simulink model "CONTROL_01"  (R2018b)
(part 37 of 185)

 I4xy*de1 - I4xy*de1*cos(e2)^2 - I4xy*de1*cos(e3)^2 - 2*I4xy*de1*cos(e4)^2 + (I4xx*de1*sin(2*e4))/2 - (I6xx*de1*sin(2*e4))/2 - (I4yy*de1*sin(2*e4))/2 + (I5yy*de1*sin(2*e4))/2 - (I5zz*de1*sin(2*e4))/2 + (I6zz*de1*sin(2*e4))/2 - I6xy*de1*cos(e5) - I5zx*de1*cos(e5) + I5yz*de1*sin(e5) - I5yz*de1*cos(e2)^2*sin(e5) - I5yz*de1*cos(e3)^2*sin(e5) - 2*I5yz*de1*cos(e4)^2*sin(e5) + de1*m4*x4*y4 - (de1*m4*x4^2*sin(2*e4))/2 + (de1*m6*x6^2*sin(2*e4))/2 + (de1*m4*y4^2*sin(2*e4))/2 - (de1*m5*y5^2*sin(2*e4))/2 + (de1*m5*z5^2*sin(2*e4))/2 - (de1*m6*z6^2*sin(2*e4))/2 + 2*I4xy*de1*cos(e2)^2*cos(e3)^2 + 2*I4xy*de1*cos(e2)^2*cos(e4)^2 + 2*I4xy*de1*cos(e3)^2*cos(e4)^2 - (I4xx*de2*cos(e2)*cos(e3))/2 - (I4xx*de3*cos(e2)*cos(e3))/2 - (I5xx*de2*cos(e2)*cos(e3))/2 - (I5xx*de3*cos(e2)*cos(e3))/2 + (I6xx*de2*cos(e2)*cos(e3))/2 + (I6xx*de3*cos(e2)*cos(e3))/2 + (I4yy*de2*cos(e2)*cos(e3))/2 + (I4yy*de3*cos(e2)*cos(e3))/2 - (I5yy*de2*cos(e2)*cos(e3))/2 - (I5yy*de3*cos(e2)*cos(e3))/2 - (I6yy*de2*cos(e2)*cos(e3))/2 - (I6yy*de3*cos(e2)*cos(e3))/2 - (I4zz*de2*cos(e2)*cos(e3))/2 - (I4zz*de3*cos(e2)*cos(e3))/2 + (I5zz*de2*cos(e2)*cos(e3))/2 + (I5zz*de3*cos(e2)*cos(e3))/2 - (I6zz*de2*cos(e2)*cos(e3))/2 - (I6zz*de3*cos(e2)*cos(e3))/2 - I5xy*de5*cos(e2)*sin(e3) - I5xy*de5*cos(e3)*sin(e2) + I6xy*de6*cos(e2)*sin(e3) + I6xy*de6*cos(e3)*sin(e2) - I6yz*de1*cos(e6)*sin(e5) + (I4xx*de2*sin(e2)*sin(e3))/2 + (I4xx*de3*sin(e2)*sin(e3))/2 + (I5xx*de2*sin(e2)*sin(e3))/2 + (I5xx*de3*sin(e2)*sin(e3))/2 - (I6xx*de2*sin(e2)*sin(e3))/2 - (I6xx*de3*sin(e2)*sin(e3))/2 - (I4yy*de2*sin(e2)*sin(e3))/2 - (I4yy*de3*sin(e2)*sin(e3))/2 + (I5yy*de2*sin(e2)*sin(e3))/2 + (I5yy*de3*sin(e2)*sin(e3))/2 + (I6yy*de2*sin(e2)*sin(e3))/2 + (I6yy*de3*sin(e2)*sin(e3))/2 + (I4zz*de2*sin(e2)*sin(e3))/2 + (I4zz*de3*sin(e2)*sin(e3))/2 - (I5zz*de2*sin(e2)*sin(e3))/2 - (I5zz*de3*sin(e2)*sin(e3))/2 + (I6zz*de2*sin(e2)*sin(e3))/2 + (I6zz*de3*sin(e2)*sin(e3))/2 - I6zx*de1*sin(e5)*sin(e6) + I6xy*de1*cos(e2)^2*cos(e5) + I6xy*de1*cos(e3)^2*cos(e5) + 2*I6xy*de1*cos(e4)^2*cos(e5) + 2*I6xy*de1*cos(e5)*cos(e6)^2 + I5zx*de1*cos(e2)^2*cos(e5) + I5zx*de1*cos(e3)^2*cos(e5) + 2*I5zx*de1*cos(e4)^2*cos(e5) - 2*I6xy*de1*cos(e2)^2*cos(e3)^2*cos(e5) - 2*I6xy*de1*cos(e2)^2*cos(e4)^2*cos(e5) - 2*I6xy*de1*cos(e3)^2*cos(e4)^2*cos(e5) - 2*I6xy*de1*cos(e2)^2*cos(e5)*cos(e6)^2 - 2*I6xy*de1*cos(e3)^2*cos(e5)*cos(e6)^2 - 4*I6xy*de1*cos(e4)^2*cos(e5)*cos(e6)^2 - 2*I5zx*de1*cos(e2)^2*cos(e3)^2*cos(e5) - 2*I5zx*de1*cos(e2)^2*cos(e4)^2*cos(e5) - 2*I5zx*de1*cos(e3)^2*cos(e4)^2*cos(e5) + 2*I5yz*de1*cos(e2)^2*cos(e3)^2*sin(e5) + 2*I5yz*de1*cos(e2)^2*cos(e4)^2*sin(e5) + 2*I5yz*de1*cos(e3)^2*cos(e4)^2*sin(e5) - de1*m4*x4*y4*cos(e2)^2 - de1*m4*x4*y4*cos(e3)^2 - 2*de1*m4*x4*y4*cos(e4)^2 - (I5xx*de5*cos(e2)*cos(e3)*cos(e4))/2 - (I6xx*de5*cos(e2)*cos(e3)*cos(e4))/2 + (I5yy*de5*cos(e2)*cos(e3)*cos(e4))/2 - (I6yy*de5*cos(e2)*cos(e3)*cos(e4))/2 - (I5zz*de5*cos(e2)*cos(e3)*cos(e4))/2 + (I6zz*de5*cos(e2)*cos(e3)*cos(e4))/2 - I5xy*de2*cos(e2)*cos(e4)*sin(e3) - I5xy*de2*cos(e3)*cos(e4)*sin(e2) - I5xy*de3*cos(e2)*cos(e4)*sin(e3) - I5xy*de3*cos(e3)*cos(e4)*sin(e2) - I6xx*de1*cos(e5)*cos(e6)*sin(e6) - I4yz*de1*cos(e2)*cos(e4)*sin(e2) - I4yz*de1*cos(e3)*cos(e4)*sin(e3) + I6yy*de1*cos(e5)*cos(e6)*sin(e6) + I4zx*de2*cos(e2)*cos(e4)*sin(e3) + I4zx*de2*cos(e3)*cos(e4)*sin(e2) + I4zx*de3*cos(e2)*cos(e4)*sin(e3) + I4zx*de3*cos(e3)*cos(e4)*sin(e2) - I6zx*de5*cos(e2)*cos(e6)*sin(e3) - I6zx*de5*cos(e3)*cos(e6)*sin(e2) - 4*I4xy*de1*cos(e2)^2*cos(e3)^2*cos(e4)^2 + I5xy*de1*cos(e2)*sin(e2)*sin(e4) + I5xy*de1*cos(e3)*sin(e3)*sin(e4) + (I5xx*de5*cos(e4)*sin(e2)*sin(e3))/2 + (I6xx*de5*cos(e4)*sin(e2)*sin(e3))/2 - I4yz*de2*cos(e2)*sin(e3)*sin(e4) - I4yz*de2*cos(e3)*sin(e2)*sin(e4) - I4yz*de3*cos(e2)*sin(e3)*sin(e4) - I4yz*de3*cos(e3)*sin(e2)*sin(e4) - (I5yy*de5*cos(e4)*sin(e2)*sin(e3))/2 + (I6yy*de5*cos(e4)*sin(e2)*sin(e3))/2 + I6yz*de5*cos(e2)*sin(e3)*sin(e6) + I6yz*de5*cos(e3)*sin(e2)*sin(e6) - I4zx*de1*cos(e2)*sin(e2)*sin(e4) - I4zx*de1*cos(e3)*sin(e3)*sin(e4) + (I5zz*de5*cos(e4)*sin(e2)*sin(e3))/2 - (I6zz*de5*cos(e4)*sin(e2)*sin(e3))/2 - de2*m6*x6^2*cos(e2)*cos(e3) - de3*m6*x6^2*cos(e2)*cos(e3) - de2*m4*y4^2*cos(e2)*cos(e3) - de3*m4*y4^2*cos(e2)*cos(e3) - de2*m5*z5^2*cos(e2)*cos(e3) - de3*m5*z5^2*cos(e2)*cos(e3) + de2*m6*x6^2*sin(e2)*sin(e3) + de3*m6*x6^2*sin(e2)*sin(e3) + de2*m4*y4^2*sin(e2)*sin(e3) + de3*m4*y4^2*sin(e2)*sin(e3) + de2*m5*z5^2*sin(e2)*sin(e3) + de3*m5*z5^2*sin(e2)*sin(e3) + I4xx*de2*cos(e2)*cos(e3)*cos(e4)^2 + I4xx*de3*cos(e2)*cos(e3)*cos(e4)^2 - I6xx*de2*cos(e2)*cos(e3)*cos(e4)^2 - I6xx*de3*cos(e2)*cos(e3)*cos(e4)^2 - I6xx*de2*cos(e2)*cos(e3)*cos(e6)^2 - I6xx*de3*cos(e2)*cos(e3)*cos(e6)^2 - I4yy*de2*cos(e2)*cos(e3)*cos(e4)^2 - I4yy*de3*cos(e2)*cos(e3)*cos(e4)^2 + I5yy*de2*cos(e2)*cos(e3)*cos(e4)^2 + I5yy*de3*cos(e2)*cos(e3)*cos(e4)^2 + I6yy*de2*cos(e2)*cos(e3)*cos(e6)^2 + I6yy*de3*cos(e2)*cos(e3)*cos(e6)^2 - I5zz*de2*cos(e2)*cos(e3)*cos(e4)^2 - I5zz*de3*cos(e2)*cos(e3)*cos(e4)^2 + I6zz*de2*cos(e2)*cos(e3)*cos(e4)^2 + I6zz*de3*cos(e2)*cos(e3)*cos(e4)^2 - I4xx*de1*cos(e2)^2*cos(e4)*sin(e4) - I4xx*de1*cos(e3)^2*cos(e4)*sin(e4) + I6xx*de1*cos(e2)^2*cos(e4)*sin(e4) + I6xx*de1*cos(e3)^2*cos(e4)*sin(e4) + I5xx*de1*cos(e4)*cos(e5)^2*sin(e4) + 2*I5xy*de5*cos(e2)*cos(e5)^2*sin(e3) + 2*I5xy*de5*cos(e3)*cos(e5)^2*sin(e2) + I6xx*de1*cos(e4)*cos(e6)^2*sin(e4) - I6xy*de6*cos(e2)*cos(e5)^2*sin(e3) - I6xy*de6*cos(e3)*cos(e5)^2*sin(e2) - 2*I6xy*de6*cos(e2)*cos(e6)^2*sin(e3) - 2*I6xy*de6*cos(e3)*cos(e6)^2*sin(e2) + I4yy*de1*cos(e2)^2*cos(e4)*sin(e4) + I4yy*de1*cos(e3)^2*cos(e4)*sin(e4) - I5yy*de1*cos(e2)^2*cos(e4)*sin(e4) - I5yy*de1*cos(e3)^2*cos(e4)*sin(e4) - I5yy*de1*cos(e4)*cos(e5)^2*sin(e4) + I6yy*de1*cos(e4)*cos(e5)^2*sin(e4) - I6yy*de1*cos(e4)*cos(e6)^2*sin(e4) + I6yz*de1*cos(e2)^2*cos(e6)*sin(e5) + I6yz*de1*cos(e3)^2*cos(e6)*sin(e5) + 2*I6yz*de1*cos(e4)^2*cos(e6)*sin(e5) + I5zz*de1*cos(e2)^2*cos(e4)*sin(e4) + I5zz*de1*cos(e3)^2*cos(e4)*sin(e4) - I6zz*de1*cos(e2)^2*cos(e4)*sin(e4) - I6zz*de1*cos(e3)^2*cos(e4)*sin(e4) - I6zz*de1*cos(e4)*cos(e5)^2*sin(e4) - I4xx*de2*cos(e4)^2*sin(e2)*sin(e3) - I4xx*de3*cos(e4)^2*sin(e2)*sin(e3) + I6xx*de2*cos(e4)^2*sin(e2)*sin(e3) + I6xx*de3*cos(e4)^2*sin(e2)*sin(e3) + I6xx*de2*cos(e6)^2*sin(e2)*sin(e3) + I6xx*de3*cos(e6)^2*sin(e2)*sin(e3) + I4yy*de2*cos(e4)^2*sin(e2)*sin(e3) + I4yy*de3*cos(e4)^2*sin(e2)*sin(e3) - I5yy*de2*cos(e4)^2*sin(e2)*sin(e3) - I5yy*de3*cos(e4)^2*sin(e2)*sin(e3) - I6yy*de2*cos(e6)^2*sin(e2)*sin(e3) - I6yy*de3*cos(e6)^2*sin(e2)*sin(e3) + I5zz*de2*cos(e4)^2*sin(e2)*sin(e3) + I5zz*de3*cos(e4)^2*sin(e2)*sin(e3) - I6zz*de2*cos(e4)^2*sin(e2)*sin(e3) + I6zx*de1*cos(e2)^2*sin(e5)*sin(e6) - I6zz*de3*cos(e4)^2*sin(e2)*sin(e3) + I6zx*de1*cos(e3)^2*sin(e5)*sin(e6) + 2*I6zx*de1*cos(e4)^2*sin(e5)*sin(e6) - de1*m6*x6*y6*cos(e5) - de1*m5*x5*z5*cos(e5) + de1*m5*y5*z5*sin(e5) + a3*de1*m4*x4*cos(e2)^2*sin(e4) + a3*de1*m4*x4*cos(e3)^2*sin(e4) - I5xx*de2*cos(e4)^2*cos(e5)^2*sin(e2)*sin(e3) - I5xx*de3*cos(e4)^2*cos(e5)^2*sin(e2)*sin(e3) - I6xx*de2*cos(e4)^2*cos(e6)^2*sin(e2)*sin(e3) - I6xx*de3*cos(e4)^2*cos(e6)^2*sin(e2)*sin(e3) + I5yy*de2*cos(e4)^2*cos(e5)^2*sin(e2)*sin(e3) + I5yy*de3*cos(e4)^2*cos(e5)^2*sin(e2)*sin(e3) - I6yy*de2*cos(e4)^2*cos(e5)^2*sin(e2)*sin(e3) + I6yy*de2*cos(e4)^2*cos(e6)^2*sin(e2)*sin(e3) - I6yy*de3*cos(e4)^2*cos(e5)^2*sin(e2)*sin(e3) + I6yy*de3*cos(e4)^2*cos(e6)^2*sin(e2)*sin(e3) - 2*I6zx*de1*cos(e2)^2*cos(e3)^2*sin(e5)*sin(e6) - 2*I6zx*de1*cos(e2)^2*cos(e4)^2*sin(e5)*sin(e6) + I6zz*de2*cos(e4)^2*cos(e5)^2*sin(e2)*sin(e3) - 2*I6zx*de1*cos(e3)^2*cos(e4)^2*sin(e5)*sin(e6) + I6zz*de3*cos(e4)^2*cos(e5)^2*sin(e2)*sin(e3) + de1*m6*x6*y6*cos(e2)^2*cos(e5) + de1*m6*x6*y6*cos(e3)^2*cos(e5) + 2*de1*m6*x6*y6*cos(e4)^2*cos(e5) + 2*de1*m6*x6*y6*cos(e5)*cos(e6)^2 + de1*m5*x5*z5*cos(e2)^2*cos(e5) + de1*m5*x5*z5*cos(e3)^2*cos(e5) + 2*de1*m5*x5*z5*cos(e4)^2*cos(e5) - de1*m5*y5*z5*cos(e2)^2*sin(e5) - de1*m5*y5*z5*cos(e3)^2*sin(e5) - 2*de1*m5*y5*z5*cos(e4)^2*sin(e5) - I6yz*de6*cos(e2)*cos(e3)*cos(e4)*cos(e6) + 2*I4xy*de2*cos(e2)*cos(e3)*cos(e4)*sin(e4) + 2*I4xy*de3*cos(e2)*cos(e3)*cos(e4)*sin(e4) - 2*I6xy*de2*cos(e2)*cos(e3)*cos(e6)*sin(e6) - I6xy*de5*cos(e2)*cos(e3)*cos(e5)*sin(e4) - 2*I6xy*de3*cos(e2)*cos(e3)*cos(e6)*sin(e6) + I5yz*de1*cos(e2)*cos(e4)*cos(e5)*sin(e2) + I5yz*de1*cos(e3)*cos(e4)*cos(e5)*sin(e3) - I6zx*de2*cos(e2)*cos(e4)*cos(e6)*sin(e3) - I6zx*de2*cos(e3)*cos(e4)*cos(e6)*sin(e2) - I5zx*de5*cos(e2)*cos(e3)*cos(e5)*sin(e4) - I6zx*de3*cos(e2)*cos(e4)*cos(e6)*sin(e3) - I6zx*de3*cos(e3)*cos(e4)*cos(e6)*sin(e2) - I6zx*de6*cos(e2)*cos(e3)*cos(e4)*sin(e6) + 4*I6xy*de1*cos(e2)^2*cos(e3)^2*cos(e4)^2*cos(e5) + 4*I6xy*de1*cos(e2)^2*cos(e3)^2*cos(e5)*cos(e6)^2 + 4*I6xy*de1*cos(e2)^2*cos(e4)^2*cos(e5)*cos(e6)^2 + 4*I6xy*de1*cos(e3)^2*cos(e4)^2*cos(e5)*cos(e6)^2 + 4*I5zx*de1*cos(e2)^2*cos(e3)^2*cos(e4)^2*cos(e5) - 2*I4xy*de1*cos(e2)*cos(e3)*sin(e2)*sin(e3) + I6xy*de1*cos(e2)*cos(e4)*sin(e2)*sin(e5) + I6xy*de1*cos(e3)*cos(e4)*sin(e3)*sin(e5) - I5xx*de5*cos(e2)*cos(e5)*sin(e3)*sin(e5) - I5xx*de5*cos(e3)*cos(e5)*sin(e2)*sin(e5) + 2*I5xy*de1*cos(e4)*cos(e5)*sin(e4)*sin(e5) + (I6xx*de6*cos(e2)*cos(e3)*sin(e4)*sin(e5))/2 + 2*I6xy*de1*cos(e4)*cos(e6)*sin(e4)*sin(e6) + I6xx*de6*cos(e2)*cos(e6)*sin(e3)*sin(e6) + I6xx*de6*cos(e3)*cos(e6)*sin(e2)*sin(e6) + I5yz*de2*cos(e2)*cos(e5)*sin(e3)*sin(e4) + I5yz*de2*cos(e3)*cos(e5)*sin(e2)*sin(e4) + I5yz*de3*cos(e2)*cos(e5)*sin(e3)*sin(e4) + I5yz*de3*cos(e3)*cos(e5)*sin(e2)*sin(e4) + I6yz*de2*cos(e2)*cos(e4)*sin(e3)*sin(e6) + I6yz*de2*cos(e3)*cos(e4)*sin(e2)*sin(e6) + I5yy*de5*cos(e2)*cos(e5)*sin(e3)*sin(e5) + I5yy*de5*cos(e3)*cos(e5)*sin(e2)*sin(e5) + I5yz*de5*cos(e2)*cos(e3)*sin(e4)*sin(e5) + I6yz*de3*cos(e2)*cos(e4)*sin(e3)*sin(e6) + I6yz*de3*cos(e3)*cos(e4)*sin(e2)*sin(e6) - I6yy*de5*cos(e2)*cos(e5)*sin(e3)*sin(e5) - I6yy*de5*cos(e3)*cos(e5)*sin(e2)*sin(e5) - (I6yy*de6*cos(e2)*cos(e3)*sin(e4)*sin(e5))/2 + I6yz*de6*cos(e4)*cos(e6)*sin(e2)*sin(e3) - I6yy*de6*cos(e2)*cos(e6)*sin(e3)*sin(e6) - I6yy*de6*cos(e3)*cos(e6)*sin(e2)*sin(e6) + I5zx*de1*cos(e2)*cos(e4)*sin(e2)*sin(e5) + I5zx*de1*cos(e3)*cos(e4)*sin(e3)*sin(e5) + I6zx*de1*cos(e2)*cos(e6)*sin(e2)*sin(e4) + I6zx*de1*cos(e3)*cos(e6)*sin(e3)*sin(e4) + I6zz*de5*cos(e2)*cos(e5)*sin(e3)*sin(e5) + I6zz*de5*cos(e3)*cos(e5)*sin(e2)*sin(e5) - (I6zz*de6*cos(e2)*cos(e3)*sin(e4)*sin(e5))/2 - 4*I5yz*de1*cos(e2)^2*cos(e3)^2*cos(e4)^2*sin(e5) - 2*I4xy*de2*cos(e4)*sin(e2)*sin(e3)*sin(e4) - 2*I4xy*de3*cos(e4)*sin(e2)*sin(e3)*sin(e4) + I6xy*de2*cos(e2)*sin(e3)*sin(e4)*sin(e5) + I6xy*de2*cos(e3)*sin(e2)*sin(e4)*sin(e5) + I6xy*de3*cos(e2)*sin(e3)*sin(e4)*sin(e5) + I6xy*de3*cos(e3)*sin(e2)*sin(e4)*sin(e5) + 2*I6xy*de2*cos(e6)*sin(e2)*sin(e3)*sin(e6) + I6xy*de5*cos(e5)*sin(e2)*sin(e3)*sin(e4) + 2*I6xy*de3*cos(e6)*sin(e2)*sin(e3)*sin(e6) - I6yz*de1*cos(e2)*sin(e2)*sin(e4)*sin(e6) - I6yz*de1*cos(e3)*sin(e3)*sin(e4)*sin(e6) + I5zx*de2*cos(e2)*sin(e3)*sin(e4)*sin(e5) + I5zx*de2*cos(e3)*sin(e2)*sin(e4)*sin(e5) + I5zx*de3*cos(e2)*sin(e3)*sin(e4)*sin(e5) + I5zx*de3*cos(e3)*sin(e2)*sin(e4)*sin(e5) + I5zx*de5*cos(e5)*sin(e2)*sin(e3)*sin(e4) + I6zx*de6*cos(e4)*sin(e2)*sin(e3)*sin(e6) - de5*m5*y5^2*cos(e2)*cos(e3)*cos(e4) - de5*m6*z6^2*cos(e2)*cos(e3)*cos(e4) - (I6xx*de6*sin(e2)*sin(e3)*sin(e4)*sin(e5))/2 - I5yz*de5*sin(e2)*sin(e3)*sin(e4)*sin(e5) + (I6yy*de6*sin(e2)*sin(e3)*sin(e4)*sin(e5))/2 + (I6zz*de6*sin(e2)*sin(e3)*sin(e4)*sin(e5))/2 + de1*m6*x6^2*cos(e5)*cos(e6)*sin(e6) + 2*de1*m4*x4*y4*cos(e2)^2*cos(e3)^2 + 2*de1*m4*x4*y4*cos(e2)^2*cos(e4)^2 + 2*de1*m4*x4*y4*cos(e3)^2*cos(e4)^2 - de1*m6*y6^2*cos(e5)*cos(e6)*sin(e6) + de5*m5*y5^2*cos(e4)*sin(e2)*sin(e3) + de5*m6*z6^2*cos(e4)*sin(e2)*sin(e3) + I5xx*de5*cos(e2)*cos(e3)*cos(e4)*cos(e5)^2 - I5yy*de5*cos(e2)*cos(e3)*cos(e4)*cos(e5)^2 + I6yy*de5*cos(e2)*cos(e3)*cos(e4)*cos(e5)^2 - I6zz*de5*cos(e2)*cos(e3)*cos(e4)*cos(e5)^2 - a2*de2*m4*x4*cos(e2)*cos(e4) + a2*de1*m4*y4*cos(e3)*cos(e4) - a2*de1*m5*z5*cos(e3)*cos(e4) + 2*I5xy*de2*cos(e2)*cos(e4)*cos(e5)^2*sin(e3) + 2*I5xy*de2*cos(e3)*cos(e4)*cos(e5)^2*sin(e2) + 2*I5xy*de3*cos(e2)*cos(e4)*cos(e5)^2*sin(e3) + 2*I5xy*de3*cos(e3)*cos(e4)*cos(e5)^2*sin(e2) + I6xx*de1*cos(e2)^2*cos(e5)*cos(e6)*sin(e6) + I6xx*de1*cos(e3)^2*cos(e5)*cos(e6)*sin(e6) + 2*I6xx*de1*cos(e4)^2*cos(e5)*cos(e6)*sin(e6) + 2*I4yz*de1*cos(e2)*cos(e3)^2*cos(e4)*sin(e2) + 2*I4yz*de1*cos(e2)^2*cos(e3)*cos(e4)*sin(e3) - I6yy*de1*cos(e2)^2*cos(e5)*cos(e6)*sin(e6) - I6yy*de1*cos(e3)^2*cos(e5)*cos(e6)*sin(e6) - 2*I6yy*de1*cos(e4)^2*cos(e5)*cos(e6)*sin(e6) + 2*I6zx*de5*cos(e2)*cos(e5)^2*cos(e6)*sin(e3) + 2*I6zx*de5*cos(e3)*cos(e5)^2*cos(e6)*sin(e2) + a2*de1*m4*x4*cos(e3)*sin(e4) + a2*de2*m4*y4*cos(e2)*sin(e4) - a2*de2*m5*z5*cos(e2)*sin(e4) - 2*I5xy*de1*cos(e2)*cos(e3)^2*sin(e2)*sin(e4) - 2*I5xy*de1*cos(e2)^2*cos(e3)*sin(e3)*sin(e4) - 2*I5xy*de1*cos(e2)*cos(e5)^2*sin(e2)*sin(e4) - 2*I5xy*de1*cos(e3)*cos(e5)^2*sin(e3)*sin(e4) - I5xx*de5*cos(e4)*cos(e5)^2*sin(e2)*sin(e3) + I5yy*de5*cos(e4)*cos(e5)^2*sin(e2)*sin(e3) - I6yy*de5*cos(e4)*cos(e5)^2*sin(e2)*sin(e3) - 2*I6yz*de5*cos(e2)*cos(e5)^2*sin(e3)*sin(e6) - 2*I6yz*de5*cos(e3)*cos(e5)^2*sin(e2)*sin(e6) + 2*I4zx*de1*cos(e2)*cos(e3)^2*sin(e2)*sin(e4) + 2*I4zx*de1*cos(e2)^2*cos(e3)*sin(e3)*sin(e4) + I6zz*de5*cos(e4)*cos(e5)^2*sin(e2)*sin(e3) - de2*m4*x4^2*cos(e2)*cos(e3)*cos(e4)^2 - de3*m4*x4^2*cos(e2)*cos(e3)*cos(e4)^2 + de2*m6*x6^2*cos(e2)*cos(e3)*cos(e4)^2 + de3*m6*x6^2*cos(e2)*cos(e3)*cos(e4)^2 + de2*m6*x6^2*cos(e2)*cos(e3)*cos(e6)^2 + de3*m6*x6^2*cos(e2)*cos(e3)*cos(e6)^2 + de2*m4*y4^2*cos(e2)*cos(e3)*cos(e4)^2 + de3*m4*y4^2*cos(e2)*cos(e3)*cos(e4)^2 - de2*m5*y5^2*cos(e2)*cos(e3)*cos(e4)^2 - de3*m5*y5^2*cos(e2)*cos(e3)*cos(e4)^2 - de2*m6*y6^2*cos(e2)*cos(e3)*cos(e6)^2 - de3*m6*y6^2*cos(e2)*cos(e3)*cos(e6)^2 - de5*m5*x5*y5*cos(e2)*sin(e3) - de5*m5*x5*y5*cos(e3)*sin(e2) + de6*m6*x6*y6*cos(e2)*sin(e3) + de6*m6*x6*y6*cos(e3)*sin(e2) + de2*m5*z5^2*cos(e2)*cos(e3)*cos(e4)^2 + de3*m5*z5^2*cos(e2)*cos(e3)*cos(e4)^2 - de2*m6*z6^2*cos(e2)*cos(e3)*cos(e4)^2 - de3*m6*z6^2*cos(e2)*cos(e3)*cos(e4)^2 - de1*m6*y6*z6*cos(e6)*sin(e5) + de1*m4*x4^2*cos(e2)^2*cos(e4)*sin(e4) + de1*m4*x4^2*cos(e3)^2*cos(e4)*sin(e4) - de1*m6*x6^2*cos(e2)^2*cos(e4)*sin(e4) - de1*m5*x5^2*cos(e4)*cos(e5)^2*sin(e4) - de1*m6*x6^2*cos(e3)^2*cos(e4)*sin(e4) - de1*m6*x6^2*cos(e4)*cos(e6)^2*sin(e4) - de1*m4*y4^2*cos(e2)^2*cos(e4)*sin(e4) - de1*m4*y4^2*cos(e3)^2*cos(e4)*sin(e4) + de1*m5*y5^2*cos(e2)^2*cos(e4)*sin(e4) + de1*m5*y5^2*cos(e3)^2*cos(e4)*sin(e4) + de1*m5*y5^2*cos(e4)*cos(e5)^2*sin(e4) - de1*m6*y6^2*cos(e4)*cos(e5)^2*sin(e4) + de1*m6*y6^2*cos(e4)*cos(e6)^2*sin(e4) - de1*m5*z5^2*cos(e2)^2*cos(e4)*sin(e4) - de1*m5*z5^2*cos(e3)^2*cos(e4)*sin(e4) + de1*m6*z6^2*cos(e2)^2*cos(e4)*sin(e4) + de1*m6*z6^2*cos(e3)^2*cos(e4)*sin(e4) + de1*m6*z6^2*cos(e4)*cos(e5)^2*sin(e4) - de1*m6*x6*z6*sin(e5)*sin(e6) + de2*m4*x4^2*cos(e4)^2*sin(e2)*sin(e3) + de3*m4*x4^2*cos(e4)^2*sin(e2)*sin(e3) - de2*m6*x6^2*cos(e4)^2*sin(e2)*sin(e3) - de3*m6*x6^2*cos(e4)^2*sin(e2)*sin(e3) - de2*m6*x6^2*cos(e6)^2*sin(e2)*sin(e3) - de3*m6*x6^2*cos(e6)^2*sin(e2)*sin(e3) - de2*m4*y4^2*cos(e4)^2*sin(e2)*sin(e3) - de3*m4*y4^2*cos(e4)^2*sin(e2)*sin(e3) + de2*m5*y5^2*cos(e4)^2*sin(e2)*sin(e3) + de3*m5*y5^2*cos(e4)^2*sin(e2)*sin(e3) + de2*m6*y6^2*cos(e6)^2*sin(e2)*sin(e3) + de3*m6*y6^2*cos(e6)^2*sin(e2)*sin(e3) - de2*m5*z5^2*cos(e4)^2*sin(e2)*sin(e3) - de3*m5*z5^2*cos(e4)^2*sin(e2)*sin(e3) + de2*m6*z6^2*cos(e4)^2*sin(e2)*sin(e3) + de3*m6*z6^2*cos(e4)^2*sin(e2)*sin(e3) + I5xx*de2*cos(e2)*cos(e3)*cos(e4)^2*cos(e5)^2 + I5xx*de3*cos(e2)*cos(e3)*cos(e4)^2*cos(e5)^2 + I6xx*de2*cos(e2)*cos(e3)*cos(e4)^2*cos(e6)^2 + I6xx*de3*cos(e2)*cos(e3)*cos(e4)^2*cos(e6)^2 - I5yy*de2*cos(e2)*cos(e3)*cos(e4)^2*cos(e5)^2 - I5yy*de3*cos(e2)*cos(e3)*cos(e4)^2*cos(e5)^2 + I6yy*de2*cos(e2)*cos(e3)*cos(e4)^2*cos(e5)^2 - I6yy*de2*cos(e2)*cos(e3)*cos(e4)^2*cos(e6)^2 + I6yy*de3*cos(e2)*cos(e3)*cos(e4)^2*cos(e5)^2 - I6yy*de3*cos(e2)*cos(e3)*cos(e4)^2*cos(e6)^2 - I6zz*de2*cos(e2)*cos(e3)*cos(e4)^2*cos(e5)^2 - I6zz*de3*cos(e2)*cos(e3)*cos(e4)^2*cos(e5)^2 + a3*de1*m4*y4*cos(e2)^2*cos(e4) + a3*de1*m4*y4*cos(e3)^2*cos(e4) - a3*de1*m5*z5*cos(e2)^2*cos(e4) - a3*de1*m5*z5*cos(e3)^2*cos(e4) + 2*I4xx*de1*cos(e2)^2*cos(e3)^2*cos(e4)*sin(e4) - 2*I6xx*de1*cos(e2)^2*cos(e3)^2*cos(e4)*sin(e4) - I5xx*de1*cos(e2)^2*cos(e4)*cos(e5)^2*sin(e4) - I5xx*de1*cos(e3)^2*cos(e4)*cos(e5)^2*sin(e4) - I6xx*de1*cos(e2)^2*cos(e4)*cos(e6)^2*sin(e4) - I6xx*de1*cos(e3)^2*cos(e4)*cos(e6)^2*sin(e4) + I6xx*de1*cos(e4)*cos(e5)^2*cos(e6)^2*sin(e4) + 2*I6xy*de6*cos(e2)*cos(e5)^2*cos(e6)^2*sin(e3) + 2*I6xy*de6*cos(e3)*cos(e5)^2*cos(e6)^2*sin(e2) - 2*I4yy*de1*cos(e2)^2*cos(e3)^2*cos(e4)*sin(e4) + 2*I5yy*de1*cos(e2)^2*cos(e3)^2*cos(e4)*sin(e4) + I5yy*de1*cos(e2)^2*cos(e4)*cos(e5)^2*sin(e4) + I5yy*de1*cos(e3)^2*cos(e4)*cos(e5)^2*sin(e4) - I6yy*de1*cos(e2)^2*cos(e4)*cos(e5)^2*sin(e4) + I6yy*de1*cos(e2)^2*cos(e4)*cos(e6)^2*sin(e4) - I6yy*de1*cos(e3)^2*cos(e4)*cos(e5)^2*sin(e4) + I6yy*de1*cos(e3)^2*cos(e4)*cos(e6)^2*sin(e4) - 2*I6yz*de1*cos(e2)^2*cos(e3)^2*cos(e6)*sin(e5) - 2*I6yz*de1*cos(e2)^2*cos(e4)^2*cos(e6)*sin(e5) - I6yy*de1*cos(e4)*cos(e5)^2*cos(e6)^2*sin(e4) - 2*I6yz*de1*cos(e3)^2*cos(e4)^2*cos(e6)*sin(e5) - 2*I5zz*de1*cos(e2)^2*cos(e3)^2*cos(e4)*sin(e4) + 2*I6zz*de1*cos(e2)^2*cos(e3)^2*cos(e4)*sin(e4) + I6zz*de1*cos(e2)^2*cos(e4)*cos(e5)^2*sin(e4) + I6zz*de1*cos(e3)^2*cos(e4)*cos(e5)^2*sin(e4) - 2*I6xy*de2*cos(e2)*cos(e3)*cos(e4)*cos(e5)*sin(e4) - 2*I6xy*de3*cos(e2)*cos(e3)*cos(e4)*cos(e5)*sin(e4) + 2*I5xy*de5*cos(e2)*cos(e3)*cos(e4)*cos(e5)*sin(e5) - I6xy*de6*cos(e2)*cos(e3)*cos(e4)*cos(e5)*sin(e5) - I6yz*de1*cos(e2)*cos(e4)*cos(e5)*cos(e6)*sin(e2) - I6yz*de1*cos(e3)*cos(e4)*cos(e5)*cos(e6)*sin(e3) - 2*I5zx*de2*cos(e2)*cos(e3)*cos(e4)*cos(e5)*sin(e4) - 2*I5zx*de3*cos(e2)*cos(e3)*cos(e4)*cos(e5)*sin(e4) + de2*m5*x5^2*cos(e4)^2*cos(e5)^2*sin(e2)*sin(e3) + de3*m5*x5^2*cos(e4)^2*cos(e5)^2*sin(e2)*sin(e3) + de2*m6*x6^2*cos(e4)^2*cos(e6)^2*sin(e2)*sin(e3) + de3*m6*x6^2*cos(e4)^2*cos(e6)^2*sin(e2)*sin(e3) - de2*m5*y5^2*cos(e4)^2*cos(e5)^2*sin(e2)*sin(e3) - de3*m5*y5^2*cos(e4)^2*cos(e5)^2*sin(e2)*sin(e3) + de2*m6*y6^2*cos(e4)^2*cos(e5)^2*sin(e2)*sin(e3) - de2*m6*y6^2*cos(e4)^2*cos(e6)^2*sin(e2)*sin(e3) + de3*m6*y6^2*cos(e4)^2*cos(e5)^2*sin(e2)*sin(e3) - de3*m6*y6^2*cos(e4)^2*cos(e6)^2*sin(e2)*sin(e3) - de2*m6*z6^2*cos(e4)^2*cos(e5)^2*sin(e2)*sin(e3) - de3*m6*z6^2*cos(e4)^2*cos(e5)^2*sin(e2)*sin(e3) + I6xx*de2*cos(e2)*cos(e3)*cos(e4)^2*cos(e5)^2*cos(e6)^2 + I6xx*de3*cos(e2)*cos(e3)*cos(e4)^2*cos(e5)^2*cos(e6)^2 - I6yy*de2*cos(e2)*cos(e3)*cos(e4)^2*cos(e5)^2*cos(e6)^2 - I6yy*de3*cos(e2)*cos(e3)*cos(e4)^2*cos(e5)^2*cos(e6)^2 + 2*I6xy*de1*cos(e2)*cos(e3)*cos(e5)*sin(e2)*sin(e3) - I5xx*de2*cos(e2)*cos(e4)*cos(e5)*sin(e3)*sin(e5) - I5xx*de2*cos(e3)*cos(e4)*cos(e5)*sin(e2)*sin(e5) - I5xx*de3*cos(e2)*cos(e4)*cos(e5)*sin(e3)*sin(e5) - I5xx*de3*cos(e3)*cos(e4)*cos(e5)*sin(e2)*sin(e5) + I5yy*de2*cos(e2)*cos(e4)*cos(e5)*sin(e3)*sin(e5) + I5yy*de2*cos(e3)*cos(e4)*cos(e5)*sin(e2)*sin(e5) + 2*I5yz*de2*cos(e2)*cos(e3)*cos(e4)*sin(e4)*sin(e5) + I5yy*de3*cos(e2)*cos(e4)*cos(e5)*sin(e3)*sin(e5) + I5yy*de3*cos(e3)*cos(e4)*cos(e5)*sin(e2)*sin(e5) + 2*I5yz*de3*cos(e2)*cos(e3)*cos(e4)*sin(e4)*sin(e5) - I6yy*de2*cos(e2)*cos(e4)*cos(e5)*sin(e3)*sin(e5) - I6yy*de2*cos(e3)*cos(e4)*cos(e5)*sin(e2)*sin(e5) - I6yy*de3*cos(e2)*cos(e4)*cos(e5)*sin(e3)*sin(e5) - I6yy*de3*cos(e3)*cos(e4)*cos(e5)*sin(e2)*sin(e5) - I6yz*de2*cos(e2)*cos(e5)*cos(e6)*sin(e3)*sin(e4) - I6yz*de2*cos(e3)*cos(e5)*cos(e6)*sin(e2)*sin(e4) - I6yz*de3*cos(e2)*cos(e5)*cos(e6)*sin(e3)*sin(e4) - I6yz*de3*cos(e3)*cos(e5)*cos(e6)*sin(e2)*sin(e4) - I6yz*de5*cos(e2)*cos(e3)*cos(e6)*sin(e4)*sin(e5) - I6yz*de6*cos(e2)*cos(e5)*cos(e6)*sin(e3)*sin(e5) - I6yz*de6*cos(e3)*cos(e5)*cos(e6)*sin(e2)*sin(e5) + 2*I5zx*de1*cos(e2)*cos(e3)*cos(e5)*sin(e2)*sin(e3) - I6zx*de1*cos(e2)*cos(e4)*cos(e5)*sin(e2)*sin(e6) - I6zx*de1*cos(e3)*cos(e4)*cos(e5)*sin(e3)*sin(e6) + I6zz*de2*cos(e2)*cos(e4)*cos(e5)*sin(e3)*sin(e5) + I6zz*de2*cos(e3)*cos(e4)*cos(e5)*sin(e2)*sin(e5) + I6zz*de3*cos(e2)*cos(e4)*cos(e5)*sin(e3)*sin(e5) + I6zz*de3*cos(e3)*cos(e4)*cos(e5)*sin(e2)*sin(e5) + 2*I6zx*de1*cos(e4)*cos(e5)*cos(e6)*sin(e4)*sin(e5) - 2*a3*de1*m4*y4*cos(e2)^2*cos(e3)^2*cos(e4) + 2*a3*de1*m5*z5*cos(e2)^2*cos(e3)^2*cos(e4) + 2*I5xx*de1*cos(e2)^2*cos(e3)^2*cos(e4)*cos(e5)^2*sin(e4) + 2*I6xx*de1*cos(e2)^2*cos(e3)^2*cos(e4)*cos(e6)^2*sin(e4) - I6xx*de1*cos(e2)^2*cos(e4)*cos(e5)^2*cos(e6)^2*sin(e4) - I6xx*de1*cos(e3)^2*cos(e4)*cos(e5)^2*cos(e6)^2*sin(e4) - 2*I5yy*de1*cos(e2)^2*cos(e3)^2*cos(e4)*cos(e5)^2*sin(e4) + 2*I6yy*de1*cos(e2)^2*cos(e3)^2*cos(e4)*cos(e5)^2*sin(e4) - 2*I6yy*de1*cos(e2)^2*cos(e3)^2*cos(e4)*cos(e6)^2*sin(e4) + I6yy*de1*cos(e2)^2*cos(e4)*cos(e5)^2*cos(e6)^2*sin(e4) + 4*I6yz*de1*cos(e2)^2*cos(e3)^2*cos(e4)^2*cos(e6)*sin(e5) + I6yy*de1*cos(e3)^2*cos(e4)*cos(e5)^2*cos(e6)^2*sin(e4) - 2*I6zz*de1*cos(e2)^2*cos(e3)^2*cos(e4)*cos(e5)^2*sin(e4) + I5xx*de1*cos(e2)*cos(e5)*sin(e2)*sin(e4)*sin(e5) + I5xx*de1*cos(e3)*cos(e5)*sin(e3)*sin(e4)*sin(e5) + 2*I6xy*de2*cos(e4)*cos(e5)*sin(e2)*sin(e3)*sin(e4) + 2*I6xy*de3*cos(e4)*cos(e5)*sin(e2)*sin(e3)*sin(e4) - 2*I5xy*de5*cos(e4)*cos(e5)*sin(e2)*sin(e3)*sin(e5) + I6xy*de6*cos(e4)*cos(e5)*sin(e2)*sin(e3)*sin(e5) - 2*I5yz*de1*cos(e2)*cos(e3)*sin(e2)*sin(e3)*sin(e5) - I5yy*de1*cos(e2)*cos(e5)*sin(e2)*sin(e4)*sin(e5) + I6yy*de1*cos(e2)*cos(e5)*sin(e2)*sin(e4)*sin(e5) - I5yy*de1*cos(e3)*cos(e5)*sin(e3)*sin(e4)*sin(e5) + I6yy*de1*cos(e3)*cos(e5)*sin(e3)*sin(e4)*sin(e5) - 2*I6yz*de1*cos(e4)*cos(e5)*sin(e4)*sin(e5)*sin(e6) + 2*I5zx*de2*cos(e4)*cos(e5)*sin(e2)*sin(e3)*sin(e4) + 2*I5zx*de3*cos(e4)*cos(e5)*sin(e2)*sin(e3)*sin(e4) - I6zz*de1*cos(e2)*cos(e5)*sin(e2)*sin(e4)*sin(e5) - I6zx*de2*cos(e2)*cos(e5)*sin(e3)*sin(e4)*sin(e6) - I6zx*de2*cos(e3)*cos(e5)*sin(e2)*sin(e4)*sin(e6) - I6zx*de3*cos(e2)*cos(e5)*sin(e3)*sin(e4)*sin(e6) - I6zx*de3*cos(e3)*cos(e5)*sin(e2)*sin(e4)*sin(e6) - I6zz*de1*cos(e3)*cos(e5)*sin(e3)*sin(e4)*sin(e5) - I6zx*de5*cos(e2)*cos(e3)*sin(e4)*sin(e5)*sin(e6) - I6zx*de6*cos(e2)*cos(e5)*sin(e3)*sin(e5)*sin(e6) - I6zx*de6*cos(e3)*cos(e5)*sin(e2)*sin(e5)*sin(e6) - 2*a3*de1*m4*x4*cos(e2)^2*cos(e3)^2*sin(e4) - I6xx*de2*cos(e4)^2*cos(e5)^2*cos(e6)^2*sin(e2)*sin(e3) - I6xx*de3*cos(e4)^2*cos(e5)^2*cos(e6)^2*sin(e2)*sin(e3) + I6yy*de2*cos(e4)^2*cos(e5)^2*cos(e6)^2*sin(e2)*sin(e3) + I6yy*de3*cos(e4)^2*cos(e5)^2*cos(e6)^2*sin(e2)*sin(e3) + 4*I6zx*de1*cos(e2)^2*cos(e3)^2*cos(e4)^2*sin(e5)*sin(e6) - 2*I5yz*de2*cos(e4)*sin(e2)*sin(e3)*sin(e4)*sin(e5) - 2*I5yz*de3*cos(e4)*sin(e2)*sin(e3)*sin(e4)*sin(e5) + I6yz*de5*cos(e6)*sin(e2)*sin(e3)*sin(e4)*sin(e5) - 2*de1*m6*x6*y6*cos(e2)^2*cos(e3)^2*cos(e5) - 2*de1*m6*x6*y6*cos(e2)^2*cos(e4)^2*cos(e5) - 2*de1*m6*x6*y6*cos(e3)^2*cos(e4)^2*cos(e5) - 2*de1*m6*x6*y6*cos(e2)^2*cos(e5)*cos(e6)^2 - 2*de1*m6*x6*y6*cos(e3)^2*cos(e5)*cos(e6)^2 - 4*de1*m6*x6*y6*cos(e4)^2*cos(e5)*cos(e6)^2 - 2*de1*m5*x5*z5*cos(e2)^2*cos(e3)^2*cos(e5) - 2*de1*m5*x5*z5*cos(e2)^2*cos(e4)^2*cos(e5) - 2*de1*m5*x5*z5*cos(e3)^2*cos(e4)^2*cos(e5) + I6zx*de5*sin(e2)*sin(e3)*sin(e4)*sin(e5)*sin(e6) + de5*m5*x5^2*cos(e2)*cos(e5)*sin(e3)*sin(e5) + de5*m5*x5^2*cos(e3)*cos(e5)*sin(e2)*sin(e5) - de6*m6*x6^2*cos(e2)*cos(e3)*sin(e4)*sin(e5) - de6*m6*x6^2*cos(e2)*cos(e6)*sin(e3)*sin(e6) - de6*m6*x6^2*cos(e3)*cos(e6)*sin(e2)*sin(e6) - de5*m5*y5^2*cos(e2)*cos(e5)*sin(e3)*sin(e5) - de5*m5*y5^2*cos(e3)*cos(e5)*sin(e2)*sin(e5) + de5*m6*y6^2*cos(e2)*cos(e5)*sin(e3)*sin(e5) + de5*m6*y6^2*cos(e3)*cos(e5)*sin(e2)*sin(e5) + de6*m6*y6^2*cos(e2)*cos(e6)*sin(e3)*sin(e6) + de6*m6*y6^2*cos(e3)*cos(e6)*sin(e2)*sin(e6) - de5*m6*z6^2*cos(e2)*cos(e5)*sin(e3)*sin(e5) - de5*m6*z6^2*cos(e3)*cos(e5)*sin(e2)*sin(e5) + 2*de1*m5*y5*z5*cos(e2)^2*cos(e3)^2*sin(e5) + 2*de1*m5*y5*z5*cos(e2)^2*cos(e4)^2*sin(e5) + 2*de1*m5*y5*z5*cos(e3)^2*cos(e4)^2*sin(e5) + I6yz*de6*cos(e2)*cos(e3)*cos(e4)*cos(e5)^2*cos(e6) - a3*de2*m4*x4*cos(e2)*cos(e3)*cos(e4) - a3*de3*m4*x4*cos(e2)*cos(e3)*cos(e4) - a2*de2*m5*x5*cos(e2)*cos(e4)*cos(e5) + a2*de1*m6*y6*cos(e3)*cos(e4)*cos(e6) + 2*I5xy*de2*cos(e2)*cos(e3)*cos(e4)^2*cos(e5)*sin(e5) + 2*I5xy*de3*cos(e2)*cos(e3)*cos(e4)^2*cos(e5)*sin(e5) + 2*I6xy*de2*cos(e2)*cos(e3)*cos(e4)^2*cos(e6)*sin(e6) + 2*I6xy*de3*cos(e2)*cos(e3)*cos(e4)^2*cos(e6)*sin(e6) + 2*I6xy*de5*cos(e2)*cos(e3)*cos(e5)*cos(e6)^2*sin(e4) - 2*I5yz*de1*cos(e2)*cos(e3)^2*cos(e4)*cos(e5)*sin(e2) - 2*I5yz*de1*cos(e2)^2*cos(e3)*cos(e4)*cos(e5)*sin(e3) + 2*I6zx*de2*cos(e2)*cos(e4)*cos(e5)^2*cos(e6)*sin(e3) + 2*I6zx*de2*cos(e3)*cos(e4)*cos(e5)^2*cos(e6)*sin(e2) + 2*I6zx*de3*cos(e2)*cos(e4)*cos(e5)^2*cos(e6)*sin(e3) + 2*I6zx*de3*cos(e3)*cos(e4)*cos(e5)^2*cos(e6)*sin(e2) + I6zx*de6*cos(e2)*cos(e3)*cos(e4)*cos(e5)^2*sin(e6) + de6*m6*x6^2*sin(e2)*sin(e3)*sin(e4)*sin(e5) + a2*de1*m5*x5*cos(e3)*cos(e5)*sin(e4) + a2*de1*m6*x6*cos(e3)*cos(e4)*sin(e6) + a1*de1*m4*y4*cos(e2)*cos(e4)*sin(e3) + a1*de1*m4*y4*cos(e3)*cos(e4)*sin(e2) + a3*de2*m4*y4*cos(e2)*cos(e3)*sin(e4) + a3*de3*m4*y4*cos(e2)*cos(e3)*sin(e4) + a2*de2*m5*y5*cos(e2)*cos(e4)*sin(e5) + a2*de2*m6*y6*cos(e2)*cos(e6)*sin(e4) - 8*I6xy*de1*cos(e2)^2*cos(e3)^2*cos(e4)^2*cos(e5)*cos(e6)^2 - a1*de1*m5*z5*cos(e2)*cos(e4)*sin(e3) - a1*de1*m5*z5*cos(e3)*cos(e4)*sin(e2) - a3*de2*m5*z5*cos(e2)*cos(e3)*sin(e4) - a3*de3*m5*z5*cos(e2)*cos(e3)*sin(e4) + a2*de2*m6*z6*cos(e2)*cos(e4)*sin(e5) + d4*de2*m4*x4*cos(e2)*cos(e4)*sin(e3) + d4*de2*m4*x4*cos(e3)*cos(e4)*sin(e2) + d4*de3*m4*x4*cos(e2)*cos(e4)*sin(e3) + d4*de3*m4*x4*cos(e3)*cos(e4)*sin(e2) + 4*I4xy*de1*cos(e2)*cos(e3)*cos(e4)^2*sin(e2)*sin(e3) - 2*I6xy*de1*cos(e2)*cos(e3)^2*cos(e4)*sin(e2)*sin(e5) - 2*I6xy*de1*cos(e2)^2*cos(e3)*cos(e4)*sin(e3)*sin(e5) - 2*I5xy*de1*cos(e2)^2*cos(e4)*cos(e5)*sin(e4)*sin(e5) - 2*I6xy*de1*cos(e2)*cos(e4)*cos(e6)^2*sin(e2)*sin(e5) - 2*I5xy*de1*cos(e3)^2*cos(e4)*cos(e5)*sin(e4)*sin(e5) - 2*I6xy*de1*cos(e3)*cos(e4)*cos(e6)^2*sin(e3)*sin(e5) - 2*I6xy*de1*cos(e2)^2*cos(e4)*cos(e6)*sin(e4)*sin(e6) - 2*I6xy*de1*cos(e3)^2*cos(e4)*cos(e6)*sin(e4)*sin(e6) - I6xx*de5*cos(e2)*cos(e5)*cos(e6)^2*sin(e3)*sin(e5) - I6xx*de5*cos(e3)*cos(e5)*cos(e6)^2*sin(e2)*sin(e5) - I6xx*de6*cos(e2)*cos(e3)*cos(e6)^2*sin(e4)*sin(e5) + 2*I6xy*de1*cos(e4)*cos(e5)^2*cos(e6)*sin(e4)*sin(e6) - I6xx*de6*cos(e2)*cos(e5)^2*cos(e6)*sin(e3)*sin(e6) - I6xx*de6*cos(e3)*cos(e5)^2*cos(e6)*sin(e2)*sin(e6) - 2*I6yz*de2*cos(e2)*cos(e4)*cos(e5)^2*sin(e3)*sin(e6) - 2*I6yz*de2*cos(e3)*cos(e4)*cos(e5)^2*sin(e2)*sin(e6) - 2*I6yz*de3*cos(e2)*cos(e4)*cos(e5)^2*sin(e3)*sin(e6) - 2*I6yz*de3*cos(e3)*cos(e4)*cos(e5)^2*sin(e2)*sin(e6) + I6yy*de5*cos(e2)*cos(e5)*cos(e6)^2*sin(e3)*sin(e5) + I6yy*de5*cos(e3)*cos(e5)*cos(e6)^2*sin(e2)*sin(e5) + I6yy*de6*cos(e2)*cos(e3)*cos(e6)^2*sin(e4)*sin(e5) - I6yz*de6*cos(e4)*cos(e5)^2*cos(e6)*sin(e2)*sin(e3) + I6yy*de6*cos(e2)*cos(e5)^2*cos(e6)*sin(e3)*sin(e6) + I6yy*de6*cos(e3)*cos(e5)^2*cos(e6)*sin(e2)*sin(e6) - 2*I5zx*de1*cos(e2)*cos(e3)^2*cos(e4)*sin(e2)*sin(e5) - 2*I5zx*de1*cos(e2)^2*cos(e3)*cos(e4)*sin(e3)*sin(e5) - 2*I6zx*de1*cos(e2)*cos(e3)^2*cos(e6)*sin(e2)*sin(e4) - 2*I6zx*de1*cos(e2)^2*cos(e3)*cos(e6)*sin(e3)*sin(e4) - 2*I6zx*de1*cos(e2)*cos(e5)^2*cos(e6)*sin(e2)*sin(e4) - 2*I6zx*de1*cos(e3)*cos(e5)^2*cos(e6)*sin(e3)*sin(e4) - d4*de1*m4*y4*cos(e2)*cos(e4)*sin(e2) - d4*de1*m4*y4*cos(e3)*cos(e4)*sin(e3) + d4*de1*m5*z5*cos(e2)*cos(e4)*sin(e2) + d4*de1*m5*z5*cos(e3)*cos(e4)*sin(e3) + a1*de1*m4*x4*cos(e2)*sin(e3)*sin(e4) + a1*de1*m4*x4*cos(e3)*sin(e2)*sin(e4) + a3*de2*m4*x4*cos(e4)*sin(e2)*sin(e3) + a3*de3*m4*x4*cos(e4)*sin(e2)*sin(e3) + a2*de2*m6*x6*cos(e2)*sin(e4)*sin(e6) - a2*de1*m5*y5*cos(e3)*sin(e4)*sin(e5) - a2*de1*m6*z6*cos(e3)*sin(e4)*sin(e5) - d4*de1*m4*x4*cos(e2)*sin(e2)*sin(e4) - d4*de1*m4*x4*cos(e3)*sin(e3)*sin(e4) - 2*I5xy*de2*cos(e4)^2*cos(e5)*sin(e2)*sin(e3)*sin(e5) - 2*I5xy*de3*cos(e4)^2*cos(e5)*sin(e2)*sin(e3)*sin(e5) - 2*I6xy*de2*cos(e2)*cos(e6)^2*sin(e3)*sin(e4)*sin(e5) - 2*I6xy*de2*cos(e3)*cos(e6)^2*sin(e2)*sin(e4)*sin(e5) - 2*I6xy*de2*cos(e4)^2*cos(e6)*sin(e2)*sin(e3)*sin(e6) - 2*I6xy*de3*cos(e2)*cos(e6)^2*sin(e3)*sin(e4)*sin(e5) - 2*I6xy*de3*cos(e3)*cos(e6)^2*sin(e2)*sin(e4)*sin(e5) - 2*I6xy*de3*cos(e4)^2*cos(e6)*sin(e2)*sin(e3)*sin(e6) - 2*I6xy*de5*cos(e5)*cos(e6)^2*sin(e2)*sin(e3)*sin(e4) + 2*I6yz*de1*cos(e2)*cos(e3)^2*sin(e2)*sin(e4)*sin(e6) + 2*I6yz*de1*cos(e2)^2*cos(e3)*sin(e3)*sin(e4)*sin(e6) + 2*I6yz*de1*cos(e2)*cos(e5)^2*sin(e2)*sin(e4)*sin(e6) + 2*I6yz*de1*cos(e3)*cos(e5)^2*sin(e3)*sin(e4)*sin(e6) - I6zx*de6*cos(e4)*cos(e5)^2*sin(e2)*sin(e3)*sin(e6) - d4*de2*m4*y4*cos(e2)*sin(e3)*sin(e4) - d4*de2*m4*y4*cos(e3)*sin(e2)*sin(e4) - d4*de3*m4*y4*cos(e2)*sin(e3)*sin(e4) - d4*de3*m4*y4*cos(e3)*sin(e2)*sin(e4) + d4*de2*m5*z5*cos(e2)*sin(e3)*sin(e4) + d4*de2*m5*z5*cos(e3)*sin(e2)*sin(e4) + d4*de3*m5*z5*cos(e2)*sin(e3)*sin(e4) + d4*de3*m5*z5*cos(e3)*sin(e2)*sin(e4) - de5*m5*x5^2*cos(e2)*cos(e3)*cos(e4)*cos(e5)^2 + de5*m5*y5^2*cos(e2)*cos(e3)*cos(e4)*cos(e5)^2 - de5*m6*y6^2*cos(e2)*cos(e3)*cos(e4)*cos(e5)^2 - de2*m5*x5*y5*cos(e2)*cos(e4)*sin(e3) - de2*m5*x5*y5*cos(e3)*cos(e4)*sin(e2) - de3*m5*x5*y5*cos(e2)*cos(e4)*sin(e3) - de3*m5*x5*y5*cos(e3)*cos(e4)*sin(e2) + de5*m6*z6^2*cos(e2)*cos(e3)*cos(e4)*cos(e5)^2 + de2*m4*x4*z4*cos(e2)*cos(e4)*sin(e3) + de2*m4*x4*z4*cos(e3)*cos(e4)*sin(e2) + de3*m4*x4*z4*cos(e2)*cos(e4)*sin(e3) + de3*m4*x4*z4*cos(e3)*cos(e4)*sin(e2) - de5*m6*x6*z6*cos(e2)*cos(e6)*sin(e3) - de5*m6*x6*z6*cos(e3)*cos(e6)*sin(e2) - de1*m4*y4*z4*cos(e2)*cos(e4)*sin(e2) - de1*m4*y4*z4*cos(e3)*cos(e4)*sin(e3) - a3*de2*m4*y4*sin(e2)*sin(e3)*sin(e4) - a3*de3*m4*y4*sin(e2)*sin(e3)*sin(e4) + a3*de2*m5*z5*sin(e2)*sin(e3)*sin(e4) + a3*de3*m5*z5*sin(e2)*sin(e3)*sin(e4) + I6xx*de6*cos(e6)^2*sin(e2)*sin(e3)*sin(e4)*sin(e5) - I6yy*de6*cos(e6)^2*sin(e2)*sin(e3)*sin(e4)*sin(e5) - de1*m6*x6^2*cos(e2)^2*cos(e5)*cos(e6)*sin(e6) - de1*m6*x6^2*cos(e3)^2*cos(e5)*cos(e6)*sin(e6) - 2*de1*m6*x6^2*cos(e4)^2*cos(e5)*cos(e6)*sin(e6) - 4*de1*m4*x4*y4*cos(e2)^2*cos(e3)^2*cos(e4)^2 + de1*m6*y6^2*cos(e2)^2*cos(e5)*cos(e6)*sin(e6) + de1*m6*y6^2*cos(e3)^2*cos(e5)*cos(e6)*sin(e6) + 2*de1*m6*y6^2*cos(e4)^2*cos(e5)*cos(e6)*sin(e6) + de1*m5*x5*y5*cos(e2)*sin(e2)*sin(e4) + de1*m5*x5*y5*cos(e3)*sin(e3)*sin(e4) - de1*m4*x4*z4*cos(e2)*sin(e2)*sin(e4) - de1*m4*x4*z4*cos(e3)*sin(e3)*sin(e4) - de2*m4*y4*z4*cos(e2)*sin(e3)*sin(e4) - de2*m4*y4*z4*cos(e3)*sin(e2)*sin(e4) - de3*m4*y4*z4*cos(e2)*sin(e3)*sin(e4) - de3*m4*y4*z4*cos(e3)*sin(e2)*sin(e4) + de5*m6*y6*z6*cos(e2)*sin(e3)*sin(e6) + de5*m6*y6*z6*cos(e3)*sin(e2)*sin(e6) + de5*m5*x5^2*cos(e4)*cos(e5)^2*sin(e2)*sin(e3) - de5*m5*y5^2*cos(e4)*cos(e5)^2*sin(e2)*sin(e3) + de5*m6*y6^2*cos(e4)*cos(e5)^2*sin(e2)*sin(e3) - de5*m6*z6^2*cos(e4)*cos(e5)^2*sin(e2)*sin(e3) + I6xx*de5*cos(e2)*cos(e3)*cos(e4)*cos(e5)^2*cos(e6)^2 - I6yy*de5*cos(e2)*cos(e3)*cos(e4)*cos(e5)^2*cos(e6)^2 - a2*de1*m4*y4*cos(e2)^2*cos(e3)*cos(e4) + a3*de1*m6*y6*cos(e2)^2*cos(e4)*cos(e6) + a3*de1*m6*y6*cos(e3)^2*cos(e4)*cos(e6) + a2*de1*m5*z5*cos(e2)^2*cos(e3)*cos(e4) - 2*I6xx*de1*cos(e2)^2*cos(e3)^2*cos(e5)*cos(e6)*sin(e6) - 2*I6xx*de1*cos(e2)^2*cos(e4)^2*cos(e5)*cos(e6)*sin(e6) - 2*I6xx*de1*cos(e3)^2*cos(e4)^2*cos(e5)*cos(e6)*sin(e6) + 2*I6yy*de1*cos(e2)^2*cos(e3)^2*cos(e5)*cos(e6)*sin(e6) + 2*I6yy*de1*cos(e2)^2*cos(e4)^2*cos(e5)*cos(e6)*sin(e6) + 2*I6yy*de1*cos(e3)^2*cos(e4)^2*cos(e5)*cos(e6)*sin(e6) - a2*de1*m4*x4*cos(e2)^2*cos(e3)*sin(e4) + a3*de1*m5*x5*cos(e2)^2*cos(e5)*sin(e4) + a3*de1*m5*x5*cos(e3)^2*cos(e5)*sin(e4) + a3*de1*m6*x6*cos(e2)^2*cos(e4)*sin(e6) + a3*de1*m6*x6*cos(e3)^2*cos(e4)*sin(e6) + 4*I5xy*de1*cos(e2)*cos(e3)^2*cos(e5)^2*sin(e2)*sin(e4) + 4*I5xy*de1*cos(e2)^2*cos(e3)*cos(e5)^2*sin(e3)*sin(e4) - I6xx*de5*cos(e4)*cos(e5)^2*cos(e6)^2*sin(e2)*sin(e3) + I6yy*de5*cos(e4)*cos(e5)^2*cos(e6)^2*sin(e2)*sin(e3) - a3*de1*m5*y5*cos(e2)^2*sin(e4)*sin(e5) - a3*de1*m5*y5*cos(e3)^2*sin(e4)*sin(e5) - a3*de1*m6*z6*cos(e2)^2*sin(e4)*sin(e5) - a3*de1*m6*z6*cos(e3)^2*sin(e4)*sin(e5) - de2*m5*x5^2*cos(e2)*cos(e3)*cos(e4)^2*cos(e5)^2 - de3*m5*x5^2*cos(e2)*cos(e3)*cos(e4)^2*cos(e5)^2 - de2*m6*x6^2*cos(e2)*cos(e3)*cos(e4)^2*cos(e6)^2 - de3*m6*x6^2*cos(e2)*cos(e3)*cos(e4)^2*cos(e6)^2 + de2*m5*y5^2*cos(e2)*cos(e3)*cos(e4)^2*cos(e5)^2 + de3*m5*y5^2*cos(e2)*cos(e3)*cos(e4)^2*cos(e5)^2 - de2*m6*y6^2*cos(e2)*cos(e3)*cos(e4)^2*cos(e5)^2 + de2*m6*y6^2*cos(e2)*cos(e3)*cos(e4)^2*cos(e6)^2 - de3*m6*y6^2*cos(e2)*cos(e3)*cos(e4)^2*cos(e5)^2 + de3*m6*y6^2*cos(e2)*cos(e3)*cos(e4)^2*cos(e6)^2 + 2*de5*m5*x5*y5*cos(e2)*cos(e5)^2*sin(e3) + 2*de5*m5*x5*y5*cos(e3)*cos(e5)^2*sin(e2) - de6*m6*x6*y6*cos(e2)*cos(e5)^2*sin(e3) - de6*m6*x6*y6*cos(e3)*cos(e5)^2*sin(e2) - 2*de6*m6*x6*y6*cos(e2)*cos(e6)^2*sin(e3) - 2*de6*m6*x6*y6*cos(e3)*cos(e6)^2*sin(e2) + de2*m6*z6^2*cos(e2)*cos(e3)*cos(e4)^2*cos(e5)^2 + de3*m6*z6^2*cos(e2)*cos(e3)*cos(e4)^2*cos(e5)^2 + de1*m6*y6*z6*cos(e2)^2*cos(e6)*sin(e5) + de1*m6*y6*z6*cos(e3)^2*cos(e6)*sin(e5) + 2*de1*m6*y6*z6*cos(e4)^2*cos(e6)*sin(e5) - 2*de1*m4*x4^2*cos(e2)^2*cos(e3)^2*cos(e4)*sin(e4) + de1*m5*x5^2*cos(e2)^2*cos(e4)*cos(e5)^2*sin(e4) + 2*de1*m6*x6^2*cos(e2)^2*cos(e3)^2*cos(e4)*sin(e4) + de1*m5*x5^2*cos(e3)^2*cos(e4)*cos(e5)^2*sin(e4) + de1*m6*x6^2*cos(e2)^2*cos(e4)*cos(e6)^2*sin(e4) + de1*m6*x6^2*cos(e3)^2*cos(e4)*cos(e6)^2*sin(e4) - de1*m6*x6^2*cos(e4)*cos(e5)^2*cos(e6)^2*sin(e4) + 2*de1*m4*y4^2*cos(e2)^2*cos(e3)^2*cos(e4)*sin(e4) - 2*de1*m5*y5^2*cos(e2)^2*cos(e3)^2*cos(e4)*sin(e4) - de1*m5*y5^2*cos(e2)^2*cos(e4)*cos(e5)^2*sin(e4) - de1*m5*y5^2*cos(e3)^2*cos(e4)*cos(e5)^2*sin(e4) + de1*m6*y6^2*cos(e2)^2*cos(e4)*cos(e5)^2*sin(e4) - de1*m6*y6^2*cos(e2)^2*cos(e4)*cos(e6)^2*sin(e4) + de1*m6*y6^2*cos(e3)^2*cos(e4)*cos(e5)^2*sin(e4) - de1*m6*y6^2*cos(e3)^2*cos(e4)*cos(e6)^2*sin(e4) + de1*m6*y6^2*cos(e4)*cos(e5)^2*cos(e6)^2*sin(e4) + 2*de1*m5*z5^2*cos(e2)^2*cos(e3)^2*cos(e4)*sin(e4) - 2*de1*m6*z6^2*cos(e2)^2*cos(e3)^2*cos(e4)*sin(e4) - de1*m6*z6^2*cos(e2)^2*cos(e4)*cos(e5)^2*sin(e4) - de1*m6*z6^2*cos(e3)^2*cos(e4)*cos(e5)^2*sin(e4) + de1*m6*x6*z6*cos(e2)^2*sin(e5)*sin(e6) + de1*m6*x6*z6*cos(e3)^2*sin(e5)*sin(e6) + 2*de1*m6*x6*z6*cos(e4)^2*sin(e5)*sin(e6) + 2*a3*de1*m5*y5*cos(e2)^2*cos(e3)^2*sin(e4)*sin(e5) + 2*a3*de1*m6*z6*cos(e2)^2*cos(e3)^2*sin(e4)*sin(e5) + 2*I6xy*de6*cos(e6)*sin(e2)*sin(e3)*sin(e4)*sin(e5)*sin(e6) + 2*I6zx*de2*cos(e4)*sin(e2)*sin(e3)*sin(e4)*sin(e5)*sin(e6) + 2*I6zx*de3*cos(e4)*sin(e2)*sin(e3)*sin(e4)*sin(e5)*sin(e6) - de2*m6*x6^2*cos(e2)*cos(e3)*cos(e4)^2*cos(e5)^2*cos(e6)^2 - de3*m6*x6^2*cos(e2)*cos(e3)*cos(e4)^2*cos(e5)^2*cos(e6)^2 + de2*m6*y6^2*cos(e2)*cos(e3)*cos(e4)^2*cos(e5)^2*cos(e6)^2 + de3*m6*y6^2*cos(e2)*cos(e3)*cos(e4)^2*cos(e5)^2*cos(e6)^2 + de2*m5*x5^2*cos(e2)*cos(e4)*cos(e5)*sin(e3)*sin(e5) + de2*m5*x5^2*cos(e3)*cos(e4)*cos(e5)*sin(e2)*sin(e5) + de3*m5*x5^2*cos(e2)*cos(e4)*cos(e5)*sin(e3)*sin(e5) + de3*m5*x5^2*cos(e3)*cos(e4)*cos(e5)*sin(e2)*sin(e5) + 2*de6*m6*x6*y6*cos(e2)*cos(e5)^2*cos(e6)^2*sin(e3) + 2*de6*m6*x6*y6*cos(e3)*cos(e5)^2*cos(e6)^2*sin(e2) - de2*m5*y5^2*cos(e2)*cos(e4)*cos(e5)*sin(e3)*sin(e5) - de2*m5*y5^2*cos(e3)*cos(e4)*cos(e5)*sin(e2)*sin(e5) - de3*m5*y5^2*cos(e2)*cos(e4)*cos(e5)*sin(e3)*sin(e5) - de3*m5*y5^2*cos(e3)*cos(e4)*cos(e5)*sin(e2)*sin(e5) + de2*m6*y6^2*cos(e2)*cos(e4)*cos(e5)*sin(e3)*sin(e5) + de2*m6*y6^2*cos(e3)*cos(e4)*cos(e5)*sin(e2)*sin(e5) + de3*m6*y6^2*cos(e2)*cos(e4)*cos(e5)*sin(e3)*sin(e5) + de3*m6*y6^2*cos(e3)*cos(e4)*cos(e5)*sin(e2)*sin(e5) - de2*m6*z6^2*cos(e2)*cos(e4)*cos(e5)*sin(e3)*sin(e5) - de2*m6*z6^2*cos(e3)*cos(e4)*cos(e5)*sin(e2)*sin(e5) - de3*m6*z6^2*cos(e2)*cos(e4)*cos(e5)*sin(e3)*sin(e5) - de3*m6*z6^2*cos(e3)*cos(e4)*cos(e5)*sin(e2)*sin(e5) - 2*de1*m6*y6*z6*cos(e2)^2*cos(e3)^2*cos(e6)*sin(e5) - 2*de1*m6*y6*z6*cos(e2)^2*cos(e4)^2*cos(e6)*sin(e5) - 2*de1*m6*y6*z6*cos(e3)^2*cos(e4)^2*cos(e6)*sin(e5) - 2*de1*m5*x5^2*cos(e2)^2*cos(e3)^2*cos(e4)*cos(e5)^2*sin(e4) - 2*de1*m6*x6^2*cos(e2)^2*cos(e3)^2*cos(e4)*cos(e6)^2*sin(e4) + de1*m6*x6^2*cos(e2)^2*cos(e4)*cos(e5)^2*cos(e6)^2*sin(e4) + de1*m6*x6^2*cos(e3)^2*cos(e4)*cos(e5)^2*cos(e6)^2*sin(e4) + 2*de1*m5*y5^2*cos(e2)^2*cos(e3)^2*cos(e4)*cos(e5)^2*sin(e4) - 2*de1*m6*y6^2*cos(e2)^2*cos(e3)^2*cos(e4)*cos(e5)^2*sin(e4) + 2*de1*m6*y6^2*cos(e2)^2*cos(e3)^2*cos(e4)*cos(e6)^2*sin(e4) - de1*m6*y6^2*cos(e2)^2*cos(e4)*cos(e5)^2*cos(e6)^2*sin(e4) - de1*m6*y6^2*cos(e3)^2*cos(e4)*cos(e5)^2*cos(e6)^2*sin(e4) - de1*m5*x5^2*cos(e2)*cos(e5)*sin(e2)*sin(e4)*sin(e5) - de1*m5*x5^2*cos(e3)*cos(e5)*sin(e3)*sin(e4)*sin(e5) + 2*de1*m6*z6^2*cos(e2)^2*cos(e3)^2*cos(e4)*cos(e5)^2*sin(e4) + de1*m5*y5^2*cos(e2)*cos(e5)*sin(e2)*sin(e4)*sin(e5) + de1*m5*y5^2*cos(e3)*cos(e5)*sin(e3)*sin(e4)*sin(e5) - de1*m6*y6^2*cos(e2)*cos(e5)*sin(e2)*sin(e4)*sin(e5) - de1*m6*y6^2*cos(e3)*cos(e5)*sin(e3)*sin(e4)*sin(e5) - 2*de1*m6*x6*z6*cos(e2)^2*cos(e3)^2*sin(e5)*sin(e6) - 2*de1*m6*x6*z6*cos(e2)^2*cos(e4)^2*sin(e5)*sin(e6) - 2*de1*m6*x6*z6*cos(e3)^2*cos(e4)^2*sin(e5)*sin(e6) + de1*m6*z6^2*cos(e2)*cos(e5)*sin(e2)*sin(e4)*sin(e5) + de1*m6*z6^2*cos(e3)*cos(e5)*sin(e3)*sin(e4)*sin(e5) - a3*de2*m5*x5*cos(e2)*cos(e3)*cos(e4)*cos(e5) - a3*de3*m5*x5*cos(e2)*cos(e3)*cos(e4)*cos(e5) - a2*de2*m6*x6*cos(e2)*cos(e4)*cos(e5)*cos(e6) + 4*I6xy*de2*cos(e2)*cos(e3)*cos(e4)*cos(e5)*cos(e6)^2*sin(e4) + 4*I6xy*de3*cos(e2)*cos(e3)*cos(e4)*cos(e5)*cos(e6)^2*sin(e4) + 2*I6xy*de5*cos(e2)*cos(e3)*cos(e4)*cos(e5)^2*cos(e6)*sin(e6) + 2*I6xy*de6*cos(e2)*cos(e3)*cos(e4)*cos(e5)*cos(e6)^2*sin(e5) + 2*I6yz*de1*cos(e2)*cos(e3)^2*cos(e4)*cos(e5)*cos(e6)*sin(e2) + 2*I6yz*de1*cos(e2)^2*cos(e3)*cos(e4)*cos(e5)*cos(e6)*sin(e3) + 2*I6zx*de2*cos(e2)*cos(e3)*cos(e4)^2*cos(e5)*cos(e6)*sin(e5) + 2*I6zx*de3*cos(e2)*cos(e3)*cos(e4)^2*cos(e5)*cos(e6)*sin(e5) + de2*m6*x6^2*cos(e4)^2*cos(e5)^2*cos(e6)^2*sin(e2)*sin(e3) + de3*m6*x6^2*cos(e4)^2*cos(e5)^2*cos(e6)^2*sin(e2)*sin(e3) - de2*m6*y6^2*cos(e4)^2*cos(e5)^2*cos(e6)^2*sin(e2)*sin(e3) - de3*m6*y6^2*cos(e4)^2*cos(e5)^2*cos(e6)^2*sin(e2)*sin(e3) + a2*de1*m6*x6*cos(e3)*cos(e5)*cos(e6)*sin(e4) + a1*de1*m6*y6*cos(e2)*cos(e4)*cos(e6)*sin(e3) + a1*de1*m6*y6*cos(e3)*cos(e4)*cos(e6)*sin(e2) + a3*de2*m5*y5*cos(e2)*cos(e3)*cos(e4)*sin(e5) + a3*de3*m5*y5*cos(e2)*cos(e3)*cos(e4)*sin(e5) + a3*de2*m6*y6*cos(e2)*cos(e3)*cos(e6)*sin(e4) + a2*de2*m6*y6*cos(e2)*cos(e4)*cos(e5)*sin(e6) + a3*de3*m6*y6*cos(e2)*cos(e3)*cos(e6)*sin(e4) + a3*de2*m6*z6*cos(e2)*cos(e3)*cos(e4)*sin(e5) + a3*de3*m6*z6*cos(e2)*cos(e3)*cos(e4)*sin(e5) + d4*de2*m5*x5*cos(e2)*cos(e4)*cos(e5)*sin(e3) + d4*de2*m5*x5*cos(e3)*cos(e4)*cos(e5)*sin(e2) + d4*de3*m5*x5*cos(e2)*cos(e4)*cos(e5)*sin(e3) + d4*de3*m5*x5*cos(e3)*cos(e4)*cos(e5)*sin(e2) - 4*I6xy*de1*cos(e2)*cos(e3)*cos(e4)^2*cos(e5)*sin(e2)*sin(e3) - 4*I6xy*de1*cos(e2)*cos(e3)*cos(e5)*cos(e6)^2*sin(e2)*sin(e3) - I6xx*de2*cos(e2)*cos(e4)*cos(e5)*cos(e6)^2*sin(e3)*sin(e5) - I6xx*de2*cos(e3)*cos(e4)*cos(e5)*cos(e6)^2*sin(e2)*sin(e5) - I6xx*de3*cos(e2)*cos(e4)*cos(e5)*cos(e6)^2*sin(e3)*sin(e5) - I6xx*de3*cos(e3)*cos(e4)*cos(e5)*cos(e6)^2*sin(e2)*sin(e5) + I6yy*de2*cos(e2)*cos(e4)*cos(e5)*cos(e6)^2*sin(e3)*sin(e5) + I6yy*de2*cos(e3)*cos(e4)*cos(e5)*cos(e6)^2*sin(e2)*sin(e5) + I6yy*de3*cos(e2)*cos(e4)*cos(e5)*cos(e6)^2*sin(e3)*sin(e5) + I6yy*de3*cos(e3)*cos(e4)*cos(e5)*cos(e6)^2*sin(e2)*sin(e5) - 2*I6yz*de2*cos(e2)*cos(e3)*cos(e4)^2*cos(e5)*sin(e5)*sin(e6) - 2*I6yz*de3*cos(e2)*cos(e3)*cos(e4)^2*cos(e5)*sin(e5)*sin(e6) - 4*I5zx*de1*cos(e2)*cos(e3)*cos(e4)^2*cos(e5)*sin(e2)*sin(e3) + 2*I6zx*de1*cos(e2)*cos(e3)^2*cos(e4)*cos(e5)*sin(e2)*sin(e6) + 2*I6zx*de1*cos(e2)^2*cos(e3)*cos(e4)*cos(e5)*sin(e3)*sin(e6) - 2*I6zx*de1*cos(e2)^2*cos(e4)*cos(e5)*cos(e6)*sin(e4)*sin(e5) - 2*I6zx*de1*cos(e3)^2*cos(e4)*cos(e5)*cos(e6)*sin(e4)*sin(e5) - d4*de1*m6*y6*cos(e2)*cos(e4)*cos(e6)*sin(e2) - d4*de1*m6*y6*cos(e3)*cos(e4)*cos(e6)*sin(e3) - de6*m6*y6*z6*cos(e2)*cos(e3)*cos(e4)*cos(e6) + a1*de1*m5*x5*cos(e2)*cos(e5)*sin(e3)*sin(e4) + a1*de1*m5*x5*cos(e3)*cos(e5)*sin(e2)*sin(e4) + a1*de1*m6*x6*cos(e2)*cos(e4)*sin(e3)*sin(e6) + a1*de1*m6*x6*cos(e3)*cos(e4)*sin(e2)*sin(e6) + a3*de2*m5*x5*cos(e4)*cos(e5)*sin(e2)*sin(e3) + a3*de3*m5*x5*cos(e4)*cos(e5)*sin(e2)*sin(e3) + a3*de2*m6*x6*cos(e2)*cos(e3)*sin(e4)*sin(e6) + a3*de3*m6*x6*cos(e2)*cos(e3)*sin(e4)*sin(e6) + a2*de1*m4*y4*cos(e2)*cos(e4)*sin(e2)*sin(e3) - a2*de1*m6*y6*cos(e3)*cos(e5)*sin(e4)*sin(e6) + 2*I6xx*de1*cos(e2)^2*cos(e3)^2*cos(e4)*cos(e5)^2*cos(e6)^2*sin(e4) - 2*I6yy*de1*cos(e2)^2*cos(e3)^2*cos(e4)*cos(e5)^2*cos(e6)^2*sin(e4) - a2*de1*m5*z5*cos(e2)*cos(e4)*sin(e2)*sin(e3) - d4*de1*m5*x5*cos(e2)*cos(e5)*sin(e2)*sin(e4) - d4*de1*m5*x5*cos(e3)*cos(e5)*sin(e3)*sin(e4) - d4*de1*m6*x6*cos(e2)*cos(e4)*sin(e2)*sin(e6) - d4*de1*m6*x6*cos(e3)*cos(e4)*sin(e3)*sin(e6) - 2*I5xx*de1*cos(e2)*cos(e3)^2*cos(e5)*sin(e2)*sin(e4)*sin(e5) - 2*I5xx*de1*cos(e2)^2*cos(e3)*cos(e5)*sin(e3)*sin(e4)*sin(e5) + I6xx*de1*cos(e2)*cos(e5)*cos(e6)^2*sin(e2)*sin(e4)*sin(e5) + I6xx*de1*cos(e3)*cos(e5)*cos(e6)^2*sin(e3)*sin(e4)*sin(e5) - 4*I6xy*de2*cos(e4)*cos(e5)*cos(e6)^2*sin(e2)*sin(e3)*sin(e4) - 4*I6xy*de3*cos(e4)*cos(e5)*cos(e6)^2*sin(e2)*sin(e3)*sin(e4) - 2*I6xy*de5*cos(e4)*cos(e5)^2*cos(e6)*sin(e2)*sin(e3)*sin(e6) - 2*I6xy*de6*cos(e4)*cos(e5)*cos(e6)^2*sin(e2)*sin(e3)*sin(e5) + 4*I5yz*de1*cos(e2)*cos(e3)*cos(e4)^2*sin(e2)*sin(e3)*sin(e5) + 2*I5yy*de1*cos(e2)*cos(e3)^2*cos(e5)*sin(e2)*sin(e4)*sin(e5) + 2*I5yy*de1*cos(e2)^2*cos(e3)*cos(e5)*sin(e3)*sin(e4)*sin(e5) - 2*I6yy*de1*cos(e2)*cos(e3)^2*cos(e5)*sin(e2)*sin(e4)*sin(e5) - 2*I6yy*de1*cos(e2)^2*cos(e3)*cos(e5)*sin(e3)*sin(e4)*sin(e5) - I6yy*de1*cos(e2)*cos(e5)*cos(e6)^2*sin(e2)*sin(e4)*sin(e5) - I6yy*de1*cos(e3)*cos(e5)*cos(e6)^2*sin(e3)*sin(e4)*sin(e5) + 2*I6yz*de1*cos(e2)^2*cos(e4)*cos(e5)*sin(e4)*sin(e5)*sin(e6) + 2*I6yz*de1*cos(e3)^2*cos(e4)*cos(e5)*sin(e4)*sin(e5)*sin(e6) + 2*I6zz*de1*cos(e2)*cos(e3)^2*cos(e5)*sin(e2)*sin(e4)*sin(e5) + 2*I6zz*de1*cos(e2)^2*cos(e3)*cos(e5)*sin(e3)*sin(e4)*sin(e5) - 2*I6zx*de2*cos(e4)^2*cos(e5)*cos(e6)*sin(e2)*sin(e3)*sin(e5) - 2*I6zx*de3*cos(e4)^2*cos(e5)*cos(e6)*sin(e2)*sin(e3)*sin(e5) - d4*de2*m5*y5*cos(e2)*cos(e4)*sin(e3)*sin(e5) - d4*de2*m5*y5*cos(e3)*cos(e4)*sin(e2)*sin(e5) - d4*de3*m5*y5*cos(e2)*cos(e4)*sin(e3)*sin(e5) - d4*de3*m5*y5*cos(e3)*cos(e4)*sin(e2)*sin(e5) - d4*de2*m6*y6*cos(e2)*cos(e6)*sin(e3)*sin(e4) - d4*de2*m6*y6*cos(e3)*cos(e6)*sin(e2)*sin(e4) - d4*de3*m6*y6*cos(e2)*cos(e6)*sin(e3)*sin(e4) - d4*de3*m6*y6*cos(e3)*cos(e6)*sin(e2)*sin(e4) - d4*de2*m6*z6*cos(e2)*cos(e4)*sin(e3)*sin(e5) - d4*de2*m6*z6*cos(e3)*cos(e4)*sin(e2)*sin(e5) - d4*de3*m6*z6*cos(e2)*cos(e4)*sin(e3)*sin(e5) - d4*de3*m6*z6*cos(e3)*cos(e4)*sin(e2)*sin(e5) + 2*de2*m4*x4*y4*cos(e2)*cos(e3)*cos(e4)*sin(e4) + 2*de3*m4*x4*y4*cos(e2)*cos(e3)*cos(e4)*sin(e4) - 2*de2*m6*x6*y6*cos(e2)*cos(e3)*cos(e6)*sin(e6) - de5*m6*x6*y6*cos(e2)*cos(e3)*cos(e5)*sin(e4) - 2*de3*m6*x6*y6*cos(e2)*cos(e3)*cos(e6)*sin(e6) - de5*m5*x5*z5*cos(e2)*cos(e3)*cos(e5)*sin(e4) - de2*m6*x6*z6*cos(e2)*cos(e4)*cos(e6)*sin(e3) - de2*m6*x6*z6*cos(e3)*cos(e4)*cos(e6)*sin(e2) - de3*m6*x6*z6*cos(e2)*cos(e4)*cos(e6)*sin(e3) - de3*m6*x6*z6*cos(e3)*cos(e4)*cos(e6)*sin(e2) - de6*m6*x6*z6*cos(e2)*cos(e3)*cos(e4)*sin(e6) + de1*m5*y5*z5*cos(e2)*cos(e4)*cos(e5)*sin(e2) + de1*m5*y5*z5*cos(e3)*cos(e4)*cos(e5)*sin(e3) + a2*de1*m4*x4*cos(e2)*sin(e2)*sin(e3)*sin(e4) - a1*de1*m5*y5*cos(e2)*sin(e3)*sin(e4)*sin(e5) - a1*de1*m5*y5*cos(e3)*sin(e2)*sin(e4)*sin(e5) - a3*de2*m5*y5*cos(e4)*sin(e2)*sin(e3)*sin(e5) - a3*de3*m5*y5*cos(e4)*sin(e2)*sin(e3)*sin(e5) - a3*de2*m6*y6*cos(e6)*sin(e2)*sin(e3)*sin(e4) - a3*de3*m6*y6*cos(e6)*sin(e2)*sin(e3)*sin(e4) - a1*de1*m6*z6*cos(e2)*sin(e3)*sin(e4)*sin(e5) - a1*de1*m6*z6*cos(e3)*sin(e2)*sin(e4)*sin(e5) - a3*de2*m6*z6*cos(e4)*sin(e2)*sin(e3)*sin(e5) - a3*de3*m6*z6*cos(e4)*sin(e2)*sin(e3)*sin(e5) - d4*de2*m6*x6*cos(e2)*sin(e3)*sin(e4)*sin(e6) - d4*de2*m6*x6*cos(e3)*sin(e2)*sin(e4)*sin(e6) - d4*de3*m6*x6*cos(e2)*sin(e3)*sin(e4)*sin(e6) - d4*de3*m6*x6*cos(e3)*sin(e2)*sin(e4)*sin(e6) + 2*I6yz*de2*cos(e4)^2*cos(e5)*sin(e2)*sin(e3)*sin(e5)*sin(e6) + 2*I6yz*de3*cos(e4)^2*cos(e5)*sin(e2)*sin(e3)*sin(e5)*sin(e6) + d4*de1*m5*y5*cos(e2)*sin(e2)*sin(e4)*sin(e5) + d4*de1*m5*y5*cos(e3)*sin(e3)*sin(e4)*sin(e5) + d4*de1*m6*z6*cos(e2)*sin(e2)*sin(e4)*sin(e5) + d4*de1*m6*z6*cos(e3)*sin(e3)*sin(e4)*sin(e5) + 4*de1*m6*x6*y6*cos(e2)^2*cos(e3)^2*cos(e4)^2*cos(e5) + 4*de1*m6*x6*y6*cos(e2)^2*cos(e3)^2*cos(e5)*cos(e6)^2 + 4*de1*m6*x6*y6*cos(e2)^2*cos(e4)^2*cos(e5)*cos(e6)^2 + 4*de1*m6*x6*y6*cos(e3)^2*cos(e4)^2*cos(e5)*cos(e6)^2 + 4*de1*m5*x5*z5*cos(e2)^2*cos(e3)^2*cos(e4)^2*cos(e5) - 2*de1*m4*x4*y4*cos(e2)*cos(e3)*sin(e2)*sin(e3) + de1*m6*x6*y6*cos(e2)*cos(e4)*sin(e2)*sin(e5) + 2*de1*m5*x5*y5*cos(e4)*cos(e5)*sin(e4)*sin(e5) + de1*m6*x6*y6*cos(e3)*cos(e4)*sin(e3)*sin(e5) + 2*de1*m6*x6*y6*cos(e4)*cos(e6)*sin(e4)*sin(e6) + de1*m5*x5*z5*cos(e2)*cos(e4)*sin(e2)*sin(e5) + de1*m5*x5*z5*cos(e3)*cos(e4)*sin(e3)*sin(e5) + de1*m6*x6*z6*cos(e2)*cos(e6)*sin(e2)*sin(e4) + de1*m6*x6*z6*cos(e3)*cos(e6)*sin(e3)*sin(e4) + de2*m5*y5*z5*cos(e2)*cos(e5)*sin(e3)*sin(e4) + de2*m5*y5*z5*cos(e3)*cos(e5)*sin(e2)*sin(e4) + de3*m5*y5*z5*cos(e2)*cos(e5)*sin(e3)*sin(e4) + de3*m5*y5*z5*cos(e3)*cos(e5)*sin(e2)*sin(e4) + de5*m5*y5*z5*cos(e2)*cos(e3)*sin(e4)*sin(e5) + de2*m6*y6*z6*cos(e2)*cos(e4)*sin(e3)*sin(e6) + de2*m6*y6*z6*cos(e3)*cos(e4)*sin(e2)*sin(e6) + de3*m6*y6*z6*cos(e2)*cos(e4)*sin(e3)*sin(e6) + de3*m6*y6*z6*cos(e3)*cos(e4)*sin(e2)*sin(e6) + de6*m6*y6*z6*cos(e4)*cos(e6)*sin(e2)*sin(e3) - a3*de2*m6*x6*sin(e2)*sin(e3)*sin(e4)*sin(e6) - a3*de3*m6*x6*sin(e2)*sin(e3)*sin(e4)*sin(e6) + de5*m6*x6^2*cos(e2)*cos(e5)*cos(e6)^2*sin(e3)*sin(e5) + de5*m6*x6^2*cos(e3)*cos(e5)*cos(e6)^2*sin(e2)*sin(e5) + de6*m6*x6^2*cos(e2)*cos(e3)*cos(e6)^2*sin(e4)*sin(e5) + de6*m6*x6^2*cos(e2)*cos(e5)^2*cos(e6)*sin(e3)*sin(e6) + de6*m6*x6^2*cos(e3)*cos(e5)^2*cos(e6)*sin(e2)*sin(e6) - de5*m6*y6^2*cos(e2)*cos(e5)*cos(e6)^2*sin(e3)*sin(e5) - de5*m6*y6^2*cos(e3)*cos(e5)*cos(e6)^2*sin(e2)*sin(e5) - de6*m6*y6^2*cos(e2)*cos(e3)*cos(e6)^2*sin(e4)*sin(e5) - de6*m6*y6^2*cos(e2)*cos(e5)^2*cos(e6)*sin(e3)*sin(e6) - de6*m6*y6^2*cos(e3)*cos(e5)^2*cos(e6)*sin(e2)*sin(e6) - 2*de2*m4*x4*y4*cos(e4)*sin(e2)*sin(e3)*sin(e4) - 2*de3*m4*x4*y4*cos(e4)*sin(e2)*sin(e3)*sin(e4) + de2*m6*x6*y6*cos(e2)*sin(e3)*sin(e4)*sin(e5) + de2*m6*x6*y6*cos(e3)*sin(e2)*sin(e4)*sin(e5) + de3*m6*x6*y6*cos(e2)*sin(e3)*sin(e4)*sin(e5) + de3*m6*x6*y6*cos(e3)*sin(e2)*sin(e4)*sin(e5) + 2*de2*m6*x6*y6*cos(e6)*sin(e2)*sin(e3)*sin(e6) + de5*m6*x6*y6*cos(e5)*sin(e2)*sin(e3)*sin(e4) + 2*de3*m6*x6*y6*cos(e6)*sin(e2)*sin(e3)*sin(e6) - 4*de1*m5*y5*z5*cos(e2)^2*cos(e3)^2*cos(e4)^2*sin(e5) + de2*m5*x5*z5*cos(e2)*sin(e3)*sin(e4)*sin(e5) + de2*m5*x5*z5*cos(e3)*sin(e2)*sin(e4)*sin(e5) + de3*m5*x5*z5*cos(e2)*sin(e3)*sin(e4)*sin(e5) + de3*m5*x5*z5*cos(e3)*sin(e2)*sin(e4)*sin(e5) + de5*m5*x5*z5*cos(e5)*sin(e2)*sin(e3)*sin(e4) + de6*m6*x6*z6*cos(e4)*sin(e2)*sin(e3)*sin(e6) - de1*m6*y6*z6*cos(e2)*sin(e2)*sin(e4)*sin(e6) - de1*m6*y6*z6*cos(e3)*sin(e3)*sin(e4)*sin(e6) - de5*m5*y5*z5*sin(e2)*sin(e3)*sin(e4)*sin(e5) - a2*de1*m6*y6*cos(e2)^2*cos(e3)*cos(e4)*cos(e6) + 2*I6xy*de2*cos(e2)*cos(e3)*cos(e4)^2*cos(e5)^2*cos(e6)*sin(e6) + 2*I6xy*de3*cos(e2)*cos(e3)*cos(e4)^2*cos(e5)^2*cos(e6)*sin(e6) - de6*m6*x6^2*cos(e6)^2*sin(e2)*sin(e3)*sin(e4)*sin(e5) + de6*m6*y6^2*cos(e6)^2*sin(e2)*sin(e3)*sin(e4)*sin(e5) - a2*de1*m5*x5*cos(e2)^2*cos(e3)*cos(e5)*sin(e4) - a2*de1*m6*x6*cos(e2)^2*cos(e3)*cos(e4)*sin(e6) + a3*de1*m6*x6*cos(e2)^2*cos(e5)*cos(e6)*sin(e4) + a3*de1*m6*x6*cos(e3)^2*cos(e5)*cos(e6)*sin(e4) + 4*I5xy*de1*cos(e2)^2*cos(e3)^2*cos(e4)*cos(e5)*sin(e4)*sin(e5) + 4*I6xy*de1*cos(e2)*cos(e3)^2*cos(e4)*cos(e6)^2*sin(e2)*sin(e5) + 4*I6xy*de1*cos(e2)^2*cos(e3)*cos(e4)*cos(e6)^2*sin(e3)*sin(e5) + 4*I6xy*de1*cos(e2)^2*cos(e3)^2*cos(e4)*cos(e6)*sin(e4)*sin(e6) - 2*I6xy*de1*cos(e2)^2*cos(e4)*cos(e5)^2*cos(e6)*sin(e4)*sin(e6) - 2*I6xy*de1*cos(e3)^2*cos(e4)*cos(e5)^2*cos(e6)*sin(e4)*sin(e6) + 4*I6zx*de1*cos(e2)*cos(e3)^2*cos(e5)^2*cos(e6)*sin(e2)*sin(e4) + 4*I6zx*de1*cos(e2)^2*cos(e3)*cos(e5)^2*cos(e6)*sin(e3)*sin(e4) + 2*d4*de1*m4*y4*cos(e2)*cos(e3)^2*cos(e4)*sin(e2) + 2*d4*de1*m4*y4*cos(e2)^2*cos(e3)*cos(e4)*sin(e3) - 2*d4*de1*m5*z5*cos(e2)*cos(e3)^2*cos(e4)*sin(e2) - 2*d4*de1*m5*z5*cos(e2)^2*cos(e3)*cos(e4)*sin(e3) + a2*de1*m5*y5*cos(e2)^2*cos(e3)*sin(e4)*sin(e5) - a3*de1*m6*y6*cos(e2)^2*cos(e5)*sin(e4)*sin(e6) - a3*de1*m6*y6*cos(e3)^2*cos(e5)*sin(e4)*sin(e6) + a2*de1*m6*z6*cos(e2)^2*cos(e3)*sin(e4)*sin(e5) + 2*d4*de1*m4*x4*cos(e2)*cos(e3)^2*sin(e2)*sin(e4) + 2*d4*de1*m4*x4*cos(e2)^2*cos(e3)*sin(e3)*sin(e4) - 2*I6xy*de2*cos(e4)^2*cos(e5)^2*cos(e6)*sin(e2)*sin(e3)*sin(e6) - 2*I6xy*de3*cos(e4)^2*cos(e5)^2*cos(e6)*sin(e2)*sin(e3)*sin(e6) - 4*I6yz*de1*cos(e2)*cos(e3)^2*cos(e5)^2*sin(e2)*sin(e4)*sin(e6) - 4*I6yz*de1*cos(e2)^2*cos(e3)*cos(e5)^2*sin(e3)*sin(e4)*sin(e6) - de5*m6*x6^2*cos(e2)*cos(e3)*cos(e4)*cos(e5)^2*cos(e6)^2 + de5*m6*y6^2*cos(e2)*cos(e3)*cos(e4)*cos(e5)^2*cos(e6)^2 + 2*de2*m5*x5*y5*cos(e2)*cos(e4)*cos(e5)^2*sin(e3) + 2*de2*m5*x5*y5*cos(e3)*cos(e4)*cos(e5)^2*sin(e2) + 2*de3*m5*x5*y5*cos(e2)*cos(e4)*cos(e5)^2*sin(e3) + 2*de3*m5*x5*y5*cos(e3)*cos(e4)*cos(e5)^2*sin(e2) + 2*de5*m6*x6*z6*cos(e2)*cos(e5)^2*cos(e6)*sin(e3) + 2*de5*m6*x6*z6*cos(e3)*cos(e5)^2*cos(e6)*sin(e2) + 2*de1*m4*y4*z4*cos(e2)*cos(e3)^2*cos(e4)*sin(e2) + 2*de1*m4*y4*z4*cos(e2)^2*cos(e3)*cos(e4)*sin(e3) + 2*de1*m6*x6^2*cos(e2)^2*cos(e3)^2*cos(e5)*cos(e6)*sin(e6) + 2*de1*m6*x6^2*cos(e2)^2*cos(e4)^2*cos(e5)*cos(e6)*sin(e6) + 2*de1*m6*x6^2*cos(e3)^2*cos(e4)^2*cos(e5)*cos(e6)*sin(e6) - 2*de1*m6*y6^2*cos(e2)^2*cos(e3)^2*cos(e5)*cos(e6)*sin(e6) - 2*de1*m6*y6^2*cos(e2)^2*cos(e4)^2*cos(e5)*cos(e6)*sin(e6) - 2*de1*m6*y6^2*cos(e3)^2*cos(e4)^2*cos(e5)*cos(e6)*sin(e6) - 2*de1*m5*x5*y5*cos(e2)*cos(e3)^2*sin(e2)*sin(e4) - 2*de1*m5*x5*y5*cos(e2)^2*cos(e3)*sin(e3)*sin(e4) - 2*de1*m5*x5*y5*cos(e2)*cos(e5)^2*sin(e2)*sin(e4) - 2*de1*m5*x5*y5*cos(e3)*cos(e5)^2*sin(e3)*sin(e4) + 2*de1*m4*x4*z4*cos(e2)*cos(e3)^2*sin(e2)*sin(e4) + 2*de1*m4*x4*z4*cos(e2)^2*cos(e3)*sin(e3)*sin(e4) - 2*de5*m6*y6*z6*cos(e2)*cos(e5)^2*sin(e3)*sin(e6) - 2*de5*m6*y6*z6*cos(e3)*cos(e5)^2*sin(e2)*sin(e6) + 2*I6zx*de5*cos(e2)*cos(e3)*cos(e4)*cos(e5)*cos(e6)*sin(e5) + de5*m6*x6^2*cos(e4)*cos(e5)^2*cos(e6)^2*sin(e2)*sin(e3) - de5*m6*y6^2*cos(e4)*cos(e5)^2*cos(e6)^2*sin(e2)*sin(e3) - I6xx*de5*cos(e2)*cos(e3)*cos(e5)*cos(e6)*sin(e4)*sin(e6) - 2*I6yz*de2*cos(e2)*cos(e3)*cos(e4)*cos(e6)*sin(e4)*sin(e5) - 2*I6yz*de3*cos(e2)*cos(e3)*cos(e4)*cos(e6)*sin(e4)*sin(e5) + I6yy*de5*cos(e2)*cos(e3)*cos(e5)*cos(e6)*sin(e4)*sin(e6) - 2*I6yz*de5*cos(e2)*cos(e3)*cos(e4)*cos(e5)*sin(e5)*sin(e6) - 2*a3*de1*m6*y6*cos(e2)^2*cos(e3)^2*cos(e4)*cos(e6) + 4*I6xx*de1*cos(e2)^2*cos(e3)^2*cos(e4)^2*cos(e5)*cos(e6)*sin(e6) - 4*I6yy*de1*cos(e2)^2*cos(e3)^2*cos(e4)^2*cos(e5)*cos(e6)*sin(e6) - 2*I4xx*de1*cos(e2)*cos(e3)*cos(e4)*sin(e2)*sin(e3)*sin(e4) + 2*I6xx*de1*cos(e2)*cos(e3)*cos(e4)*sin(e2)*sin(e3)*sin(e4) + I6xx*de1*cos(e2)*cos(e4)*cos(e6)*sin(e2)*sin(e5)*sin(e6) + I6xx*de1*cos(e3)*cos(e4)*cos(e6)*sin(e3)*sin(e5)*sin(e6) - 2*I6xy*de5*cos(e2)*cos(e5)*cos(e6)*sin(e3)*sin(e5)*sin(e6) - 2*I6xy*de5*cos(e3)*cos(e5)*cos(e6)*sin(e2)*sin(e5)*sin(e6) - 2*I6xy*de6*cos(e2)*cos(e3)*cos(e6)*sin(e4)*sin(e5)*sin(e6) + 2*I4yy*de1*cos(e2)*cos(e3)*cos(e4)*sin(e2)*sin(e3)*sin(e4) - 2*I5yy*de1*cos(e2)*cos(e3)*cos(e4)*sin(e2)*sin(e3)*sin(e4) + 2*I6yz*de1*cos(e2)*cos(e3)*cos(e6)*sin(e2)*sin(e3)*sin(e5) - I6yy*de1*cos(e2)*cos(e4)*cos(e6)*sin(e2)*sin(e5)*sin(e6) - I6yy*de1*cos(e3)*cos(e4)*cos(e6)*sin(e3)*sin(e5)*sin(e6) + 2*I5zz*de1*cos(e2)*cos(e3)*cos(e4)*sin(e2)*sin(e3)*sin(e4) - 2*I6zz*de1*cos(e2)*cos(e3)*cos(e4)*sin(e2)*sin(e3)*sin(e4) - 2*I6zx*de2*cos(e2)*cos(e3)*cos(e4)*sin(e4)*sin(e5)*sin(e6) - 2*I6zx*de3*cos(e2)*cos(e3)*cos(e4)*sin(e4)*sin(e5)*sin(e6) - 2*I6zx*de5*cos(e4)*cos(e5)*cos(e6)*sin(e2)*sin(e3)*sin(e5) - 2*a3*de1*m5*x5*cos(e2)^2*cos(e3)^2*cos(e5)*sin(e4) - 2*a3*de1*m6*x6*cos(e2)^2*cos(e3)^2*cos(e4)*sin(e6) + I6xx*de2*cos(e2)*cos(e6)*sin(e3)*sin(e4)*sin(e5)*sin(e6) + I6xx*de2*cos(e3)*cos(e6)*sin(e2)*sin(e4)*sin(e5)*sin(e6) + I6xx*de3*cos(e2)*cos(e6)*sin(e3)*sin(e4)*sin(e5)*sin(e6) + I6xx*de3*cos(e3)*cos(e6)*sin(e2)*sin(e4)*sin(e5)*sin(e6) + I6xx*de5*cos(e5)*cos(e6)*sin(e2)*sin(e3)*sin(e4)*sin(e6) + 2*I6yz*de2*cos(e4)*cos(e6)*sin(e2)*sin(e3)*sin(e4)*sin(e5) - I6yy*de2*cos(e2)*cos(e6)*sin(e3)*sin(e4)*sin(e5)*sin(e6) - I6yy*de2*cos(e3)*cos(e6)*sin(e2)*sin(e4)*sin(e5)*sin(e6) + 2*I6yz*de3*cos(e4)*cos(e6)*sin(e2)*sin(e3)*sin(e4)*sin(e5) - I6yy*de3*cos(e2)*cos(e6)*sin(e3)*sin(e4)*sin(e5)*sin(e6) - I6yy*de3*cos(e3)*cos(e6)*sin(e2)*sin(e4)*sin(e5)*sin(e6) - I6yy*de5*cos(e5)*cos(e6)*sin(e2)*sin(e3)*sin(e4)*sin(e6) + 2*I6yz*de5*cos(e4)*cos(e5)*sin(e2)*sin(e3)*sin(e5)*sin(e6) + 2*I6zx*de1*cos(e2)*cos(e3)*sin(e2)*sin(e3)*sin(e5)*sin(e6) + a3*de2*m6*y6*cos(e2)*cos(e3)*cos(e4)*cos(e5)*sin(e6) + a3*de3*m6*y6*cos(e2)*cos(e3)*cos(e4)*cos(e5)*sin(e6) + d4*de2*m6*x6*cos(e2)*cos(e4)*cos(e5)*cos(e6)*sin(e3) + d4*de2*m6*x6*cos(e3)*cos(e4)*cos(e5)*cos(e6)*sin(e2) + d4*de3*m6*x6*cos(e2)*cos(e4)*cos(e5)*cos(e6)*sin(e3) + d4*de3*m6*x6*cos(e3)*cos(e4)*cos(e5)*cos(e6)*sin(e2) + a1*de1*m6*x6*cos(e2)*cos(e5)*cos(e6)*sin(e3)*sin(e4) + a1*de1*m6*x6*cos(e3)*cos(e5)*cos(e6)*sin(e2)*sin(e4) + a3*de2*m6*x6*cos(e4)*cos(e5)*cos(e6)*sin(e2)*sin(e3) + a3*de3*m6*x6*cos(e4)*cos(e5)*cos(e6)*sin(e2)*sin(e3) + 2*a3*de1*m4*y4*cos(e2)*cos(e3)*cos(e4)*sin(e2)*sin(e3) + a2*de1*m6*y6*cos(e2)*cos(e4)*cos(e6)*sin(e2)*sin(e3) - 2*a3*de1*m5*z5*cos(e2)*cos(e3)*cos(e4)*sin(e2)*sin(e3) - d4*de1*m6*x6*cos(e2)*cos(e5)*cos(e6)*sin(e2)*sin(e4) - d4*de1*m6*x6*cos(e3)*cos(e5)*cos(e6)*sin(e3)*sin(e4) - 2*I5xx*de1*cos(e2)*cos(e3)*cos(e4)*cos(e5)^2*sin(e2)*sin(e3)*sin(e4) - 2*I6xx*de1*cos(e2)*cos(e3)*cos(e4)*cos(e6)^2*sin(e2)*sin(e3)*sin(e4) - 2*I6xx*de1*cos(e2)*cos(e3)^2*cos(e4)*cos(e6)*sin(e2)*sin(e5)*sin(e6) - 2*I6xx*de1*cos(e2)^2*cos(e3)*cos(e4)*cos(e6)*sin(e3)*sin(e5)*sin(e6) + 2*I5yy*de1*cos(e2)*cos(e3)*cos(e4)*cos(e5)^2*sin(e2)*sin(e3)*sin(e4) - 2*I6yy*de1*cos(e2)*cos(e3)*cos(e4)*cos(e5)^2*sin(e2)*sin(e3)*sin(e4) + 2*I6yy*de1*cos(e2)*cos(e3)*cos(e4)*cos(e6)^2*sin(e2)*sin(e3)*sin(e4) - 4*I6yz*de1*cos(e2)*cos(e3)*cos(e4)^2*cos(e6)*sin(e2)*sin(e3)*sin(e5) + 2*I6yy*de1*cos(e2)*cos(e3)^2*cos(e4)*cos(e6)*sin(e2)*sin(e5)*sin(e6) + 2*I6yy*de1*cos(e2)^2*cos(e3)*cos(e4)*cos(e6)*sin(e3)*sin(e5)*sin(e6) + 2*I6zz*de1*cos(e2)*cos(e3)*cos(e4)*cos(e5)^2*sin(e2)*sin(e3)*sin(e4) - d4*de2*m6*y6*cos(e2)*cos(e4)*cos(e5)*sin(e3)*sin(e6) - d4*de2*m6*y6*cos(e3)*cos(e4)*cos(e5)*sin(e2)*sin(e6) - d4*de3*m6*y6*cos(e2)*cos(e4)*cos(e5)*sin(e3)*sin(e6) - d4*de3*m6*y6*cos(e3)*cos(e4)*cos(e5)*sin(e2)*sin(e6) - 2*de2*m6*x6*y6*cos(e2)*cos(e3)*cos(e4)*cos(e5)*sin(e4) - 2*de3*m6*x6*y6*cos(e2)*cos(e3)*cos(e4)*cos(e5)*sin(e4) + 2*de5*m5*x5*y5*cos(e2)*cos(e3)*cos(e4)*cos(e5)*sin(e5) - de6*m6*x6*y6*cos(e2)*cos(e3)*cos(e4)*cos(e5)*sin(e5) - 2*de2*m5*x5*z5*cos(e2)*cos(e3)*cos(e4)*cos(e5)*sin(e4) - 2*de3*m5*x5*z5*cos(e2)*cos(e3)*cos(e4)*cos(e5)*sin(e4) - de1*m6*y6*z6*cos(e2)*cos(e4)*cos(e5)*cos(e6)*sin(e2) - de1*m6*y6*z6*cos(e3)*cos(e4)*cos(e5)*cos(e6)*sin(e3) + 2*a3*de1*m4*x4*cos(e2)*cos(e3)*sin(e2)*sin(e3)*sin(e4) + a2*de1*m5*x5*cos(e2)*cos(e5)*sin(e2)*sin(e3)*sin(e4) + a2*de1*m6*x6*cos(e2)*cos(e4)*sin(e2)*sin(e3)*sin(e6) - a1*de1*m6*y6*cos(e2)*cos(e5)*sin(e3)*sin(e4)*sin(e6) - a1*de1*m6*y6*cos(e3)*cos(e5)*sin(e2)*sin(e4)*sin(e6) - a3*de2*m6*y6*cos(e4)*cos(e5)*sin(e2)*sin(e3)*sin(e6) - a3*de3*m6*y6*cos(e4)*cos(e5)*sin(e2)*sin(e3)*sin(e6) - 4*I6zx*de1*cos(e2)*cos(e3)*cos(e4)^2*sin(e2)*sin(e3)*sin(e5)*sin(e6) + d4*de1*m6*y6*cos(e2)*cos(e5)*sin(e2)*sin(e4)*sin(e6) + d4*de1*m6*y6*cos(e3)*cos(e5)*sin(e3)*sin(e4)*sin(e6) + 2*de1*m6*x6*y6*cos(e2)*cos(e3)*cos(e5)*sin(e2)*sin(e3) + 2*de1*m5*x5*z5*cos(e2)*cos(e3)*cos(e5)*sin(e2)*sin(e3) - de1*m6*x6*z6*cos(e2)*cos(e4)*cos(e5)*sin(e2)*sin(e6) - de1*m6*x6*z6*cos(e3)*cos(e4)*cos(e5)*sin(e3)*sin(e6) + 2*de1*m6*x6*z6*cos(e4)*cos(e5)*cos(e6)*sin(e4)*sin(e5) + 2*de2*m5*y5*z5*cos(e2)*cos(e3)*cos(e4)*sin(e4)*sin(e5) + 2*de3*m5*y5*z5*cos(e2)*cos(e3)*cos(e4)*sin(e4)*sin(e5) - de2*m6*y6*z6*cos(e2)*cos(e5)*cos(e6)*sin(e3)*sin(e4) - de2*m6*y6*z6*cos(e3)*cos(e5)*cos(e6)*sin(e2)*sin(e4) - de3*m6*y6*z6*cos(e2)*cos(e5)*cos(e6)*sin(e3)*sin(e4) - de3*m6*y6*z6*cos(e3)*cos(e5)*cos(e6)*sin(e2)*sin(e4) - de5*m6*y6*z6*cos(e2)*cos(e3)*cos(e6)*sin(e4)*sin(e5) - de6*m6*y6*z6*cos(e2)*cos(e5)*cos(e6)*sin(e3)*sin(e5) - de6*m6*y6*z6*cos(e3)*cos(e5)*cos(e6)*sin(e2)*sin(e5) - a2*de1*m5*y5*cos(e2)*sin(e2)*sin(e3)*sin(e4)*sin(e5) - a2*de1*m6*z6*cos(e2)*sin(e2)*sin(e3)*sin(e4)*sin(e5) + de2*m6*x6^2*cos(e2)*cos(e4)*cos(e5)*cos(e6)^2*sin(e3)*sin(e5) + de2*m6*x6^2*cos(e3)*cos(e4)*cos(e5)*cos(e6)^2*sin(e2)*sin(e5) + de3*m6*x6^2*cos(e2)*cos(e4)*cos(e5)*cos(e6)^2*sin(e3)*sin(e5) + de3*m6*x6^2*cos(e3)*cos(e4)*cos(e5)*cos(e6)^2*sin(e2)*sin(e5) - de2*m6*y6^2*cos(e2)*cos(e4)*cos(e5)*cos(e6)^2*sin(e3)*sin(e5) - de2*m6*y6^2*cos(e3)*cos(e4)*cos(e5)*cos(e6)^2*sin(e2)*sin(e5) - de3*m6*y6^2*cos(e2)*cos(e4)*cos(e5)*cos(e6)^2*sin(e3)*sin(e5) - de3*m6*y6^2*cos(e3)*cos(e4)*cos(e5)*cos(e6)^2*sin(e2)*sin(e5) + 2*de2*m6*x6*y6*cos(e4)*cos(e5)*sin(e2)*sin(e3)*sin(e4) + 2*de3*m6*x6*y6*cos(e4)*cos(e5)*sin(e2)*sin(e3)*sin(e4) - 2*de5*m5*x5*y5*cos(e4)*cos(e5)*sin(e2)*sin(e3)*sin(e5) + de6*m6*x6*y6*cos(e4)*cos(e5)*sin(e2)*sin(e3)*sin(e5) + 4*de1*m6*y6*z6*cos(e2)^2*cos(e3)^2*cos(e4)^2*cos(e6)*sin(e5) + 2*de2*m5*x5*z5*cos(e4)*cos(e5)*sin(e2)*sin(e3)*sin(e4) + 2*de3*m5*x5*z5*cos(e4)*cos(e5)*sin(e2)*sin(e3)*sin(e4) - de2*m6*x6*z6*cos(e2)*cos(e5)*sin(e3)*sin(e4)*sin(e6) - de2*m6*x6*z6*cos(e3)*cos(e5)*sin(e2)*sin(e4)*sin(e6) - de3*m6*x6*z6*cos(e2)*cos(e5)*sin(e3)*sin(e4)*sin(e6) - de3*m6*x6*z6*cos(e3)*cos(e5)*sin(e2)*sin(e4)*sin(e6) - de5*m6*x6*z6*cos(e2)*cos(e3)*sin(e4)*sin(e5)*sin(e6) - de6*m6*x6*z6*cos(e2)*cos(e5)*sin(e3)*sin(e5)*sin(e6) - de6*m6*x6*z6*cos(e3)*cos(e5)*sin(e2)*sin(e5)*sin(e6) - 2*de1*m5*y5*z5*cos(e2)*cos(e3)*sin(e2)*sin(e3)*sin(e5) - 2*de1*m6*y6*z6*cos(e4)*cos(e5)*sin(e4)*sin(e5)*sin(e6) - 2*de1*m6*x6^2*cos(e2)^2*cos(e3)^2*cos(e4)*cos(e5)^2*cos(e6)^2*sin(e4) + 2*de1*m6*y6^2*cos(e2)^2*cos(e3)^2*cos(e4)*cos(e5)^2*cos(e6)^2*sin(e4) + 2*de1*m5*x5^2*cos(e2)*cos(e3)^2*cos(e5)*sin(e2)*sin(e4)*sin(e5) + 2*de1*m5*x5^2*cos(e2)^2*cos(e3)*cos(e5)*sin(e3)*sin(e4)*sin(e5) - de1*m6*x6^2*cos(e2)*cos(e5)*cos(e6)^2*sin(e2)*sin(e4)*sin(e5) - de1*m6*x6^2*cos(e3)*cos(e5)*cos(e6)^2*sin(e3)*sin(e4)*sin(e5) - 2*de1*m5*y5^2*cos(e2)*cos(e3)^2*cos(e5)*sin(e2)*sin(e4)*sin(e5) - 2*de1*m5*y5^2*cos(e2)^2*cos(e3)*cos(e5)*sin(e3)*sin(e4)*sin(e5) + 2*de1*m6*y6^2*cos(e2)*cos(e3)^2*cos(e5)*sin(e2)*sin(e4)*sin(e5) + 2*de1*m6*y6^2*cos(e2)^2*cos(e3)*cos(e5)*sin(e3)*sin(e4)*sin(e5) + de1*m6*y6^2*cos(e2)*cos(e5)*cos(e6)^2*sin(e2)*sin(e4)*sin(e5) + de1*m6*y6^2*cos(e3)*cos(e5)*cos(e6)^2*sin(e3)*sin(e4)*sin(e5) + 4*de1*m6*x6*z6*cos(e2)^2*cos(e3)^2*cos(e4)^2*sin(e5)*sin(e6) - 2*de1*m6*z6^2*cos(e2)*cos(e3)^2*cos(e5)*sin(e2)*sin(e4)*sin(e5) - 2*de1*m6*z6^2*cos(e2)^2*cos(e3)*cos(e5)*sin(e3)*sin(e4)*sin(e5) - 2*de2*m5*y5*z5*cos(e4)*sin(e2)*sin(e3)*sin(e4)*sin(e5) - 2*de3*m5*y5*z5*cos(e4)*sin(e2)*sin(e3)*sin(e4)*sin(e5) + de5*m6*y6*z6*cos(e6)*sin(e2)*sin(e3)*sin(e4)*sin(e5) + de5*m6*x6*z6*sin(e2)*sin(e3)*sin(e4)*sin(e5)*sin(e6) - a2*de1*m6*x6*cos(e2)^2*cos(e3)*cos(e5)*cos(e6)*sin(e4) + 8*I6xy*de1*cos(e2)*cos(e3)*cos(e4)^2*cos(e5)*cos(e6)^2*sin(e2)*sin(e3) + 4*I6zx*de1*cos(e2)^2*cos(e3)^2*cos(e4)*cos(e5)*cos(e6)*sin(e4)*sin(e5) + 2*d4*de1*m6*y6*cos(e2)*cos(e3)^2*cos(e4)*cos(e6)*sin(e2) + 2*d4*de1*m6*y6*cos(e2)^2*cos(e3)*cos(e4)*cos(e6)*sin(e3) + de6*m6*y6*z6*cos(e2)*cos(e3)*cos(e4)*cos(e5)^2*cos(e6) + a2*de1*m6*y6*cos(e2)^2*cos(e3)*cos(e5)*sin(e4)*sin(e6) + 2*d4*de1*m5*x5*cos(e2)*cos(e3)^2*cos(e5)*sin(e2)*sin(e4) + 2*d4*de1*m5*x5*cos(e2)^2*cos(e3)*cos(e5)*sin(e3)*sin(e4) + 2*d4*de1*m6*x6*cos(e2)*cos(e3)^2*cos(e4)*sin(e2)*sin(e6) + 2*d4*de1*m6*x6*cos(e2)^2*cos(e3)*cos(e4)*sin(e3)*sin(e6) - 2*I6xx*de1*cos(e2)*cos(e3)^2*cos(e5)*cos(e6)^2*sin(e2)*sin(e4)*sin(e5) - 2*I6xx*de1*cos(e2)^2*cos(e3)*cos(e5)*cos(e6)^2*sin(e3)*sin(e4)*sin(e5) + 2*I6yy*de1*cos(e2)*cos(e3)^2*cos(e5)*cos(e6)^2*sin(e2)*sin(e4)*sin(e5) + 2*I6yy*de1*cos(e2)^2*cos(e3)*cos(e5)*cos(e6)^2*sin(e3)*sin(e4)*sin(e5) - 4*I6yz*de1*cos(e2)^2*cos(e3)^2*cos(e4)*cos(e5)*sin(e4)*sin(e5)*sin(e6) + 2*de2*m5*x5*y5*cos(e2)*cos(e3)*cos(e4)^2*cos(e5)*sin(e5) + 2*de3*m5*x5*y5*cos(e2)*cos(e3)*cos(e4)^2*cos(e5)*sin(e5) + 2*de2*m6*x6*y6*cos(e2)*cos(e3)*cos(e4)^2*cos(e6)*sin(e6) + 2*de3*m6*x6*y6*cos(e2)*cos(e3)*cos(e4)^2*cos(e6)*sin(e6) + 2*de5*m6*x6*y6*cos(e2)*cos(e3)*cos(e5)*cos(e6)^2*sin(e4) + 2*de2*m6*x6*z6*cos(e2)*cos(e4)*cos(e5)^2*cos(e6)*sin(e3) + 2*de2*m6*x6*z6*cos(e3)*cos(e4)*cos(e5)^2*cos(e6)*sin(e2) + 2*de3*m6*x6*z6*cos(e2)*cos(e4)*cos(e5)^2*cos(e6)*sin(e3) + 2*de3*m6*x6*z6*cos(e3)*cos(e4)*cos(e5)^2*cos(e6)*sin(e2) + de6*m6*x6*z6*cos(e2)*cos(e3)*cos(e4)*cos(e5)^2*sin(e6) - 2*de1*m5*y5*z5*cos(e2)*cos(e3)^2*cos(e4)*cos(e5)*sin(e2) - 2*de1*m5*y5*z5*cos(e2)^2*cos(e3)*cos(e4)*cos(e5)*sin(e3) - 2*d4*de1*m5*y5*cos(e2)*cos(e3)^2*sin(e2)*sin(e4)*sin(e5) - 2*d4*de1*m5*y5*cos(e2)^2*cos(e3)*sin(e3)*sin(e4)*sin(e5) - 2*d4*de1*m6*z6*cos(e2)*cos(e3)^2*sin(e2)*sin(e4)*sin(e5) - 2*d4*de1*m6*z6*cos(e2)^2*cos(e3)*sin(e3)*sin(e4)*sin(e5) - 8*de1*m6*x6*y6*cos(e2)^2*cos(e3)^2*cos(e4)^2*cos(e5)*cos(e6)^2 + 4*de1*m4*x4*y4*cos(e2)*cos(e3)*cos(e4)^2*sin(e2)*sin(e3) - 2*de1*m6*x6*y6*cos(e2)*cos(e3)^2*cos(e4)*sin(e2)*sin(e5) - 2*de1*m5*x5*y5*cos(e2)^2*cos(e4)*cos(e5)*sin(e4)*sin(e5) - 2*de1*m6*x6*y6*cos(e2)^2*cos(e3)*cos(e4)*sin(e3)*sin(e5) - 2*de1*m5*x5*y5*cos(e3)^2*cos(e4)*cos(e5)*sin(e4)*sin(e5) - 2*de1*m6*x6*y6*cos(e2)*cos(e4)*cos(e6)^2*sin(e2)*sin(e5) - 2*de1*m6*x6*y6*cos(e3)*cos(e4)*cos(e6)^2*sin(e3)*sin(e5) - 2*de1*m6*x6*y6*cos(e2)^2*cos(e4)*cos(e6)*sin(e4)*sin(e6) - 2*de1*m6*x6*y6*cos(e3)^2*cos(e4)*cos(e6)*sin(e4)*sin(e6) + 2*de1*m6*x6*y6*cos(e4)*cos(e5)^2*cos(e6)*sin(e4)*sin(e6) - 2*de1*m5*x5*z5*cos(e2)*cos(e3)^2*cos(e4)*sin(e2)*sin(e5) - 2*de1*m5*x5*z5*cos(e2)^2*cos(e3)*cos(e4)*sin(e3)*sin(e5) - 2*de1*m6*x6*z6*cos(e2)*cos(e3)^2*cos(e6)*sin(e2)*sin(e4) - 2*de1*m6*x6*z6*cos(e2)^2*cos(e3)*cos(e6)*sin(e3)*sin(e4) - 2*de1*m6*x6*z6*cos(e2)*cos(e5)^2*cos(e6)*sin(e2)*sin(e4) - 2*de1*m6*x6*z6*cos(e3)*cos(e5)^2*cos(e6)*sin(e3)*sin(e4) - 2*de2*m6*y6*z6*cos(e2)*cos(e4)*cos(e5)^2*sin(e3)*sin(e6) - 2*de2*m6*y6*z6*cos(e3)*cos(e4)*cos(e5)^2*sin(e2)*sin(e6) - 2*de3*m6*y6*z6*cos(e2)*cos(e4)*cos(e5)^2*sin(e3)*sin(e6) - 2*de3*m6*y6*z6*cos(e3)*cos(e4)*cos(e5)^2*sin(e2)*sin(e6) - de6*m6*y6*z6*cos(e4)*cos(e5)^2*cos(e6)*sin(e2)*sin(e3) - 2*de2*m5*x5*y5*cos(e4)^2*cos(e5)*sin(e2)*sin(e3)*sin(e5) - 2*de3*m5*x5*y5*cos(e4)^2*cos(e5)*sin(e2)*sin(e3)*sin(e5) - 2*de2*m6*x6*y6*cos(e2)*cos(e6)^2*sin(e3)*sin(e4)*sin(e5) - 2*de2*m6*x6*y6*cos(e3)*cos(e6)^2*sin(e2)*sin(e4)*sin(e5) - 2*de2*m6*x6*y6*cos(e4)^2*cos(e6)*sin(e2)*sin(e3)*sin(e6) - 2*de3*m6*x6*y6*cos(e2)*cos(e6)^2*sin(e3)*sin(e4)*sin(e5) - 2*de3*m6*x6*y6*cos(e3)*cos(e6)^2*sin(e2)*sin(e4)*sin(e5) - 2*de3*m6*x6*y6*cos(e4)^2*cos(e6)*sin(e2)*sin(e3)*sin(e6) - 2*de5*m6*x6*y6*cos(e5)*cos(e6)^2*sin(e2)*sin(e3)*sin(e4) - de6*m6*x6*z6*cos(e4)*cos(e5)^2*sin(e2)*sin(e3)*sin(e6) + 2*de1*m6*y6*z6*cos(e2)*cos(e3)^2*sin(e2)*sin(e4)*sin(e6) + 2*de1*m6*y6*z6*cos(e2)^2*cos(e3)*sin(e3)*sin(e4)*sin(e6) + 2*de1*m6*y6*z6*cos(e2)*cos(e5)^2*sin(e2)*sin(e4)*sin(e6) + 2*de1*m6*y6*z6*cos(e3)*cos(e5)^2*sin(e3)*sin(e4)*sin(e6) - 2*I6xx*de2*cos(e2)*cos(e3)*cos(e4)*cos(e5)*cos(e6)*sin(e4)*sin(e6) - 2*I6xx*de3*cos(e2)*cos(e3)*cos(e4)*cos(e5)*cos(e6)*sin(e4)*sin(e6) - I6xx*de6*cos(e2)*cos(e3)*cos(e4)*cos(e5)*cos(e6)*sin(e5)*sin(e6) + 2*I6yy*de2*cos(e2)*cos(e3)*cos(e4)*cos(e5)*cos(e6)*sin(e4)*sin(e6) + 2*I6yy*de3*cos(e2)*cos(e3)*cos(e4)*cos(e5)*cos(e6)*sin(e4)*sin(e6) + I6yy*de6*cos(e2)*cos(e3)*cos(e4)*cos(e5)*cos(e6)*sin(e5)*sin(e6) + 2*I6xx*de1*cos(e2)*cos(e3)*cos(e5)*cos(e6)*sin(e2)*sin(e3)*sin(e6) - 2*I6xy*de2*cos(e2)*cos(e4)*cos(e5)*cos(e6)*sin(e3)*sin(e5)*sin(e6) - 2*I6xy*de2*cos(e3)*cos(e4)*cos(e5)*cos(e6)*sin(e2)*sin(e5)*sin(e6) - 2*I6xy*de3*cos(e2)*cos(e4)*cos(e5)*cos(e6)*sin(e3)*sin(e5)*sin(e6) - 2*I6xy*de3*cos(e3)*cos(e4)*cos(e5)*cos(e6)*sin(e2)*sin(e5)*sin(e6) - 2*I6yy*de1*cos(e2)*cos(e3)*cos(e5)*cos(e6)*sin(e2)*sin(e3)*sin(e6) - 2*a3*de1*m6*x6*cos(e2)^2*cos(e3)^2*cos(e5)*cos(e6)*sin(e4) + 4*I6xy*de1*cos(e2)^2*cos(e3)^2*cos(e4)*cos(e5)^2*cos(e6)*sin(e4)*sin(e6) + 2*I6xx*de2*cos(e4)*cos(e5)*cos(e6)*sin(e2)*sin(e3)*sin(e4)*sin(e6) + 2*I6xy*de1*cos(e2)*cos(e5)*cos(e6)*sin(e2)*sin(e4)*sin(e5)*sin(e6) + 2*I6xx*de3*cos(e4)*cos(e5)*cos(e6)*sin(e2)*sin(e3)*sin(e4)*sin(e6) + 2*I6xy*de1*cos(e3)*cos(e5)*cos(e6)*sin(e3)*sin(e4)*sin(e5)*sin(e6) + I6xx*de6*cos(e4)*cos(e5)*cos(e6)*sin(e2)*sin(e3)*sin(e5)*sin(e6) - 2*I6yy*de2*cos(e4)*cos(e5)*cos(e6)*sin(e2)*sin(e3)*sin(e4)*sin(e6) - 2*I6yy*de3*cos(e4)*cos(e5)*cos(e6)*sin(e2)*sin(e3)*sin(e4)*sin(e6) - I6yy*de6*cos(e4)*cos(e5)*cos(e6)*sin(e2)*sin(e3)*sin(e5)*sin(e6) + 2*a3*de1*m6*y6*cos(e2)^2*cos(e3)^2*cos(e5)*sin(e4)*sin(e6) + de5*m6*x6^2*cos(e2)*cos(e3)*cos(e5)*cos(e6)*sin(e4)*sin(e6) - de5*m6*y6^2*cos(e2)*cos(e3)*cos(e5)*cos(e6)*sin(e4)*sin(e6) - 4*de1*m6*x6^2*cos(e2)^2*cos(e3)^2*cos(e4)^2*cos(e5)*cos(e6)*sin(e6) + 4*de1*m6*y6^2*cos(e2)^2*cos(e3)^2*cos(e4)^2*cos(e5)*cos(e6)*sin(e6) + 2*de1*m4*x4^2*cos(e2)*cos(e3)*cos(e4)*sin(e2)*sin(e3)*sin(e4) - 2*de1*m6*x6^2*cos(e2)*cos(e3)*cos(e4)*sin(e2)*sin(e3)*sin(e4) - de1*m6*x6^2*cos(e2)*cos(e4)*cos(e6)*sin(e2)*sin(e5)*sin(e6) - de1*m6*x6^2*cos(e3)*cos(e4)*cos(e6)*sin(e3)*sin(e5)*sin(e6) + 4*de1*m5*x5*y5*cos(e2)*cos(e3)^2*cos(e5)^2*sin(e2)*sin(e4) + 4*de1*m5*x5*y5*cos(e2)^2*cos(e3)*cos(e5)^2*sin(e3)*sin(e4) - 2*de1*m4*y4^2*cos(e2)*cos(e3)*cos(e4)*sin(e2)*sin(e3)*sin(e4) + 2*de1*m5*y5^2*cos(e2)*cos(e3)*cos(e4)*sin(e2)*sin(e3)*sin(e4) + de1*m6*y6^2*cos(e2)*cos(e4)*cos(e6)*sin(e2)*sin(e5)*sin(e6) + de1*m6*y6^2*cos(e3)*cos(e4)*cos(e6)*sin(e3)*sin(e5)*sin(e6) - 2*de1*m5*z5^2*cos(e2)*cos(e3)*cos(e4)*sin(e2)*sin(e3)*sin(e4) + 2*de1*m6*z6^2*cos(e2)*cos(e3)*cos(e4)*sin(e2)*sin(e3)*sin(e4) - a3*de2*m6*x6*cos(e2)*cos(e3)*cos(e4)*cos(e5)*cos(e6) - a3*de3*m6*x6*cos(e2)*cos(e3)*cos(e4)*cos(e5)*cos(e6) - de2*m6*x6^2*cos(e2)*cos(e6)*sin(e3)*sin(e4)*sin(e5)*sin(e6) - de2*m6*x6^2*cos(e3)*cos(e6)*sin(e2)*sin(e4)*sin(e5)*sin(e6) - de3*m6*x6^2*cos(e2)*cos(e6)*sin(e3)*sin(e4)*sin(e5)*sin(e6) - de3*m6*x6^2*cos(e3)*cos(e6)*sin(e2)*sin(e4)*sin(e5)*sin(e6) - de5*m6*x6^2*cos(e5)*cos(e6)*sin(e2)*sin(e3)*sin(e4)*sin(e6) + de2*m6*y6^2*cos(e2)*cos(e6)*sin(e3)*sin(e4)*sin(e5)*sin(e6) + de2*m6*y6^2*cos(e3)*cos(e6)*sin(e2)*sin(e4)*sin(e5)*sin(e6) + de3*m6*y6^2*cos(e2)*cos(e6)*sin(e3)*sin(e4)*sin(e5)*sin(e6) + de3*m6*y6^2*cos(e3)*cos(e6)*sin(e2)*sin(e4)*sin(e5)*sin(e6) + de5*m6*y6^2*cos(e5)*cos(e6)*sin(e2)*sin(e3)*sin(e4)*sin(e6) - 2*de5*m6*x6*y6*cos(e2)*cos(e5)*cos(e6)*sin(e3)*sin(e5)*sin(e6) - 2*de5*m6*x6*y6*cos(e3)*cos(e5)*cos(e6)*sin(e2)*sin(e5)*sin(e6) - 2*de6*m6*x6*y6*cos(e2)*cos(e3)*cos(e6)*sin(e4)*sin(e5)*sin(e6) - 2*de2*m6*x6*z6*cos(e2)*cos(e3)*cos(e4)*sin(e4)*sin(e5)*sin(e6) - 2*de3*m6*x6*z6*cos(e2)*cos(e3)*cos(e4)*sin(e4)*sin(e5)*sin(e6) - 2*de5*m6*x6*z6*cos(e4)*cos(e5)*cos(e6)*sin(e2)*sin(e3)*sin(e5) + 2*de1*m6*y6*z6*cos(e2)*cos(e3)*cos(e6)*sin(e2)*sin(e3)*sin(e5) + 2*de1*m5*x5^2*cos(e2)*cos(e3)*cos(e4)*cos(e5)^2*sin(e2)*sin(e3)*sin(e4) + 2*de1*m6*x6^2*cos(e2)*cos(e3)*cos(e4)*cos(e6)^2*sin(e2)*sin(e3)*sin(e4) + 2*de1*m6*x6^2*cos(e2)*cos(e3)^2*cos(e4)*cos(e6)*sin(e2)*sin(e5)*sin(e6) + 2*de1*m6*x6^2*cos(e2)^2*cos(e3)*cos(e4)*cos(e6)*sin(e3)*sin(e5)*sin(e6) - 2*de1*m5*y5^2*cos(e2)*cos(e3)*cos(e4)*cos(e5)^2*sin(e2)*sin(e3)*sin(e4) + 2*de1*m6*y6^2*cos(e2)*cos(e3)*cos(e4)*cos(e5)^2*sin(e2)*sin(e3)*sin(e4) - 2*de1*m6*y6^2*cos(e2)*cos(e3)*cos(e4)*cos(e6)^2*sin(e2)*sin(e3)*sin(e4) - 2*de1*m6*y6^2*cos(e2)*cos(e3)^2*cos(e4)*cos(e6)*sin(e2)*sin(e5)*sin(e6) - 2*de1*m6*y6^2*cos(e2)^2*cos(e3)*cos(e4)*cos(e6)*sin(e3)*sin(e5)*sin(e6) - 2*de1*m6*z6^2*cos(e2)*cos(e3)*cos(e4)*cos(e5)^2*sin(e2)*sin(e3)*sin(e4) + 2*de1*m6*x6*z6*cos(e2)*cos(e3)*sin(e2)*sin(e3)*sin(e5)*sin(e6) + 2*de2*m6*y6*z6*cos(e4)*cos(e6)*sin(e2)*sin(e3)*sin(e4)*sin(e5) + 2*de3*m6*y6*z6*cos(e4)*cos(e6)*sin(e2)*sin(e3)*sin(e4)*sin(e5) + 2*de5*m6*y6*z6*cos(e4)*cos(e5)*sin(e2)*sin(e3)*sin(e5)*sin(e6) + 2*de6*m6*x6*y6*cos(e6)*sin(e2)*sin(e3)*sin(e4)*sin(e5)*sin(e6) + 2*de2*m6*x6*z6*cos(e4)*sin(e2)*sin(e3)*sin(e4)*sin(e5)*sin(e6) + 2*de3*m6*x6*z6*cos(e4)*sin(e2)*sin(e3)*sin(e4)*sin(e5)*sin(e6) + 2*d4*de1*m6*x6*cos(e2)*cos(e3)^2*cos(e5)*cos(e6)*sin(e2)*sin(e4) + 2*d4*de1*m6*x6*cos(e2)^2*cos(e3)*cos(e5)*cos(e6)*sin(e3)*sin(e4) - 2*I6xx*de1*cos(e2)*cos(e3)*cos(e4)*cos(e5)^2*cos(e6)^2*sin(e2)*sin(e3)*sin(e4) + 2*I6yy*de1*cos(e2)*cos(e3)*cos(e4)*cos(e5)^2*cos(e6)^2*sin(e2)*sin(e3)*sin(e4) + 4*de2*m6*x6*y6*cos(e2)*cos(e3)*cos(e4)*cos(e5)*cos(e6)^2*sin(e4) + 4*de3*m6*x6*y6*cos(e2)*cos(e3)*cos(e4)*cos(e5)*cos(e6)^2*sin(e4) + 2*de5*m6*x6*y6*cos(e2)*cos(e3)*cos(e4)*cos(e5)^2*cos(e6)*sin(e6) + 2*de6*m6*x6*y6*cos(e2)*cos(e3)*cos(e4)*cos(e5)*cos(e6)^2*sin(e5) + 2*de2*m6*x6*z6*cos(e2)*cos(e3)*cos(e4)^2*cos(e5)*cos(e6)*sin(e5) + 2*de3*m6*x6*z6*cos(e2)*cos(e3)*cos(e4)^2*cos(e5)*cos(e6)*sin(e5) + 2*de1*m6*y6*z6*cos(e2)*cos(e3)^2*cos(e4)*cos(e5)*cos(e6)*sin(e2) + 2*de1*m6*y6*z6*cos(e2)^2*cos(e3)*cos(e4)*cos(e5)*cos(e6)*sin(e3) - 2*d4*de1*m6*y6*cos(e2)*cos(e3)^2*cos(e5)*sin(e2)*sin(e4)*sin(e6) - 2*d4*de1*m6*y6*cos(e2)^2*cos(e3)*cos(e5)*sin(e3)*sin(e4)*sin(e6) - 4*de1*m6*x6*y6*cos(e2)*cos(e3)*cos(e4)^2*cos(e5)*sin(e2)*sin(e3) - 4*de1*m6*x6*y6*cos(e2)*cos(e3)*cos(e5)*cos(e6)^2*sin(e2)*sin(e3) - 4*de1*m5*x5*z5*cos(e2)*cos(e3)*cos(e4)^2*cos(e5)*sin(e2)*sin(e3) + 2*de1*m6*x6*z6*cos(e2)*cos(e3)^2*cos(e4)*cos(e5)*sin(e2)*sin(e6) + 2*de1*m6*x6*z6*cos(e2)^2*cos(e3)*cos(e4)*cos(e5)*sin(e3)*sin(e6) - 2*de1*m6*x6*z6*cos(e2)^2*cos(e4)*cos(e5)*cos(e6)*sin(e4)*sin(e5) - 2*de1*m6*x6*z6*cos(e3)^2*cos(e4)*cos(e5)*cos(e6)*sin(e4)*sin(e5) - 2*de2*m6*y6*z6*cos(e2)*cos(e3)*cos(e4)^2*cos(e5)*sin(e5)*sin(e6) - 2*de3*m6*y6*z6*cos(e2)*cos(e3)*cos(e4)^2*cos(e5)*sin(e5)*sin(e6) - 4*de2*m6*x6*y6*cos(e4)*cos(e5)*cos(e6)^2*sin(e2)*sin(e3)*sin(e4) - 4*de3*m6*x6*y6*cos(e4)*cos(e5)*cos(e6)^2*sin(e2)*sin(e3)*sin(e4) - 2*de5*m6*x6*y6*cos(e4)*cos(e5)^2*cos(e6)*sin(e2)*sin(e3)*sin(e6) - 2*de6*m6*x6*y6*cos(e4)*cos(e5)*cos(e6)^2*sin(e2)*sin(e3)*sin(e5) - 2*de2*m6*x6*z6*cos(e4)^2*cos(e5)*cos(e6)*sin(e2)*sin(e3)*sin(e5) - 2*de3*m6*x6*z6*cos(e4)^2*cos(e5)*cos(e6)*sin(e2)*sin(e3)*sin(e5) + 4*de1*m5*y5*z5*cos(e2)*cos(e3)*cos(e4)^2*sin(e2)*sin(e3)*sin(e5) + 2*de1*m6*y6*z6*cos(e2)^2*cos(e4)*cos(e5)*sin(e4)*sin(e5)*sin(e6) + 2*de1*m6*y6*z6*cos(e3)^2*cos(e4)*cos(e5)*sin(e4)*sin(e5)*sin(e6) + 2*de1*m6*x6^2*cos(e2)*cos(e3)^2*cos(e5)*cos(e6)^2*sin(e2)*sin(e4)*sin(e5) + 2*de1*m6*x6^2*cos(e2)^2*cos(e3)*cos(e5)*cos(e6)^2*sin(e3)*sin(e4)*sin(e5) - 2*de1*m6*y6^2*cos(e2)*cos(e3)^2*cos(e5)*cos(e6)^2*sin(e2)*sin(e4)*sin(e5) - 2*de1*m6*y6^2*cos(e2)^2*cos(e3)*cos(e5)*cos(e6)^2*sin(e3)*sin(e4)*sin(e5) + 2*de2*m6*y6*z6*cos(e4)^2*cos(e5)*sin(e2)*sin(e3)*sin(e5)*sin(e6) + 2*de3*m6*y6*z6*cos(e4)^2*cos(e5)*sin(e2)*sin(e3)*sin(e5)*sin(e6) - 4*I5xy*de1*cos(e2)*cos(e3)*cos(e4)*cos(e5)*sin(e2)*sin(e3)*sin(e4)*sin(e5) - 4*I6xy*de1*cos(e2)*cos(e3)*cos(e4)*cos(e6)*sin(e2)*sin(e3)*sin(e4)*sin(e6) + 2*de2*m6*x6^2*cos(e2)*cos(e3)*cos(e4)*cos(e5)*cos(e6)*sin(e4)*sin(e6) + 2*de3*m6*x6^2*cos(e2)*cos(e3)*cos(e4)*cos(e5)*cos(e6)*sin(e4)*sin(e6) + de6*m6*x6^2*cos(e2)*cos(e3)*cos(e4)*cos(e5)*cos(e6)*sin(e5)*sin(e6) + 2*de2*m6*x6*y6*cos(e2)*cos(e3)*cos(e4)^2*cos(e5)^2*cos(e6)*sin(e6) + 2*de3*m6*x6*y6*cos(e2)*cos(e3)*cos(e4)^2*cos(e5)^2*cos(e6)*sin(e6) - 2*de2*m6*y6^2*cos(e2)*cos(e3)*cos(e4)*cos(e5)*cos(e6)*sin(e4)*sin(e6) - 2*de3*m6*y6^2*cos(e2)*cos(e3)*cos(e4)*cos(e5)*cos(e6)*sin(e4)*sin(e6) - de6*m6*y6^2*cos(e2)*cos(e3)*cos(e4)*cos(e5)*cos(e6)*sin(e5)*sin(e6) - 2*de1*m6*x6^2*cos(e2)*cos(e3)*cos(e5)*cos(e6)*sin(e2)*sin(e3)*sin(e6) + 4*de1*m5*x5*y5*cos(e2)^2*cos(e3)^2*cos(e4)*cos(e5)*sin(e4)*sin(e5) + 4*de1*m6*x6*y6*cos(e2)*cos(e3)^2*cos(e4)*cos(e6)^2*sin(e2)*sin(e5) + 4*de1*m6*x6*y6*cos(e2)^2*cos(e3)*cos(e4)*cos(e6)^2*sin(e3)*sin(e5) + 4*de1*m6*x6*y6*cos(e2)^2*cos(e3)^2*cos(e4)*cos(e6)*sin(e4)*sin(e6) - 2*de1*m6*x6*y6*cos(e2)^2*cos(e4)*cos(e5)^2*cos(e6)*sin(e4)*sin(e6) - 2*de1*m6*x6*y6*cos(e3)^2*cos(e4)*cos(e5)^2*cos(e6)*sin(e4)*sin(e6) + 2*de1*m6*y6^2*cos(e2)*cos(e3)*cos(e5)*cos(e6)*sin(e2)*sin(e3)*sin(e6) + 4*de1*m6*x6*z6*cos(e2)*cos(e3)^2*cos(e5)^2*cos(e6)*sin(e2)*sin(e4) + 4*de1*m6*x6*z6*cos(e2)^2*cos(e3)*cos(e5)^2*cos(e6)*sin(e3)*sin(e4) - 2*de2*m6*x6^2*cos(e4)*cos(e5)*cos(e6)*sin(e2)*sin(e3)*sin(e4)*sin(e6) - 2*de3*m6*x6^2*cos(e4)*cos(e5)*cos(e6)*sin(e2)*sin(e3)*sin(e4)*sin(e6) - de6*m6*x6^2*cos(e4)*cos(e5)*cos(e6)*sin(e2)*sin(e3)*sin(e5)*sin(e6) - 2*de2*m6*x6*y6*cos(e4)^2*cos(e5)^2*cos(e6)*sin(e2)*sin(e3)*sin(e6) - 2*de3*m6*x6*y6*cos(e4)^2*cos(e5)^2*cos(e6)*sin(e2)*sin(e3)*sin(e6) + 2*de2*m6*y6^2*cos(e4)*cos(e5)*cos(e6)*sin(e2)*sin(e3)*sin(e4)*sin(e6) + 2*de3*m6*y6^2*cos(e4)*cos(e5)*cos(e6)*sin(e2)*sin(e3)*sin(e4)*sin(e6) + de6*m6*y6^2*cos(e4)*cos(e5)*cos(e6)*sin(e2)*sin(e3)*sin(e5)*sin(e6) - 4*de1*m6*y6*z6*cos(e2)*cos(e3)^2*cos(e5)^2*sin(e2)*sin(e4)*sin(e6) - 4*de1*m6*y6*z6*cos(e2)^2*cos(e3)*cos(e5)^2*sin(e3)*sin(e4)*sin(e6) + 2*a3*de1*m6*y6*cos(e2)*cos(e3)*cos(e4)*cos(e6)*sin(e2)*sin(e3) - 4*I6xx*de1*cos(e2)*cos(e3)*cos(e4)^2*cos(e5)*cos(e6)*sin(e2)*sin(e3)*sin(e6) + 4*I6yy*de1*cos(e2)*cos(e3)*cos(e4)^2*cos(e5)*cos(e6)*sin(e2)*sin(e3)*sin(e6) + 2*de5*m6*x6*z6*cos(e2)*cos(e3)*cos(e4)*cos(e5)*cos(e6)*sin(e5) + 2*a3*de1*m5*x5*cos(e2)*cos(e3)*cos(e5)*sin(e2)*sin(e3)*sin(e4) + 2*a3*de1*m6*x6*cos(e2)*cos(e3)*cos(e4)*sin(e2)*sin(e3)*sin(e6) + a2*de1*m6*x6*cos(e2)*cos(e5)*cos(e6)*sin(e2)*sin(e3)*sin(e4) - 4*I6xy*de1*cos(e2)*cos(e3)^2*cos(e5)*cos(e6)*sin(e2)*sin(e4)*sin(e5)*sin(e6) - 4*I6xy*de1*cos(e2)^2*cos(e3)*cos(e5)*cos(e6)*sin(e3)*sin(e4)*sin(e5)*sin(e6) - 2*de2*m6*y6*z6*cos(e2)*cos(e3)*cos(e4)*cos(e6)*sin(e4)*sin(e5) - 2*de3*m6*y6*z6*cos(e2)*cos(e3)*cos(e4)*cos(e6)*sin(e4)*sin(e5) - 2*de5*m6*y6*z6*cos(e2)*cos(e3)*cos(e4)*cos(e5)*sin(e5)*sin(e6) - 2*a3*de1*m5*y5*cos(e2)*cos(e3)*sin(e2)*sin(e3)*sin(e4)*sin(e5) - a2*de1*m6*y6*cos(e2)*cos(e5)*sin(e2)*sin(e3)*sin(e4)*sin(e6) - 2*a3*de1*m6*z6*cos(e2)*cos(e3)*sin(e2)*sin(e3)*sin(e4)*sin(e5) - 4*de1*m6*y6*z6*cos(e2)*cos(e3)*cos(e4)^2*cos(e6)*sin(e2)*sin(e3)*sin(e5) + 2*de1*m6*x6^2*cos(e2)*cos(e3)*cos(e4)*cos(e5)^2*cos(e6)^2*sin(e2)*sin(e3)*sin(e4) - 2*de1*m6*y6^2*cos(e2)*cos(e3)*cos(e4)*cos(e5)^2*cos(e6)^2*sin(e2)*sin(e3)*sin(e4) - 4*de1*m6*x6*z6*cos(e2)*cos(e3)*cos(e4)^2*sin(e2)*sin(e3)*sin(e5)*sin(e6) - 4*I6zx*de1*cos(e2)*cos(e3)*cos(e4)*cos(e5)*cos(e6)*sin(e2)*sin(e3)*sin(e4)*sin(e5) + 4*I6yz*de1*cos(e2)*cos(e3)*cos(e4)*cos(e5)*sin(e2)*sin(e3)*sin(e4)*sin(e5)*sin(e6) + 8*de1*m6*x6*y6*cos(e2)*cos(e3)*cos(e4)^2*cos(e5)*cos(e6)^2*sin(e2)*sin(e3) + 4*de1*m6*x6*z6*cos(e2)^2*cos(e3)^2*cos(e4)*cos(e5)*cos(e6)*sin(e4)*sin(e5) - 4*de1*m6*y6*z6*cos(e2)^2*cos(e3)^2*cos(e4)*cos(e5)*sin(e4)*sin(e5)*sin(e6) + 2*a3*de1*m6*x6*cos(e2)*cos(e3)*cos(e5)*cos(e6)*sin(e2)*sin(e3)*sin(e4) - 4*I6xy*de1*cos(e2)*cos(e3)*cos(e4)*cos(e5)^2*cos(e6)*sin(e2)*sin(e3)*sin(e4)*sin(e6) - 2*a3*de1*m6*y6*cos(e2)*cos(e3)*cos(e5)*sin(e2)*sin(e3)*sin(e4)*sin(e6) - 2*de2*m6*x6*y6*cos(e2)*cos(e4)*cos(e5)*cos(e6)*sin(e3)*sin(e5)*sin(e6) - 2*de2*m6*x6*y6*cos(e3)*cos(e4)*cos(e5)*cos(e6)*sin(e2)*sin(e5)*sin(e6) - 2*de3*m6*x6*y6*cos(e2)*cos(e4)*cos(e5)*cos(e6)*sin(e3)*sin(e5)*sin(e6) - 2*de3*m6*x6*y6*cos(e3)*cos(e4)*cos(e5)*cos(e6)*sin(e2)*sin(e5)*sin(e6) + 4*de1*m6*x6^2*cos(e2)*cos(e3)*cos(e4)^2*cos(e5)*cos(e6)*sin(e2)*sin(e3)*sin(e6) + 4*de1*m6*x6*y6*cos(e2)^2*cos(e3)^2*cos(e4)*cos(e5)^2*cos(e6)*sin(e4)*sin(e6) - 4*de1*m6*y6^2*cos(e2)*cos(e3)*cos(e4)^2*cos(e5)*cos(e6)*sin(e2)*sin(e3)*sin(e6) + 2*de1*m6*x6*y6*cos(e2)*cos(e5)*cos(e6)*sin(e2)*sin(e4)*sin(e5)*sin(e6) + 2*de1*m6*x6*y6*cos(e3)*cos(e5)*cos(e6)*sin(e3)*sin(e4)*sin(e5)*sin(e6) - 4*de1*m6*x6*y6*cos(e2)*cos(e3)^2*cos(e5)*cos(e6)*sin(e2)*sin(e4)*sin(e5)*sin(e6) - 4*de1*m6*x6*y6*cos(e2)^2*cos(e3)*cos(e5)*cos(e6)*sin(e3)*sin(e4)*sin(e5)*sin(e6) - 4*de1*m5*x5*y5*cos(e2)*cos(e3)*cos(e4)*cos(e5)*sin(e2)*sin(e3)*sin(e4)*sin(e5) - 4*de1*m6*x6*y6*cos(e2)*cos(e3)*cos(e4)*cos(e6)*sin(e2)*sin(e3)*sin(e4)*sin(e6) - 4*de1*m6*x6*z6*cos(e2)*cos(e3)*cos(e4)*cos(e5)*cos(e6)*sin(e2)*sin(e3)*sin(e4)*sin(e5) + 4*de1*m6*y6*z6*cos(e2)*cos(e3)*cos(e4)*cos(e5)*sin(e2)*sin(e3)*sin(e4)*sin(e5)*sin(e6) - 4*de1*m6*x6*y6*cos(e2)*cos(e3)*cos(e4)*cos(e5)^2*cos(e6)*sin(e2)*sin(e3)*sin(e4)*sin(e6),2*I4xy*de2*cos(e4)^2 - I4xy*de3 - I4xy*de2 + 2*I4xy*de3*cos(e4)^2 - (I4xx*de2*sin(2*e4))/2 - (I4xx*de3*sin(2*e4))/2 + (I6xx*de2*sin(2*e4))/2 + (I6xx*de3*sin(2*e4))/2 + (I4yy*de2*sin(2*e4))/2 + (I4yy*de3*sin(2*e4))/2 - (I5yy*de2*sin(2*e4))/2 - (I5yy*de3*sin(2*e4))/2 + (I5zz*de2*sin(2*e4))/2 + (I5zz*de3*sin(2*e4))/2 - (I6zz*de2*sin(2*e4))/2 - (I6zz*de3*sin(2*e4))/2 + I6xy*de2*cos(e5) + I6xy*de3*cos(e5) + I5zx*de2*cos(e5) + I5zx*de3*cos(e5) + (I5xx*de5*sin(e4))/2 + (I6xx*de5*sin(e4))/2 - I5yz*de2*sin(e5) - (I5yy*de5*sin(e4))/2 - I5yz*de3*sin(e5) + (I6yy*de5*sin(e4))/2 + (I5zz*de5*sin(e4))/2 - (I6zz*de5*sin(e4))/2 - I5xx*de5*cos(e5)^2*sin(e4) + 2*I5yz*de2*cos(e4)^2*sin(e5) + 2*I5yz*de3*cos(e4)^2*sin(e5) + I5yy*de5*cos(e5)^2*sin(e4) - I6yy*de5*cos(e5)^2*sin(e4) + I6zz*de5*cos(e5)^2*sin(e4) - de2*m4*x4*y4 - de3*m4*x4*y4 + (de2*m4*x4^2*sin(2*e4))/2 + (de3*m4*x4^2*sin(2*e4))/2 - (de2*m6*x6^2*sin(2*e4))/2 - (de3*m6*x6^2*sin(2*e4))/2 - (de2*m4*y4^2*sin(2*e4))/2 - (de3*m4*y4^2*sin(2*e4))/2 + (de2*m5*y5^2*sin(2*e4))/2 + (de3*m5*y5^2*sin(2*e4))/2 - (de2*m5*z5^2*sin(2*e4))/2 - (de3*m5*z5^2*sin(2*e4))/2 + (de2*m6*z6^2*sin(2*e4))/2 + (de3*m6*z6^2*sin(2*e4))/2 - (I4xx*de1*cos(e2)*cos(e3))/2 - (I5xx*de1*cos(e2)*cos(e3))/2 + (I6xx*de1*cos(e2)*cos(e3))/2 - I6xy*de5*cos(e4)*cos(e5) + (I4yy*de1*cos(e2)*cos(e3))/2 - (I5yy*de1*cos(e2)*cos(e3))/2 - (I6yy*de1*cos(e2)*cos(e3))/2 - (I4zz*de1*cos(e2)*cos(e3))/2 + (I5zz*de1*cos(e2)*cos(e3))/2 - (I6zz*de1*cos(e2)*cos(e3))/2 - I5zx*de5*cos(e4)*cos(e5) + (I6xx*de6*cos(e4)*sin(e5))/2 + I5yz*de5*cos(e4)*sin(e5) + I6yz*de2*cos(e6)*sin(e5) - (I6yy*de6*cos(e4)*sin(e5))/2 + I6yz*de3*cos(e6)*sin(e5) + I6yz*de6*cos(e6)*sin(e4) - (I6zz*de6*cos(e4)*sin(e5))/2 + (I4xx*de1*sin(e2)*sin(e3))/2 + (I5xx*de1*sin(e2)*sin(e3))/2 - (I6xx*de1*sin(e2)*sin(e3))/2 - (I4yy*de1*sin(e2)*sin(e3))/2 + (I5yy*de1*sin(e2)*sin(e3))/2 + (I6yy*de1*sin(e2)*sin(e3))/2 + (I4zz*de1*sin(e2)*sin(e3))/2 - (I5zz*de1*sin(e2)*sin(e3))/2 + (I6zz*de1*sin(e2)*sin(e3))/2 + I6zx*de2*sin(e5)*sin(e6) + I6zx*de3*sin(e5)*sin(e6) + I6zx*de6*sin(e4)*sin(e6) + de5*m5*y5^2*sin(e4) + de5*m6*z6^2*sin(e4) - 2*I6xy*de2*cos(e4)^2*cos(e5) - 2*I6xy*de3*cos(e4)^2*cos(e5) - 2*I6xy*de2*cos(e5)*cos(e6)^2 - 2*I6xy*de3*cos(e5)*cos(e6)^2 - 2*I5zx*de2*cos(e4)^2*cos(e5) - 2*I5zx*de3*cos(e4)^2*cos(e5) + de5*m5*x5^2*cos(e5)^2*sin(e4) - de5*m5*y5^2*cos(e5)^2*sin(e4) + de5*m6*y6^2*cos(e5)^2*sin(e4) - de5*m6*z6^2*cos(e5)^2*sin(e4) + 4*I6xy*de2*cos(e4)^2*cos(e5)*cos(e6)^2 + 4*I6xy*de3*cos(e4)^2*cos(e5)*cos(e6)^2 - I6xx*de5*cos(e5)^2*cos(e6)^2*sin(e4) + I6yy*de5*cos(e5)^2*cos(e6)^2*sin(e4) + 2*de2*m4*x4*y4*cos(e4)^2 + 2*de3*m4*x4*y4*cos(e4)^2 - I5xy*de1*cos(e2)*cos(e4)*sin(e3) - I5xy*de1*cos(e3)*cos(e4)*sin(e2) + I6xx*de2*cos(e5)*cos(e6)*sin(e6) + I6xx*de3*cos(e5)*cos(e6)*sin(e6) - I6yy*de2*cos(e5)*cos(e6)*sin(e6) - I6yy*de3*cos(e5)*cos(e6)*sin(e6) - I6yz*de5*cos(e4)*cos(e6)*sin(e5) + I4zx*de1*cos(e2)*cos(e4)*sin(e3) + I4zx*de1*cos(e3)*cos(e4)*sin(e2) - 2*I5xy*de5*cos(e5)*sin(e4)*sin(e5) + I6xy*de6*cos(e5)*sin(e4)*sin(e5) - I4yz*de1*cos(e2)*sin(e3)*sin(e4) - I4yz*de1*cos(e3)*sin(e2)*sin(e4) - I6zx*de5*cos(e4)*sin(e5)*sin(e6) - de1*m6*x6^2*cos(e2)*cos(e3) - de1*m4*y4^2*cos(e2)*cos(e3) - de1*m5*z5^2*cos(e2)*cos(e3) - de6*m6*x6^2*cos(e4)*sin(e5) + de1*m6*x6^2*sin(e2)*sin(e3) + de1*m4*y4^2*sin(e2)*sin(e3) + de1*m5*z5^2*sin(e2)*sin(e3) + I4xx*de1*cos(e2)*cos(e3)*cos(e4)^2 - I6xx*de1*cos(e2)*cos(e3)*cos(e4)^2 - I6xx*de1*cos(e2)*cos(e3)*cos(e6)^2 + 2*I6xy*de5*cos(e4)*cos(e5)*cos(e6)^2 - I4yy*de1*cos(e2)*cos(e3)*cos(e4)^2 + I5yy*de1*cos(e2)*cos(e3)*cos(e4)^2 + I6yy*de1*cos(e2)*cos(e3)*cos(e6)^2 - I5zz*de1*cos(e2)*cos(e3)*cos(e4)^2 + I6zz*de1*cos(e2)*cos(e3)*cos(e4)^2 + a3*de2*m4*y4*cos(e4) + a3*de3*m4*y4*cos(e4) - a3*de2*m5*z5*cos(e4) - a3*de3*m5*z5*cos(e4) - I5xx*de2*cos(e4)*cos(e5)^2*sin(e4) - I5xx*de3*cos(e4)*cos(e5)^2*sin(e4) - I6xx*de2*cos(e4)*cos(e6)^2*sin(e4) - I6xx*de3*cos(e4)*cos(e6)^2*sin(e4) - I6xx*de6*cos(e4)*cos(e6)^2*sin(e5) + I5yy*de2*cos(e4)*cos(e5)^2*sin(e4) + I5yy*de3*cos(e4)*cos(e5)^2*sin(e4) - I6yy*de2*cos(e4)*cos(e5)^2*sin(e4) + I6yy*de2*cos(e4)*cos(e6)^2*sin(e4) - I6yy*de3*cos(e4)*cos(e5)^2*sin(e4) + I6yy*de3*cos(e4)*cos(e6)^2*sin(e4) - 2*I6yz*de2*cos(e4)^2*cos(e6)*sin(e5) - 2*I6yz*de3*cos(e4)^2*cos(e6)*sin(e5) + I6yy*de6*cos(e4)*cos(e6)^2*sin(e5) - I6yz*de6*cos(e5)^2*cos(e6)*sin(e4) + I6zz*de2*cos(e4)*cos(e5)^2*sin(e4) + I6zz*de3*cos(e4)*cos(e5)^2*sin(e4) + a3*de2*m4*x4*sin(e4) + a3*de3*m4*x4*sin(e4) - I4xx*de1*cos(e4)^2*sin(e2)*sin(e3) + I6xx*de1*cos(e4)^2*sin(e2)*sin(e3) + I6xx*de1*cos(e6)^2*sin(e2)*sin(e3) + I4yy*de1*cos(e4)^2*sin(e2)*sin(e3) - I5yy*de1*cos(e4)^2*sin(e2)*sin(e3) - I6yy*de1*cos(e6)^2*sin(e2)*sin(e3) + I5zz*de1*cos(e4)^2*sin(e2)*sin(e3) - I6zz*de1*cos(e4)^2*sin(e2)*sin(e3) - 2*I6zx*de2*cos(e4)^2*sin(e5)*sin(e6) - 2*I6zx*de3*cos(e4)^2*sin(e5)*sin(e6) - I6zx*de6*cos(e5)^2*sin(e4)*sin(e6) + de2*m6*x6*y6*cos(e5) + de3*m6*x6*y6*cos(e5) + de2*m5*x5*z5*cos(e5) + de3*m5*x5*z5*cos(e5) - de2*m5*y5*z5*sin(e5) - de3*m5*y5*z5*sin(e5) - I5xx*de1*cos(e4)^2*cos(e5)^2*sin(e2)*sin(e3) - I6xx*de1*cos(e4)^2*cos(e6)^2*sin(e2)*sin(e3) + I5yy*de1*cos(e4)^2*cos(e5)^2*sin(e2)*sin(e3) - I6yy*de1*cos(e4)^2*cos(e5)^2*sin(e2)*sin(e3) + I6yy*de1*cos(e4)^2*cos(e6)^2*sin(e2)*sin(e3) + I6zz*de1*cos(e4)^2*cos(e5)^2*sin(e2)*sin(e3) - 2*de2*m6*x6*y6*cos(e4)^2*cos(e5) - 2*de3*m6*x6*y6*cos(e4)^2*cos(e5) - 2*de2*m6*x6*y6*cos(e5)*cos(e6)^2 - 2*de3*m6*x6*y6*cos(e5)*cos(e6)^2 - 2*de2*m5*x5*z5*cos(e4)^2*cos(e5) - 2*de3*m5*x5*z5*cos(e4)^2*cos(e5) + 2*de2*m5*y5*z5*cos(e4)^2*sin(e5) + 2*de3*m5*y5*z5*cos(e4)^2*sin(e5) + de5*m6*x6^2*cos(e5)^2*cos(e6)^2*sin(e4) - de5*m6*y6^2*cos(e5)^2*cos(e6)^2*sin(e4) + 2*I4xy*de1*cos(e2)*cos(e3)*cos(e4)*sin(e4) - 2*I6xy*de1*cos(e2)*cos(e3)*cos(e6)*sin(e6) - I6xx*de5*cos(e4)*cos(e5)*cos(e6)*sin(e6) + I6yy*de5*cos(e4)*cos(e5)*cos(e6)*sin(e6) - I6zx*de1*cos(e2)*cos(e4)*cos(e6)*sin(e3) - I6zx*de1*cos(e3)*cos(e4)*cos(e6)*sin(e2) - 2*I5xy*de2*cos(e4)*cos(e5)*sin(e4)*sin(e5) - 2*I5xy*de3*cos(e4)*cos(e5)*sin(e4)*sin(e5) - 2*I6xy*de2*cos(e4)*cos(e6)*sin(e4)*sin(e6) - 2*I6xy*de3*cos(e4)*cos(e6)*sin(e4)*sin(e6) - 2*I6xy*de6*cos(e4)*cos(e6)*sin(e5)*sin(e6) + I5yz*de1*cos(e2)*cos(e5)*sin(e3)*sin(e4) + I5yz*de1*cos(e3)*cos(e5)*sin(e2)*sin(e4) + I6yz*de1*cos(e2)*cos(e4)*sin(e3)*sin(e6) + I6yz*de1*cos(e3)*cos(e4)*sin(e2)*sin(e6) - 2*I6zx*de5*cos(e5)*cos(e6)*sin(e4)*sin(e5) - 2*I4xy*de1*cos(e4)*sin(e2)*sin(e3)*sin(e4) + I6xy*de1*cos(e2)*sin(e3)*sin(e4)*sin(e5) + I6xy*de1*cos(e3)*sin(e2)*sin(e4)*sin(e5) + 2*I6xy*de1*cos(e6)*sin(e2)*sin(e3)*sin(e6) + 2*I6yz*de5*cos(e5)*sin(e4)*sin(e5)*sin(e6) + I5zx*de1*cos(e2)*sin(e3)*sin(e4)*sin(e5) + I5zx*de1*cos(e3)*sin(e2)*sin(e4)*sin(e5) - de2*m6*x6^2*cos(e5)*cos(e6)*sin(e6) - de3*m6*x6^2*cos(e5)*cos(e6)*sin(e6) + de2*m6*y6^2*cos(e5)*cos(e6)*sin(e6) + de3*m6*y6^2*cos(e5)*cos(e6)*sin(e6) - a2*de1*m4*x4*cos(e2)*cos(e4) + a2*de2*m4*y4*cos(e3)*cos(e4) + a3*de2*m6*y6*cos(e4)*cos(e6) + a3*de3*m6*y6*cos(e4)*cos(e6) - a2*de2*m5*z5*cos(e3)*cos(e4) + 2*I5xy*de1*cos(e2)*cos(e4)*cos(e5)^2*sin(e3) + 2*I5xy*de1*cos(e3)*cos(e4)*cos(e5)^2*sin(e2) - 2*I6xx*de2*cos(e4)^2*cos(e5)*cos(e6)*sin(e6) - 2*I6xx*de3*cos(e4)^2*cos(e5)*cos(e6)*sin(e6) + 2*I6yy*de2*cos(e4)^2*cos(e5)*cos(e6)*sin(e6) + 2*I6yy*de3*cos(e4)^2*cos(e5)*cos(e6)*sin(e6) + a2*de2*m4*x4*cos(e3)*sin(e4) + a3*de2*m5*x5*cos(e5)*sin(e4) + a3*de3*m5*x5*cos(e5)*sin(e4) + a3*de2*m6*x6*cos(e4)*sin(e6) + a3*de3*m6*x6*cos(e4)*sin(e6) + a2*de1*m4*y4*cos(e2)*sin(e4) - a2*de1*m5*z5*cos(e2)*sin(e4) - 2*I6xy*de5*cos(e5)^2*cos(e6)*sin(e4)*sin(e6) - 2*I6xy*de6*cos(e5)*cos(e6)^2*sin(e4)*sin(e5) - de5*m6*x6*y6*cos(e4)*cos(e5) - de5*m5*x5*z5*cos(e4)*cos(e5) - a3*de2*m5*y5*sin(e4)*sin(e5) - a3*de3*m5*y5*sin(e4)*sin(e5) - a3*de2*m6*z6*sin(e4)*sin(e5) - a3*de3*m6*z6*sin(e4)*sin(e5) - de1*m4*x4^2*cos(e2)*cos(e3)*cos(e4)^2 + de1*m6*x6^2*cos(e2)*cos(e3)*cos(e4)^2 + de1*m6*x6^2*cos(e2)*cos(e3)*cos(e6)^2 + de1*m4*y4^2*cos(e2)*cos(e3)*cos(e4)^2 - de1*m5*y5^2*cos(e2)*cos(e3)*cos(e4)^2 - de1*m6*y6^2*cos(e2)*cos(e3)*cos(e6)^2 + de1*m5*z5^2*cos(e2)*cos(e3)*cos(e4)^2 - de1*m6*z6^2*cos(e2)*cos(e3)*cos(e4)^2 + de5*m5*y5*z5*cos(e4)*sin(e5) + de2*m6*y6*z6*cos(e6)*sin(e5) + de3*m6*y6*z6*cos(e6)*sin(e5) + de6*m6*y6*z6*cos(e6)*sin(e4) + de2*m5*x5^2*cos(e4)*cos(e5)^2*sin(e4) + de3*m5*x5^2*cos(e4)*cos(e5)^2*sin(e4) + de2*m6*x6^2*cos(e4)*cos(e6)^2*sin(e4) + de3*m6*x6^2*cos(e4)*cos(e6)^2*sin(e4) + de6*m6*x6^2*cos(e4)*cos(e6)^2*sin(e5) - de2*m5*y5^2*cos(e4)*cos(e5)^2*sin(e4) - de3*m5*y5^2*cos(e4)*cos(e5)^2*sin(e4) + de2*m6*y6^2*cos(e4)*cos(e5)^2*sin(e4) - de2*m6*y6^2*cos(e4)*cos(e6)^2*sin(e4) + de3*m6*y6^2*cos(e4)*cos(e5)^2*sin(e4) - de3*m6*y6^2*cos(e4)*cos(e6)^2*sin(e4) - de6*m6*y6^2*cos(e4)*cos(e6)^2*sin(e5) - de2*m6*z6^2*cos(e4)*cos(e5)^2*sin(e4) - de3*m6*z6^2*cos(e4)*cos(e5)^2*sin(e4) + de2*m6*x6*z6*sin(e5)*sin(e6) + de3*m6*x6*z6*sin(e5)*sin(e6) + de6*m6*x6*z6*sin(e4)*sin(e6) + de1*m4*x4^2*cos(e4)^2*sin(e2)*sin(e3) - de1*m6*x6^2*cos(e4)^2*sin(e2)*sin(e3) - de1*m6*x6^2*cos(e6)^2*sin(e2)*sin(e3) - de1*m4*y4^2*cos(e4)^2*sin(e2)*sin(e3) + de1*m5*y5^2*cos(e4)^2*sin(e2)*sin(e3) + de1*m6*y6^2*cos(e6)^2*sin(e2)*sin(e3) - de1*m5*z5^2*cos(e4)^2*sin(e2)*sin(e3) + de1*m6*z6^2*cos(e4)^2*sin(e2)*sin(e3) + I5xx*de1*cos(e2)*cos(e3)*cos(e4)^2*cos(e5)^2 + I6xx*de1*cos(e2)*cos(e3)*cos(e4)^2*cos(e6)^2 - I5yy*de1*cos(e2)*cos(e3)*cos(e4)^2*cos(e5)^2 + I6yy*de1*cos(e2)*cos(e3)*cos(e4)^2*cos(e5)^2 - I6yy*de1*cos(e2)*cos(e3)*cos(e4)^2*cos(e6)^2 - I6zz*de1*cos(e2)*cos(e3)*cos(e4)^2*cos(e5)^2 - I6xx*de2*cos(e4)*cos(e5)^2*cos(e6)^2*sin(e4) - I6xx*de3*cos(e4)*cos(e5)^2*cos(e6)^2*sin(e4) + I6yy*de2*cos(e4)*cos(e5)^2*cos(e6)^2*sin(e4) + I6yy*de3*cos(e4)*cos(e5)^2*cos(e6)^2*sin(e4) - 2*I6xy*de1*cos(e2)*cos(e3)*cos(e4)*cos(e5)*sin(e4) - 2*I5zx*de1*cos(e2)*cos(e3)*cos(e4)*cos(e5)*sin(e4) + de1*m5*x5^2*cos(e4)^2*cos(e5)^2*sin(e2)*sin(e3) + de1*m6*x6^2*cos(e4)^2*cos(e6)^2*sin(e2)*sin(e3) - de1*m5*y5^2*cos(e4)^2*cos(e5)^2*sin(e2)*sin(e3) + de1*m6*y6^2*cos(e4)^2*cos(e5)^2*sin(e2)*sin(e3) - de1*m6*y6^2*cos(e4)^2*cos(e6)^2*sin(e2)*sin(e3) - de1*m6*z6^2*cos(e4)^2*cos(e5)^2*sin(e2)*sin(e3) + I6xx*de1*cos(e2)*cos(e3)*cos(e4)^2*cos(e5)^2*cos(e6)^2 - I6yy*de1*cos(e2)*cos(e3)*cos(e4)^2*cos(e5)^2*cos(e6)^2 - I5xx*de1*cos(e2)*cos(e4)*cos(e5)*sin(e3)*sin(e5) - I5xx*de1*cos(e3)*cos(e4)*cos(e5)*sin(e2)*sin(e5) + I5yy*de1*cos(e2)*cos(e4)*cos(e5)*sin(e3)*sin(e5) + I5yy*de1*cos(e3)*cos(e4)*cos(e5)*sin(e2)*sin(e5) + 2*I5yz*de1*cos(e2)*cos(e3)*cos(e4)*sin(e4)*sin(e5) - I6yy*de1*cos(e2)*cos(e4)*cos(e5)*sin(e3)*sin(e5) - I6yy*de1*cos(e3)*cos(e4)*cos(e5)*sin(e2)*sin(e5) - I6yz*de1*cos(e2)*cos(e5)*cos(e6)*sin(e3)*sin(e4) - I6yz*de1*cos(e3)*cos(e5)*cos(e6)*sin(e2)*sin(e4) + I6zz*de1*cos(e2)*cos(e4)*cos(e5)*sin(e3)*sin(e5) + I6zz*de1*cos(e3)*cos(e4)*cos(e5)*sin(e2)*sin(e5) - 2*I6zx*de2*cos(e4)*cos(e5)*cos(e6)*sin(e4)*sin(e5) - 2*I6zx*de3*cos(e4)*cos(e5)*cos(e6)*sin(e4)*sin(e5) + 2*I6xy*de1*cos(e4)*cos(e5)*sin(e2)*sin(e3)*sin(e4) + I6xx*de6*cos(e5)*cos(e6)*sin(e4)*sin(e5)*sin(e6) + 2*I6yz*de2*cos(e4)*cos(e5)*sin(e4)*sin(e5)*sin(e6) + 2*I6yz*de3*cos(e4)*cos(e5)*sin(e4)*sin(e5)*sin(e6) - I6yy*de6*cos(e5)*cos(e6)*sin(e4)*sin(e5)*sin(e6) + 2*I5zx*de1*cos(e4)*cos(e5)*sin(e2)*sin(e3)*sin(e4) - I6zx*de1*cos(e2)*cos(e5)*sin(e3)*sin(e4)*sin(e6) - I6zx*de1*cos(e3)*cos(e5)*sin(e2)*sin(e4)*sin(e6) - I6xx*de1*cos(e4)^2*cos(e5)^2*cos(e6)^2*sin(e2)*sin(e3) + I6yy*de1*cos(e4)^2*cos(e5)^2*cos(e6)^2*sin(e2)*sin(e3) - 2*I5yz*de1*cos(e4)*sin(e2)*sin(e3)*sin(e4)*sin(e5) + de5*m6*x6^2*cos(e4)*cos(e5)*cos(e6)*sin(e6) + 4*de2*m6*x6*y6*cos(e4)^2*cos(e5)*cos(e6)^2 + 4*de3*m6*x6*y6*cos(e4)^2*cos(e5)*cos(e6)^2 - de5*m6*y6^2*cos(e4)*cos(e5)*cos(e6)*sin(e6) - a3*de1*m4*x4*cos(e2)*cos(e3)*cos(e4) - a2*de1*m5*x5*cos(e2)*cos(e4)*cos(e5) + a2*de2*m6*y6*cos(e3)*cos(e4)*cos(e6) + 2*I5xy*de1*cos(e2)*cos(e3)*cos(e4)^2*cos(e5)*sin(e5) + 2*I6xy*de1*cos(e2)*cos(e3)*cos(e4)^2*cos(e6)*sin(e6) + 2*I6zx*de1*cos(e2)*cos(e4)*cos(e5)^2*cos(e6)*sin(e3) + 2*I6zx*de1*cos(e3)*cos(e4)*cos(e5)^2*cos(e6)*sin(e2) + a2*de2*m5*x5*cos(e3)*cos(e5)*sin(e4) + a2*de2*m6*x6*cos(e3)*cos(e4)*sin(e6) + a3*de2*m6*x6*cos(e5)*cos(e6)*sin(e4) + a3*de3*m6*x6*cos(e5)*cos(e6)*sin(e4) + a3*de1*m4*y4*cos(e2)*cos(e3)*sin(e4) + a2*de1*m5*y5*cos(e2)*cos(e4)*sin(e5) + a2*de1*m6*y6*cos(e2)*cos(e6)*sin(e4) - a3*de1*m5*z5*cos(e2)*cos(e3)*sin(e4) + a2*de1*m6*z6*cos(e2)*cos(e4)*sin(e5) + d4*de1*m4*x4*cos(e2)*cos(e4)*sin(e3) + d4*de1*m4*x4*cos(e3)*cos(e4)*sin(e2) - 2*I6xy*de2*cos(e4)*cos(e5)^2*cos(e6)*sin(e4)*sin(e6) - 2*I6xy*de3*cos(e4)*cos(e5)^2*cos(e6)*sin(e4)*sin(e6) - 2*I6yz*de1*cos(e2)*cos(e4)*cos(e5)^2*sin(e3)*sin(e6) - 2*I6yz*de1*cos(e3)*cos(e4)*cos(e5)^2*sin(e2)*sin(e6) + a3*de1*m4*x4*cos(e4)*sin(e2)*sin(e3) + a2*de1*m6*x6*cos(e2)*sin(e4)*sin(e6) - a2*de2*m5*y5*cos(e3)*sin(e4)*sin(e5) - a3*de2*m6*y6*cos(e5)*sin(e4)*sin(e6) - a3*de3*m6*y6*cos(e5)*sin(e4)*sin(e6) - a2*de2*m6*z6*cos(e3)*sin(e4)*sin(e5) - 2*I5xy*de1*cos(e4)^2*cos(e5)*sin(e2)*sin(e3)*sin(e5) - 2*I6xy*de1*cos(e2)*cos(e6)^2*sin(e3)*sin(e4)*sin(e5) - 2*I6xy*de1*cos(e3)*cos(e6)^2*sin(e2)*sin(e4)*sin(e5) - 2*I6xy*de1*cos(e4)^2*cos(e6)*sin(e2)*sin(e3)*sin(e6) - d4*de1*m4*y4*cos(e2)*sin(e3)*sin(e4) - d4*de1*m4*y4*cos(e3)*sin(e2)*sin(e4) + d4*de1*m5*z5*cos(e2)*sin(e3)*sin(e4) + d4*de1*m5*z5*cos(e3)*sin(e2)*sin(e4) - de1*m5*x5*y5*cos(e2)*cos(e4)*sin(e3) - de1*m5*x5*y5*cos(e3)*cos(e4)*sin(e2) + de1*m4*x4*z4*cos(e2)*cos(e4)*sin(e3) + de1*m4*x4*z4*cos(e3)*cos(e4)*sin(e2) - de5*m6*y6*z6*cos(e4)*cos(e6)*sin(e5) - a3*de1*m4*y4*sin(e2)*sin(e3)*sin(e4) + a3*de1*m5*z5*sin(e2)*sin(e3)*sin(e4) + 2*de2*m6*x6^2*cos(e4)^2*cos(e5)*cos(e6)*sin(e6) + 2*de3*m6*x6^2*cos(e4)^2*cos(e5)*cos(e6)*sin(e6) - 2*de2*m6*y6^2*cos(e4)^2*cos(e5)*cos(e6)*sin(e6) - 2*de3*m6*y6^2*cos(e4)^2*cos(e5)*cos(e6)*sin(e6) - 2*de5*m5*x5*y5*cos(e5)*sin(e4)*sin(e5) + de6*m6*x6*y6*cos(e5)*sin(e4)*sin(e5) - de5*m6*x6*z6*cos(e4)*sin(e5)*sin(e6) - de1*m4*y4*z4*cos(e2)*sin(e3)*sin(e4) - de1*m4*y4*z4*cos(e3)*sin(e2)*sin(e4) + 2*de5*m6*x6*y6*cos(e4)*cos(e5)*cos(e6)^2 - de1*m5*x5^2*cos(e2)*cos(e3)*cos(e4)^2*cos(e5)^2 - de1*m6*x6^2*cos(e2)*cos(e3)*cos(e4)^2*cos(e6)^2 + de1*m5*y5^2*cos(e2)*cos(e3)*cos(e4)^2*cos(e5)^2 - de1*m6*y6^2*cos(e2)*cos(e3)*cos(e4)^2*cos(e5)^2 + de1*m6*y6^2*cos(e2)*cos(e3)*cos(e4)^2*cos(e6)^2 + de1*m6*z6^2*cos(e2)*cos(e3)*cos(e4)^2*cos(e5)^2 - 2*de2*m6*y6*z6*cos(e4)^2*cos(e6)*sin(e5) - 2*de3*m6*y6*z6*cos(e4)^2*cos(e6)*sin(e5) - de6*m6*y6*z6*cos(e5)^2*cos(e6)*sin(e4) + de2*m6*x6^2*cos(e4)*cos(e5)^2*cos(e6)^2*sin(e4) + de3*m6*x6^2*cos(e4)*cos(e5)^2*cos(e6)^2*sin(e4) - de2*m6*y6^2*cos(e4)*cos(e5)^2*cos(e6)^2*sin(e4) - de3*m6*y6^2*cos(e4)*cos(e5)^2*cos(e6)^2*sin(e4) - 2*de2*m6*x6*z6*cos(e4)^2*sin(e5)*sin(e6) - 2*de3*m6*x6*z6*cos(e4)^2*sin(e5)*sin(e6) - de6*m6*x6*z6*cos(e5)^2*sin(e4)*sin(e6) + 2*I6zx*de1*cos(e4)*sin(e2)*sin(e3)*sin(e4)*sin(e5)*sin(e6) - de1*m6*x6^2*cos(e2)*cos(e3)*cos(e4)^2*cos(e5)^2*cos(e6)^2 + de1*m6*y6^2*cos(e2)*cos(e3)*cos(e4)^2*cos(e5)^2*cos(e6)^2 + de1*m5*x5^2*cos(e2)*cos(e4)*cos(e5)*sin(e3)*sin(e5) + de1*m5*x5^2*cos(e3)*cos(e4)*cos(e5)*sin(e2)*sin(e5) - de1*m5*y5^2*cos(e2)*cos(e4)*cos(e5)*sin(e3)*sin(e5) - de1*m5*y5^2*cos(e3)*cos(e4)*cos(e5)*sin(e2)*sin(e5) + de1*m6*y6^2*cos(e2)*cos(e4)*cos(e5)*sin(e3)*sin(e5) + de1*m6*y6^2*cos(e3)*cos(e4)*cos(e5)*sin(e2)*sin(e5) - de1*m6*z6^2*cos(e2)*cos(e4)*cos(e5)*sin(e3)*sin(e5) - de1*m6*z6^2*cos(e3)*cos(e4)*cos(e5)*sin(e2)*sin(e5) - de6*m6*x6^2*cos(e5)*cos(e6)*sin(e4)*sin(e5)*sin(e6) + de6*m6*y6^2*cos(e5)*cos(e6)*sin(e4)*sin(e5)*sin(e6) - a3*de1*m5*x5*cos(e2)*cos(e3)*cos(e4)*cos(e5) - a2*de1*m6*x6*cos(e2)*cos(e4)*cos(e5)*cos(e6) + 4*I6xy*de1*cos(e2)*cos(e3)*cos(e4)*cos(e5)*cos(e6)^2*sin(e4) + 2*I6zx*de1*cos(e2)*cos(e3)*cos(e4)^2*cos(e5)*cos(e6)*sin(e5) + de1*m6*x6^2*cos(e4)^2*cos(e5)^2*cos(e6)^2*sin(e2)*sin(e3) - de1*m6*y6^2*cos(e4)^2*cos(e5)^2*cos(e6)^2*sin(e2)*sin(e3) + a2*de2*m6*x6*cos(e3)*cos(e5)*cos(e6)*sin(e4) + a3*de1*m5*y5*cos(e2)*cos(e3)*cos(e4)*sin(e5) + a3*de1*m6*y6*cos(e2)*cos(e3)*cos(e6)*sin(e4) + a2*de1*m6*y6*cos(e2)*cos(e4)*cos(e5)*sin(e6) + a3*de1*m6*z6*cos(e2)*cos(e3)*cos(e4)*sin(e5) + d4*de1*m5*x5*cos(e2)*cos(e4)*cos(e5)*sin(e3) + d4*de1*m5*x5*cos(e3)*cos(e4)*cos(e5)*sin(e2) - I6xx*de1*cos(e2)*cos(e4)*cos(e5)*cos(e6)^2*sin(e3)*sin(e5) - I6xx*de1*cos(e3)*cos(e4)*cos(e5)*cos(e6)^2*sin(e2)*sin(e5) + I6yy*de1*cos(e2)*cos(e4)*cos(e5)*cos(e6)^2*sin(e3)*sin(e5) + I6yy*de1*cos(e3)*cos(e4)*cos(e5)*cos(e6)^2*sin(e2)*sin(e5) - 2*I6yz*de1*cos(e2)*cos(e3)*cos(e4)^2*cos(e5)*sin(e5)*sin(e6) + a3*de1*m5*x5*cos(e4)*cos(e5)*sin(e2)*sin(e3) + a3*de1*m6*x6*cos(e2)*cos(e3)*sin(e4)*sin(e6) - a2*de2*m6*y6*cos(e3)*cos(e5)*sin(e4)*sin(e6) - 4*I6xy*de1*cos(e4)*cos(e5)*cos(e6)^2*sin(e2)*sin(e3)*sin(e4) - 2*I6zx*de1*cos(e4)^2*cos(e5)*cos(e6)*sin(e2)*sin(e3)*sin(e5) - d4*de1*m5*y5*cos(e2)*cos(e4)*sin(e3)*sin(e5) - d4*de1*m5*y5*cos(e3)*cos(e4)*sin(e2)*sin(e5) - d4*de1*m6*y6*cos(e2)*cos(e6)*sin(e3)*sin(e4) - d4*de1*m6*y6*cos(e3)*cos(e6)*sin(e2)*sin(e4) - d4*de1*m6*z6*cos(e2)*cos(e4)*sin(e3)*sin(e5) - d4*de1*m6*z6*cos(e3)*cos(e4)*sin(e2)*sin(e5) + 2*de1*m4*x4*y4*cos(e2)*cos(e3)*cos(e4)*sin(e4) - 2*de1*m6*x6*y6*cos(e2)*cos(e3)*cos(e6)*sin(e6) - de1*m6*x6*z6*cos(e2)*cos(e4)*cos(e6)*sin(e3) - de1*m6*x6*z6*cos(e3)*cos(e4)*cos(e6)*sin(e2) - a3*de1*m5*y5*cos(e4)*sin(e2)*sin(e3)*sin(e5) - a3*de1*m6*y6*cos(e6)*sin(e2)*sin(e3)*sin(e4) - a3*de1*m6*z6*cos(e4)*sin(e2)*sin(e3)*sin(e5) - d4*de1*m6*x6*cos(e2)*sin(e3)*sin(e4)*sin(e6) - d4*de1*m6*x6*cos(e3)*sin(e2)*sin(e4)*sin(e6) + 2*I6yz*de1*cos(e4)^2*cos(e5)*sin(e2)*sin(e3)*sin(e5)*sin(e6) - 2*de2*m5*x5*y5*cos(e4)*cos(e5)*sin(e4)*sin(e5) - 2*de3*m5*x5*y5*cos(e4)*cos(e5)*sin(e4)*sin(e5) - 2*de2*m6*x6*y6*cos(e4)*cos(e6)*sin(e4)*sin(e6) - 2*de3*m6*x6*y6*cos(e4)*cos(e6)*sin(e4)*sin(e6) - 2*de6*m6*x6*y6*cos(e4)*cos(e6)*sin(e5)*sin(e6) - 2*de5*m6*x6*z6*cos(e5)*cos(e6)*sin(e4)*sin(e5) + de1*m5*y5*z5*cos(e2)*cos(e5)*sin(e3)*sin(e4) + de1*m5*y5*z5*cos(e3)*cos(e5)*sin(e2)*sin(e4) + de1*m6*y6*z6*cos(e2)*cos(e4)*sin(e3)*sin(e6) + de1*m6*y6*z6*cos(e3)*cos(e4)*sin(e2)*sin(e6) - a3*de1*m6*x6*sin(e2)*sin(e3)*sin(e4)*sin(e6) - 2*de1*m4*x4*y4*cos(e4)*sin(e2)*sin(e3)*sin(e4) + de1*m6*x6*y6*cos(e2)*sin(e3)*sin(e4)*sin(e5) + de1*m6*x6*y6*cos(e3)*sin(e2)*sin(e4)*sin(e5) + 2*de1*m6*x6*y6*cos(e6)*sin(e2)*sin(e3)*sin(e6) + de1*m5*x5*z5*cos(e2)*sin(e3)*sin(e4)*sin(e5) + de1*m5*x5*z5*cos(e3)*sin(e2)*sin(e4)*sin(e5) + 2*de5*m6*y6*z6*cos(e5)*sin(e4)*sin(e5)*sin(e6) + 2*I6xy*de1*cos(e2)*cos(e3)*cos(e4)^2*cos(e5)^2*cos(e6)*sin(e6) - 2*I6xy*de1*cos(e4)^2*cos(e5)^2*cos(e6)*sin(e2)*sin(e3)*sin(e6) + 2*de1*m5*x5*y5*cos(e2)*cos(e4)*cos(e5)^2*sin(e3) + 2*de1*m5*x5*y5*cos(e3)*cos(e4)*cos(e5)^2*sin(e2) - 2*de5*m6*x6*y6*cos(e5)^2*cos(e6)*sin(e4)*sin(e6) - 2*de6*m6*x6*y6*cos(e5)*cos(e6)^2*sin(e4)*sin(e5) - 2*I6yz*de1*cos(e2)*cos(e3)*cos(e4)*cos(e6)*sin(e4)*sin(e5) - 2*I6zx*de1*cos(e2)*cos(e3)*cos(e4)*sin(e4)*sin(e5)*sin(e6) + I6xx*de1*cos(e2)*cos(e6)*sin(e3)*sin(e4)*sin(e5)*sin(e6) + I6xx*de1*cos(e3)*cos(e6)*sin(e2)*sin(e4)*sin(e5)*sin(e6) + 2*I6yz*de1*cos(e4)*cos(e6)*sin(e2)*sin(e3)*sin(e4)*sin(e5) - I6yy*de1*cos(e2)*cos(e6)*sin(e3)*sin(e4)*sin(e5)*sin(e6) - I6yy*de1*cos(e3)*cos(e6)*sin(e2)*sin(e4)*sin(e5)*sin(e6) + a3*de1*m6*y6*cos(e2)*cos(e3)*cos(e4)*cos(e5)*sin(e6) + d4*de1*m6*x6*cos(e2)*cos(e4)*cos(e5)*cos(e6)*sin(e3) + d4*de1*m6*x6*cos(e3)*cos(e4)*cos(e5)*cos(e6)*sin(e2) + a3*de1*m6*x6*cos(e4)*cos(e5)*cos(e6)*sin(e2)*sin(e3) - d4*de1*m6*y6*cos(e2)*cos(e4)*cos(e5)*sin(e3)*sin(e6) - d4*de1*m6*y6*cos(e3)*cos(e4)*cos(e5)*sin(e2)*sin(e6) - 2*de1*m6*x6*y6*cos(e2)*cos(e3)*cos(e4)*cos(e5)*sin(e4) - 2*de1*m5*x5*z5*cos(e2)*cos(e3)*cos(e4)*cos(e5)*sin(e4) - a3*de1*m6*y6*cos(e4)*cos(e5)*sin(e2)*sin(e3)*sin(e6) - 2*de2*m6*x6*z6*cos(e4)*cos(e5)*cos(e6)*sin(e4)*sin(e5) - 2*de3*m6*x6*z6*cos(e4)*cos(e5)*cos(e6)*sin(e4)*sin(e5) + 2*de1*m5*y5*z5*cos(e2)*cos(e3)*cos(e4)*sin(e4)*sin(e5) - de1*m6*y6*z6*cos(e2)*cos(e5)*cos(e6)*sin(e3)*sin(e4) - de1*m6*y6*z6*cos(e3)*cos(e5)*cos(e6)*sin(e2)*sin(e4) + de1*m6*x6^2*cos(e2)*cos(e4)*cos(e5)*cos(e6)^2*sin(e3)*sin(e5) + de1*m6*x6^2*cos(e3)*cos(e4)*cos(e5)*cos(e6)^2*sin(e2)*sin(e5) - de1*m6*y6^2*cos(e2)*cos(e4)*cos(e5)*cos(e6)^2*sin(e3)*sin(e5) - de1*m6*y6^2*cos(e3)*cos(e4)*cos(e5)*cos(e6)^2*sin(e2)*sin(e5) + 2*de1*m6*x6*y6*cos(e4)*cos(e5)*sin(e2)*sin(e3)*sin(e4) + 2*de1*m5*x5*z5*cos(e4)*cos(e5)*sin(e2)*sin(e3)*sin(e4) - de1*m6*x6*z6*cos(e2)*cos(e5)*sin(e3)*sin(e4)*sin(e6) - de1*m6*x6*z6*cos(e3)*cos(e5)*sin(e2)*sin(e4)*sin(e6) + 2*de2*m6*y6*z6*cos(e4)*cos(e5)*sin(e4)*sin(e5)*sin(e6) + 2*de3*m6*y6*z6*cos(e4)*cos(e5)*sin(e4)*sin(e5)*sin(e6) - 2*de1*m5*y5*z5*cos(e4)*sin(e2)*sin(e3)*sin(e4)*sin(e5) + 2*de1*m5*x5*y5*cos(e2)*cos(e3)*cos(e4)^2*cos(e5)*sin(e5) + 2*de1*m6*x6*y6*cos(e2)*cos(e3)*cos(e4)^2*cos(e6)*sin(e6) + 2*de1*m6*x6*z6*cos(e2)*cos(e4)*cos(e5)^2*cos(e6)*sin(e3) + 2*de1*m6*x6*z6*cos(e3)*cos(e4)*cos(e5)^2*cos(e6)*sin(e2) - 2*de2*m6*x6*y6*cos(e4)*cos(e5)^2*cos(e6)*sin(e4)*sin(e6) - 2*de3*m6*x6*y6*cos(e4)*cos(e5)^2*cos(e6)*sin(e4)*sin(e6) - 2*de1*m6*y6*z6*cos(e2)*cos(e4)*cos(e5)^2*sin(e3)*sin(e6) - 2*de1*m6*y6*z6*cos(e3)*cos(e4)*cos(e5)^2*sin(e2)*sin(e6) - 2*de1*m5*x5*y5*cos(e4)^2*cos(e5)*sin(e2)*sin(e3)*sin(e5) - 2*de1*m6*x6*y6*cos(e2)*cos(e6)^2*sin(e3)*sin(e4)*sin(e5) - 2*de1*m6*x6*y6*cos(e3)*cos(e6)^2*sin(e2)*sin(e4)*sin(e5) - 2*de1*m6*x6*y6*cos(e4)^2*cos(e6)*sin(e2)*sin(e3)*sin(e6) - 2*I6xx*de1*cos(e2)*cos(e3)*cos(e4)*cos(e5)*cos(e6)*sin(e4)*sin(e6) + 2*I6yy*de1*cos(e2)*cos(e3)*cos(e4)*cos(e5)*cos(e6)*sin(e4)*sin(e6) - 2*I6xy*de1*cos(e2)*cos(e4)*cos(e5)*cos(e6)*sin(e3)*sin(e5)*sin(e6) - 2*I6xy*de1*cos(e3)*cos(e4)*cos(e5)*cos(e6)*sin(e2)*sin(e5)*sin(e6) + 2*I6xx*de1*cos(e4)*cos(e5)*cos(e6)*sin(e2)*sin(e3)*sin(e4)*sin(e6) - 2*I6yy*de1*cos(e4)*cos(e5)*cos(e6)*sin(e2)*sin(e3)*sin(e4)*sin(e6) - a3*de1*m6*x6*cos(e2)*cos(e3)*cos(e4)*cos(e5)*cos(e6) - de1*m6*x6^2*cos(e2)*cos(e6)*sin(e3)*sin(e4)*sin(e5)*sin(e6) - de1*m6*x6^2*cos(e3)*cos(e6)*sin(e2)*sin(e4)*sin(e5)*sin(e6) + de1*m6*y6^2*cos(e2)*cos(e6)*sin(e3)*sin(e4)*sin(e5)*sin(e6) + de1*m6*y6^2*cos(e3)*cos(e6)*sin(e2)*sin(e4)*sin(e5)*sin(e6) - 2*de1*m6*x6*z6*cos(e2)*cos(e3)*cos(e4)*sin(e4)*sin(e5)*sin(e6) + 2*de1*m6*y6*z6*cos(e4)*cos(e6)*sin(e2)*sin(e3)*sin(e4)*sin(e5) + 2*de1*m6*x6*z6*cos(e4)*sin(e2)*sin(e3)*sin(e4)*sin(e5)*sin(e6) + 4*de1*m6*x6*y6*cos(e2)*cos(e3)*cos(e4)*cos(e5)*cos(e6)^2*sin(e4) + 2*de1*m6*x6*z6*cos(e2)*cos(e3)*cos(e4)^2*cos(e5)*cos(e6)*sin(e5) - 2*de1*m6*y6*z6*cos(e2)*cos(e3)*cos(e4)^2*cos(e5)*sin(e5)*sin(e6) - 4*de1*m6*x6*y6*cos(e4)*cos(e5)*cos(e6)^2*sin(e2)*sin(e3)*sin(e4) - 2*de1*m6*x6*z6*cos(e4)^2*cos(e5)*cos(e6)*sin(e2)*sin(e3)*sin(e5) + 2*de1*m6*y6*z6*cos(e4)^2*cos(e5)*sin(e2)*sin(e3)*sin(e5)*sin(e6) + 2*de1*m6*x6^2*cos(e2)*cos(e3)*cos(e4)*cos(e5)*cos(e6)*sin(e4)*sin(e6) + 2*de1*m6*x6*y6*cos(e2)*cos(e3)*cos(e4)^2*cos(e5)^2*cos(e6)*sin(e6) - 2*de1*m6*y6^2*cos(e2)*cos(e3)*cos(e4)*cos(e5)*cos(e6)*sin(e4)*sin(e6) - 2*de1*m6*x6^2*cos(e4)*cos(e5)*cos(e6)*sin(e2)*sin(e3)*sin(e4)*sin(e6) - 2*de1*m6*x6*y6*cos(e4)^2*cos(e5)^2*cos(e6)*sin(e2)*sin(e3)*sin(e6) + 2*de1*m6*y6^2*cos(e4)*cos(e5)*cos(e6)*sin(e2)*sin(e3)*sin(e4)*sin(e6) - 2*de1*m6*y6*z6*cos(e2)*cos(e3)*cos(e4)*cos(e6)*sin(e4)*sin(e5) - 2*de1*m6*x6*y6*cos(e2)*cos(e4)*cos(e5)*cos(e6)*sin(e3)*sin(e5)*sin(e6) - 2*de1*m6*x6*y6*cos(e3)*cos(e4)*cos(e5)*cos(e6)*sin(e2)*sin(e5)*sin(e6),2*I4xy*de2*cos(e4)^2 - I4xy*de3 - I4xy*de2 + 2*I4xy*de3*cos(e4)^2 - (I4xx*de2*sin(2*e4))/2 - (I4xx*de3*sin(2*e4))/2 + (I6xx*de2*sin(2*e4))/2 + (I6xx*de3*sin(2*e4))/2 + (I4yy*de2*sin(2*e4))/2 + (I4yy*de3*sin(2*e4))/2 - (I5yy*de2*sin(2*e4))/2 - (I5yy*de3*sin(2*e4))/2 + (I5zz*de2*sin(2*e4))/2 + (I5zz*de3*sin(2*e4))/2 - (I6zz*de2*sin(2*e4))/2 - (I6zz*de3*sin(2*e4))/2 + I6xy*de2*cos(e5) + I6xy*de3*cos(e5) + I5zx*de2*cos(e5) + I5zx*de3*cos(e5) + (I5xx*de5*sin(e4))/2 + (I6xx*de5*sin(e4))/2 - I5yz*de2*sin(e5) - (I5yy*de5*sin(e4))/2 - I5yz*de3*sin(e5) + (I6yy*de5*sin(e4))/2 + (I5zz*de5*sin(e4))/2 - (I6zz*de5*sin(e4))/2 - I5xx*de5*cos(e5)^2*sin(e4) + 2*I5yz*de2*cos(e4)^2*sin(e5) + 2*I5yz*de3*cos(e4)^2*sin(e5) + I5yy*de5*cos(e5)^2*sin(e4) - I6yy*de5*cos(e5)^2*sin(e4) + I6zz*de5*cos(e5)^2*sin(e4) - de2*m4*x4*y4 - de3*m4*x4*y4 + (de2*m4*x4^2*sin(2*e4))/2 + (de3*m4*x4^2*sin(2*e4))/2 - (de2*m6*x6^2*sin(2*e4))/2 - (de3*m6*x6^2*sin(2*e4))/2 - (de2*m4*y4^2*sin(2*e4))/2 - (de3*m4*y4^2*sin(2*e4))/2 + (de2*m5*y5^2*sin(2*e4))/2 + (de3*m5*y5^2*sin(2*e4))/2 - (de2*m5*z5^2*sin(2*e4))/2 - (de3*m5*z5^2*sin(2*e4))/2 + (de2*m6*z6^2*sin(2*e4))/2 + (de3*m6*z6^2*sin(2*e4))/2 - (I4xx*de1*cos(e2)*cos(e3))/2 - (I5xx*de1*cos(e2)*cos(e3))/2 + (I6xx*de1*cos(e2)*cos(e3))/2 - I6xy*de5*cos(e4)*cos(e5) + (I4yy*de1*cos(e2)*cos(e3))/2 - (I5yy*de1*cos(e2)*cos(e3))/2 - (I6yy*de1*cos(e2)*cos(e3))/2 - (I4zz*de1*cos(e2)*cos(e3))/2 + (I5zz*de1*cos(e2)*cos(e3))/2 - (I6zz*de1*cos(e2)*cos(e3))/2 - I5zx*de5*cos(e4)*cos(e5) + (I6xx*de6*cos(e4)*sin(e5))/2 + I5yz*de5*cos(e4)*sin(e5) + I6yz*de2*cos(e6)*sin(e5) - (I6yy*de6*cos(e4)*sin(e5))/2 + I6yz*de3*cos(e6)*sin(e5) + I6yz*de6*cos(e6)*sin(e4) - (I6zz*de6*cos(e4)*sin(e5))/2 + (I4xx*de1*sin(e2)*sin(e3))/2 + (I5xx*de1*sin(e2)*sin(e3))/2 - (I6xx*de1*sin(e2)*sin(e3))/2 - (I4yy*de1*sin(e2)*sin(e3))/2 + (I5yy*de1*sin(e2)*sin(e3))/2 + (I6yy*de1*sin(e2)*sin(e3))/2 + (I4zz*de1*sin(e2)*sin(e3))/2 - (I5zz*de1*sin(e2)*sin(e3))/2 + (I6zz*de1*sin(e2)*sin(e3))/2 + I6zx*de2*sin(e5)*sin(e6) + I6zx*de3*sin(e5)*sin(e6) + I6zx*de6*sin(e4)*sin(e6) + de5*m5*y5^2*sin(e4) + de5*m6*z6^2*sin(e4) - 2*I6xy*de2*cos(e4)^2*cos(e5) - 2*I6xy*de3*cos(e4)^2*cos(e5) - 2*I6xy*de2*cos(e5)*cos(e6)^2 - 2*I6xy*de3*cos(e5)*cos(e6)^2 - 2*I5zx*de2*cos(e4)^2*cos(e5) - 2*I5zx*de3*cos(e4)^2*cos(e5) + de5*m5*x5^2*cos(e5)^2*sin(e4) - de5*m5*y5^2*cos(e5)^2*sin(e4) + de5*m6*y6^2*cos(e5)^2*sin(e4) - de5*m6*z6^2*cos(e5)^2*sin(e4) + 4*I6xy*de2*cos(e4)^2*cos(e5)*cos(e6)^2 + 4*I6xy*de3*cos(e4)^2*cos(e5)*cos(e6)^2 - I6xx*de5*cos(e5)^2*cos(e6)^2*sin(e4) + I6yy*de5*cos(e5)^2*cos(e6)^2*sin(e4) + 2*de2*m4*x4*y4*cos(e4)^2 + 2*de3*m4*x4*y4*cos(e4)^2 - I5xy*de1*cos(e2)*cos(e4)*sin(e3) - I5xy*de1*cos(e3)*cos(e4)*sin(e2) + I6xx*de2*cos(e5)*cos(e6)*sin(e6) + I6xx*de3*cos(e5)*cos(e6)*sin(e6) - I6yy*de2*cos(e5)*cos(e6)*sin(e6) - I6yy*de3*cos(e5)*cos(e6)*sin(e6) - I6yz*de5*cos(e4)*cos(e6)*sin(e5) + I4zx*de1*cos(e2)*cos(e4)*sin(e3) + I4zx*de1*cos(e3)*cos(e4)*sin(e2) - 2*I5xy*de5*cos(e5)*sin(e4)*sin(e5) + I6xy*de6*cos(e5)*sin(e4)*sin(e5) - I4yz*de1*cos(e2)*sin(e3)*sin(e4) - I4yz*de1*cos(e3)*sin(e2)*sin(e4) - I6zx*de5*cos(e4)*sin(e5)*sin(e6) - de1*m6*x6^2*cos(e2)*cos(e3) - de1*m4*y4^2*cos(e2)*cos(e3) - de1*m5*z5^2*cos(e2)*cos(e3) - de6*m6*x6^2*cos(e4)*sin(e5) + de1*m6*x6^2*sin(e2)*sin(e3) + de1*m4*y4^2*sin(e2)*sin(e3) + de1*m5*z5^2*sin(e2)*sin(e3) + I4xx*de1*cos(e2)*cos(e3)*cos(e4)^2 - I6xx*de1*cos(e2)*cos(e3)*cos(e4)^2 - I6xx*de1*cos(e2)*cos(e3)*cos(e6)^2 + 2*I6xy*de5*cos(e4)*cos(e5)*cos(e6)^2 - I4yy*de1*cos(e2)*cos(e3)*cos(e4)^2 + I5yy*de1*cos(e2)*cos(e3)*cos(e4)^2 + I6yy*de1*cos(e2)*cos(e3)*cos(e6)^2 - I5zz*de1*cos(e2)*cos(e3)*cos(e4)^2 + I6zz*de1*cos(e2)*cos(e3)*cos(e4)^2 + a3*de2*m4*y4*cos(e4) + a3*de3*m4*y4*cos(e4) - a3*de2*m5*z5*cos(e4) - a3*de3*m5*z5*cos(e4) - I5xx*de2*cos(e4)*cos(e5)^2*sin(e4) - I5xx*de3*cos(e4)*cos(e5)^2*sin(e4) - I6xx*de2*cos(e4)*cos(e6)^2*sin(e4) - I6xx*de3*cos(e4)*cos(e6)^2*sin(e4) - I6xx*de6*cos(e4)*cos(e6)^2*sin(e5) + I5yy*de2*cos(e4)*cos(e5)^2*sin(e4) + I5yy*de3*cos(e4)*cos(e5)^2*sin(e4) - I6yy*de2*cos(e4)*cos(e5)^2*sin(e4) + I6yy*de2*cos(e4)*cos(e6)^2*sin(e4) - I6yy*de3*cos(e4)*cos(e5)^2*sin(e4) + I6yy*de3*cos(e4)*cos(e6)^2*sin(e4) - 2*I6yz*de2*cos(e4)^2*cos(e6)*sin(e5) - 2*I6yz*de3*cos(e4)^2*cos(e6)*sin(e5) + I6yy*de6*cos(e4)*cos(e6)^2*sin(e5) - I6yz*de6*cos(e5)^2*cos(e6)*sin(e4) + I6zz*de2*cos(e4)*cos(e5)^2*sin(e4) + I6zz*de3*cos(e4)*cos(e5)^2*sin(e4) + a3*de2*m4*x4*sin(e4) + a3*de3*m4*x4*sin(e4) - I4xx*de1*cos(e4)^2*sin(e2)*sin(e3) + I6xx*de1*cos(e4)^2*sin(e2)*sin(e3) + I6xx*de1*cos(e6)^2*sin(e2)*sin(e3) + I4yy*de1*cos(e4)^2*sin(e2)*sin(e3) - I5yy*de1*cos(e4)^2*sin(e2)*sin(e3) - I6yy*de1*cos(e6)^2*sin(e2)*sin(e3) + I5zz*de1*cos(e4)^2*sin(e2)*sin(e3) - I6zz*de1*cos(e4)^2*sin(e2)*sin(e3) - 2*I6zx*de2*cos(e4)^2*sin(e5)*sin(e6) - 2*I6zx*de3*cos(e4)^2*sin(e5)*sin(e6) - I6zx*de6*cos(e5)^2*sin(e4)*sin(e6) + de2*m6*x6*y6*cos(e5) + de3*m6*x6*y6*cos(e5) + de2*m5*x5*z5*cos(e5) + de3*m5*x5*z5*cos(e5) - de2*m5*y5*z5*sin(e5) - de3*m5*y5*z5*sin(e5) - I5xx*de1*cos(e4)^2*cos(e5)^2*sin(e2)*sin(e3) - I6xx*de1*cos(e4)^2*cos(e6)^2*sin(e2)*sin(e3) + I5yy*de1*cos(e4)^2*cos(e5)^2*sin(e2)*sin(e3) - I6yy*de1*cos(e4)^2*cos(e5)^2*sin(e2)*sin(e3) + I6yy*de1*cos(e4)^2*cos(e6)^2*sin(e2)*sin(e3) + I6zz*de1*cos(e4)^2*cos(e5)^2*sin(e2)*sin(e3) - 2*de2*m6*x6*y6*cos(e4)^2*cos(e5) - 2*de3*m6*x6*y6*cos(e4)^2*cos(e5) - 2*de2*m6*x6*y6*cos(e5)*cos(e6)^2 - 2*de3*m6*x6*y6*cos(e5)*cos(e6)^2 - 2*de2*m5*x5*z5*cos(e4)^2*cos(e5) - 2*de3*m5*x5*z5*cos(e4)^2*cos(e5) + 2*de2*m5*y5*z5*cos(e4)^2*sin(e5) + 2*de3*m5*y5*z5*cos(e4)^2*sin(e5) + de5*m6*x6^2*cos(e5)^2*cos(e6)^2*sin(e4) - de5*m6*y6^2*cos(e5)^2*cos(e6)^2*sin(e4) + 2*I4xy*de1*cos(e2)*cos(e3)*cos(e4)*sin(e4) - 2*I6xy*de1*cos(e2)*cos(e3)*cos(e6)*sin(e6) - I6xx*de5*cos(e4)*cos(e5)*cos(e6)*sin(e6) + I6yy*de5*cos(e4)*cos(e5)*cos(e6)*sin(e6) - I6zx*de1*cos(e2)*cos(e4)*cos(e6)*sin(e3) - I6zx*de1*cos(e3)*cos(e4)*cos(e6)*sin(e2) - 2*I5xy*de2*cos(e4)*cos(e5)*sin(e4)*sin(e5) - 2*I5xy*de3*cos(e4)*cos(e5)*sin(e4)*sin(e5) - 2*I6xy*de2*cos(e4)*cos(e6)*sin(e4)*sin(e6) - 2*I6xy*de3*cos(e4)*cos(e6)*sin(e4)*sin(e6) - 2*I6xy*de6*cos(e4)*cos(e6)*sin(e5)*sin(e6) + I5yz*de1*cos(e2)*cos(e5)*sin(e3)*sin(e4) + I5yz*de1*cos(e3)*cos(e5)*sin(e2)*sin(e4) + I6yz*de1*cos(e2)*cos(e4)*sin(e3)*sin(e6) + I6yz*de1*cos(e3)*cos(e4)*sin(e2)*sin(e6) - 2*I6zx*de5*cos(e5)*cos(e6)*sin(e4)*sin(e5) - 2*I4xy*de1*cos(e4)*sin(e2)*sin(e3)*sin(e4) + I6xy*de1*cos(e2)*sin(e3)*sin(e4)*sin(e5) + I6xy*de1*cos(e3)*sin(e2)*sin(e4)*sin(e5) + 2*I6xy*de1*cos(e6)*sin(e2)*sin(e3)*sin(e6) + 2*I6yz*de5*cos(e5)*sin(e4)*sin(e5)*sin(e6) + I5zx*de1*cos(e2)*sin(e3)*sin(e4)*sin(e5) + I5zx*de1*cos(e3)*sin(e2)*sin(e4)*sin(e5) - de2*m6*x6^2*cos(e5)*cos(e6)*sin(e6) - de3*m6*x6^2*cos(e5)*cos(e6)*sin(e6) + de2*m6*y6^2*cos(e5)*cos(e6)*sin(e6) + de3*m6*y6^2*cos(e5)*cos(e6)*sin(e6) + a3*de2*m6*y6*cos(e4)*cos(e6) + a3*de3*m6*y6*cos(e4)*cos(e6) + 2*I5xy*de1*cos(e2)*cos(e4)*cos(e5)^2*sin(e3) + 2*I5xy*de1*cos(e3)*cos(e4)*cos(e5)^2*sin(e2) - 2*I6xx*de2*cos(e4)^2*cos(e5)*cos(e6)*sin(e6) - 2*I6xx*de3*cos(e4)^2*cos(e5)*cos(e6)*sin(e6) + 2*I6yy*de2*cos(e4)^2*cos(e5)*cos(e6)*sin(e6) + 2*I6yy*de3*cos(e4)^2*cos(e5)*cos(e6)*sin(e6) + a3*de2*m5*x5*cos(e5)*sin(e4) + a3*de3*m5*x5*cos(e5)*sin(e4) + a3*de2*m6*x6*cos(e4)*sin(e6) + a3*de3*m6*x6*cos(e4)*sin(e6) - 2*I6xy*de5*cos(e5)^2*cos(e6)*sin(e4)*sin(e6) - 2*I6xy*de6*cos(e5)*cos(e6)^2*sin(e4)*sin(e5) - de5*m6*x6*y6*cos(e4)*cos(e5) - de5*m5*x5*z5*cos(e4)*cos(e5) - a3*de2*m5*y5*sin(e4)*sin(e5) - a3*de3*m5*y5*sin(e4)*sin(e5) - a3*de2*m6*z6*sin(e4)*sin(e5) - a3*de3*m6*z6*sin(e4)*sin(e5) - de1*m4*x4^2*cos(e2)*cos(e3)*cos(e4)^2 + de1*m6*x6^2*cos(e2)*cos(e3)*cos(e4)^2 + de1*m6*x6^2*cos(e2)*cos(e3)*cos(e6)^2 + de1*m4*y4^2*cos(e2)*cos(e3)*cos(e4)^2 - de1*m5*y5^2*cos(e2)*cos(e3)*cos(e4)^2 - de1*m6*y6^2*cos(e2)*cos(e3)*cos(e6)^2 + de1*m5*z5^2*cos(e2)*cos(e3)*cos(e4)^2 - de1*m6*z6^2*cos(e2)*cos(e3)*cos(e4)^2 + de5*m5*y5*z5*cos(e4)*sin(e5) + de2*m6*y6*z6*cos(e6)*sin(e5) + de3*m6*y6*z6*cos(e6)*sin(e5) + de6*m6*y6*z6*cos(e6)*sin(e4) + de2*m5*x5^2*cos(e4)*cos(e5)^2*sin(e4) + de3*m5*x5^2*cos(e4)*cos(e5)^2*sin(e4) + de2*m6*x6^2*cos(e4)*cos(e6)^2*sin(e4) + de3*m6*x6^2*cos(e4)*cos(e6)^2*sin(e4) + de6*m6*x6^2*cos(e4)*cos(e6)^2*sin(e5) - de2*m5*y5^2*cos(e4)*cos(e5)^2*sin(e4) - de3*m5*y5^2*cos(e4)*cos(e5)^2*sin(e4) + de2*m6*y6^2*cos(e4)*cos(e5)^2*sin(e4) - de2*m6*y6^2*cos(e4)*cos(e6)^2*sin(e4) + de3*m6*y6^2*cos(e4)*cos(e5)^2*sin(e4) - de3*m6*y6^2*cos(e4)*cos(e6)^2*sin(e4) - de6*m6*y6^2*cos(e4)*cos(e6)^2*sin(e5) - de2*m6*z6^2*cos(e4)*cos(e5)^2*sin(e4) - de3*m6*z6^2*cos(e4)*cos(e5)^2*sin(e4) + de2*m6*x6*z6*sin(e5)*sin(e6) + de3*m6*x6*z6*sin(e5)*sin(e6) + de6*m6*x6*z6*sin(e4)*sin(e6) + de1*m4*x4^2*cos(e4)^2*sin(e2)*sin(e3) - de1*m6*x6^2*cos(e4)^2*sin(e2)*sin(e3) - de1*m6*x6^2*cos(e6)^2*sin(e2)*sin(e3) - de1*m4*y4^2*cos(e4)^2*sin(e2)*sin(e3) + de1*m5*y5^2*cos(e4)^2*sin(e2)*sin(e3) + de1*m6*y6^2*cos(e6)^2*sin(e2)*sin(e3) - de1*m5*z5^2*cos(e4)^2*sin(e2)*sin(e3) + de1*m6*z6^2*cos(e4)^2*sin(e2)*sin(e3) + I5xx*de1*cos(e2)*cos(e3)*cos(e4)^2*cos(e5)^2 + I6xx*de1*cos(e2)*cos(e3)*cos(e4)^2*cos(e6)^2 - I5yy*de1*cos(e2)*cos(e3)*cos(e4)^2*cos(e5)^2 + I6yy*de1*cos(e2)*cos(e3)*cos(e4)^2*cos(e5)^2 - I6yy*de1*cos(e2)*cos(e3)*cos(e4)^2*cos(e6)^2 - I6zz*de1*cos(e2)*cos(e3)*cos(e4)^2*cos(e5)^2 - I6xx*de2*cos(e4)*cos(e5)^2*cos(e6)^2*sin(e4) - I6xx*de3*cos(e4)*cos(e5)^2*cos(e6)^2*sin(e4) + I6yy*de2*cos(e4)*cos(e5)^2*cos(e6)^2*sin(e4) + I6yy*de3*cos(e4)*cos(e5)^2*cos(e6)^2*sin(e4) - 2*I6xy*de1*cos(e2)*cos(e3)*cos(e4)*cos(e5)*sin(e4) - 2*I5zx*de1*cos(e2)*cos(e3)*cos(e4)*cos(e5)*sin(e4) + de1*m5*x5^2*cos(e4)^2*cos(e5)^2*sin(e2)*sin(e3) + de1*m6*x6^2*cos(e4)^2*cos(e6)^2*sin(e2)*sin(e3) - de1*m5*y5^2*cos(e4)^2*cos(e5)^2*sin(e2)*sin(e3) + de1*m6*y6^2*cos(e4)^2*cos(e5)^2*sin(e2)*sin(e3) - de1*m6*y6^2*cos(e4)^2*cos(e6)^2*sin(e2)*sin(e3) - de1*m6*z6^2*cos(e4)^2*cos(e5)^2*sin(e2)*sin(e3) + I6xx*de1*cos(e2)*cos(e3)*cos(e4)^2*cos(e5)^2*cos(e6)^2 - I6yy*de1*cos(e2)*cos(e3)*cos(e4)^2*cos(e5)^2*cos(e6)^2 - I5xx*de1*cos(e2)*cos(e4)*cos(e5)*sin(e3)*sin(e5) - I5xx*de1*cos(e3)*cos(e4)*cos(e5)*sin(e2)*sin(e5) + I5yy*de1*cos(e2)*cos(e4)*cos(e5)*sin(e3)*sin(e5) + I5yy*de1*cos(e3)*cos(e4)*cos(e5)*sin(e2)*sin(e5) + 2*I5yz*de1*cos(e2)*cos(e3)*cos(e4)*sin(e4)*sin(e5) - I6yy*de1*cos(e2)*cos(e4)*cos(e5)*sin(e3)*sin(e5) - I6yy*de1*cos(e3)*cos(e4)*cos(e5)*sin(e2)*sin(e5) - I6yz*de1*cos(e2)*cos(e5)*cos(e6)*sin(e3)*sin(e4) - I6yz*de1*cos(e3)*cos(e5)*cos(e6)*sin(e2)*sin(e4) + I6zz*de1*cos(e2)*cos(e4)*cos(e5)*sin(e3)*sin(e5) + I6zz*de1*cos(e3)*cos(e4)*cos(e5)*sin(e2)*sin(e5) - 2*I6zx*de2*cos(e4)*cos(e5)*cos(e6)*sin(e4)*sin(e5) - 2*I6zx*de3*cos(e4)*cos(e5)*cos(e6)*sin(e4)*sin(e5) + 2*I6xy*de1*cos(e4)*cos(e5)*sin(e2)*sin(e3)*sin(e4) + I6xx*de6*cos(e5)*cos(e6)*sin(e4)*sin(e5)*sin(e6) + 2*I6yz*de2*cos(e4)*cos(e5)*sin(e4)*sin(e5)*sin(e6) + 2*I6yz*de3*cos(e4)*cos(e5)*sin(e4)*sin(e5)*sin(e6) - I6yy*de6*cos(e5)*cos(e6)*sin(e4)*sin(e5)*sin(e6) + 2*I5zx*de1*cos(e4)*cos(e5)*sin(e2)*sin(e3)*sin(e4) - I6zx*de1*cos(e2)*cos(e5)*sin(e3)*sin(e4)*sin(e6) - I6zx*de1*cos(e3)*cos(e5)*sin(e2)*sin(e4)*sin(e6) - I6xx*de1*cos(e4)^2*cos(e5)^2*cos(e6)^2*sin(e2)*sin(e3) + I6yy*de1*cos(e4)^2*cos(e5)^2*cos(e6)^2*sin(e2)*sin(e3) - 2*I5yz*de1*cos(e4)*sin(e2)*sin(e3)*sin(e4)*sin(e5) + de5*m6*x6^2*cos(e4)*cos(e5)*cos(e6)*sin(e6) + 4*de2*m6*x6*y6*cos(e4)^2*cos(e5)*cos(e6)^2 + 4*de3*m6*x6*y6*cos(e4)^2*cos(e5)*cos(e6)^2 - de5*m6*y6^2*cos(e4)*cos(e5)*cos(e6)*sin(e6) - a3*de1*m4*x4*cos(e2)*cos(e3)*cos(e4) + 2*I5xy*de1*cos(e2)*cos(e3)*cos(e4)^2*cos(e5)*sin(e5) + 2*I6xy*de1*cos(e2)*cos(e3)*cos(e4)^2*cos(e6)*sin(e6) + 2*I6zx*de1*cos(e2)*cos(e4)*cos(e5)^2*cos(e6)*sin(e3) + 2*I6zx*de1*cos(e3)*cos(e4)*cos(e5)^2*cos(e6)*sin(e2) + a3*de2*m6*x6*cos(e5)*cos(e6)*sin(e4) + a3*de3*m6*x6*cos(e5)*cos(e6)*sin(e4) + a3*de1*m4*y4*cos(e2)*cos(e3)*sin(e4) - a3*de1*m5*z5*cos(e2)*cos(e3)*sin(e4) + d4*de1*m4*x4*cos(e2)*cos(e4)*sin(e3) + d4*de1*m4*x4*cos(e3)*cos(e4)*sin(e2) - 2*I6xy*de2*cos(e4)*cos(e5)^2*cos(e6)*sin(e4)*sin(e6) - 2*I6xy*de3*cos(e4)*cos(e5)^2*cos(e6)*sin(e4)*sin(e6) - 2*I6yz*de1*cos(e2)*cos(e4)*cos(e5)^2*sin(e3)*sin(e6) - 2*I6yz*de1*cos(e3)*cos(e4)*cos(e5)^2*sin(e2)*sin(e6) + a3*de1*m4*x4*cos(e4)*sin(e2)*sin(e3) - a3*de2*m6*y6*cos(e5)*sin(e4)*sin(e6) - a3*de3*m6*y6*cos(e5)*sin(e4)*sin(e6) - 2*I5xy*de1*cos(e4)^2*cos(e5)*sin(e2)*sin(e3)*sin(e5) - 2*I6xy*de1*cos(e2)*cos(e6)^2*sin(e3)*sin(e4)*sin(e5) - 2*I6xy*de1*cos(e3)*cos(e6)^2*sin(e2)*sin(e4)*sin(e5) - 2*I6xy*de1*cos(e4)^2*cos(e6)*sin(e2)*sin(e3)*sin(e6) - d4*de1*m4*y4*cos(e2)*sin(e3)*sin(e4) - d4*de1*m4*y4*cos(e3)*sin(e2)*sin(e4) + d4*de1*m5*z5*cos(e2)*sin(e3)*sin(e4) + d4*de1*m5*z5*cos(e3)*sin(e2)*sin(e4) - de1*m5*x5*y5*cos(e2)*cos(e4)*sin(e3) - de1*m5*x5*y5*cos(e3)*cos(e4)*sin(e2) + de1*m4*x4*z4*cos(e2)*cos(e4)*sin(e3) + de1*m4*x4*z4*cos(e3)*cos(e4)*sin(e2) - de5*m6*y6*z6*cos(e4)*cos(e6)*sin(e5) - a3*de1*m4*y4*sin(e2)*sin(e3)*sin(e4) + a3*de1*m5*z5*sin(e2)*sin(e3)*sin(e4) + 2*de2*m6*x6^2*cos(e4)^2*cos(e5)*cos(e6)*sin(e6) + 2*de3*m6*x6^2*cos(e4)^2*cos(e5)*cos(e6)*sin(e6) - 2*de2*m6*y6^2*cos(e4)^2*cos(e5)*cos(e6)*sin(e6) - 2*de3*m6*y6^2*cos(e4)^2*cos(e5)*cos(e6)*sin(e6) - 2*de5*m5*x5*y5*cos(e5)*sin(e4)*sin(e5) + de6*m6*x6*y6*cos(e5)*sin(e4)*sin(e5) - de5*m6*x6*z6*cos(e4)*sin(e5)*sin(e6) - de1*m4*y4*z4*cos(e2)*sin(e3)*sin(e4) - de1*m4*y4*z4*cos(e3)*sin(e2)*sin(e4) + 2*de5*m6*x6*y6*cos(e4)*cos(e5)*cos(e6)^2 - de1*m5*x5^2*cos(e2)*cos(e3)*cos(e4)^2*cos(e5)^2 - de1*m6*x6^2*cos(e2)*cos(e3)*cos(e4)^2*cos(e6)^2 + de1*m5*y5^2*cos(e2)*cos(e3)*cos(e4)^2*cos(e5)^2 - de1*m6*y6^2*cos(e2)*cos(e3)*cos(e4)^2*cos(e5)^2 + de1*m6*y6^2*cos(e2)*cos(e3)*cos(e4)^2*cos(e6)^2 + de1*m6*z6^2*cos(e2)*cos(e3)*cos(e4)^2*cos(e5)^2 - 2*de2*m6*y6*z6*cos(e4)^2*cos(e6)*sin(e5) - 2*de3*m6*y6*z6*cos(e4)^2*cos(e6)*sin(e5) - de6*m6*y6*z6*cos(e5)^2*cos(e6)*sin(e4) + de2*m6*x6^2*cos(e4)*cos(e5)^2*cos(e6)^2*sin(e4) + de3*m6*x6^2*cos(e4)*cos(e5)^2*cos(e6)^2*sin(e4) - de2*m6*y6^2*cos(e4)*cos(e5)^2*cos(e6)^2*sin(e4) - de3*m6*y6^2*cos(e4)*cos(e5)^2*cos(e6)^2*sin(e4) - 2*de2*m6*x6*z6*cos(e4)^2*sin(e5)*sin(e6) - 2*de3*m6*x6*z6*cos(e4)^2*sin(e5)*sin(e6) - de6*m6*x6*z6*cos(e5)^2*sin(e4)*sin(e6) + 2*I6zx*de1*cos(e4)*sin(e2)*sin(e3)*sin(e4)*sin(e5)*sin(e6) - de1*m6*x6^2*cos(e2)*cos(e3)*cos(e4)^2*cos(e5)^2*cos(e6)^2 + de1*m6*y6^2*cos(e2)*cos(e3)*cos(e4)^2*cos(e5)^2*cos(e6)^2 + de1*m5*x5^2*cos(e2)*cos(e4)*cos(e5)*sin(e3)*sin(e5) + de1*m5*x5^2*cos(e3)*cos(e4)*cos(e5)*sin(e2)*sin(e5) - de1*m5*y5^2*cos(e2)*cos(e4)*cos(e5)*sin(e3)*sin(e5) - de1*m5*y5^2*cos(e3)*cos(e4)*cos(e5)*sin(e2)*sin(e5) + de1*m6*y6^2*cos(e2)*cos(e4)*cos(e5)*sin(e3)*sin(e5) + de1*m6*y6^2*cos(e3)*cos(e4)*cos(e5)*sin(e2)*sin(e5) - de1*m6*z6^2*cos(e2)*cos(e4)*cos(e5)*sin(e3)*sin(e5) - de1*m6*z6^2*cos(e3)*cos(e4)*cos(e5)*sin(e2)*sin(e5) - de6*m6*x6^2*cos(e5)*cos(e6)*sin(e4)*sin(e5)*sin(e6) + de6*m6*y6^2*cos(e5)*cos(e6)*sin(e4)*sin(e5)*sin(e6) - a3*de1*m5*x5*cos(e2)*cos(e3)*cos(e4)*cos(e5) + 4*I6xy*de1*cos(e2)*cos(e3)*cos(e4)*cos(e5)*cos(e6)^2*sin(e4) + 2*I6zx*de1*cos(e2)*cos(e3)*cos(e4)^2*cos(e5)*cos(e6)*sin(e5) + de1*m6*x6^2*cos(e4)^2*cos(e5)^2*cos(e6)^2*sin(e2)*sin(e3) - de1*m6*y6^2*cos(e4)^2*cos(e5)^2*cos(e6)^2*sin(e2)*sin(e3) + a3*de1*m5*y5*cos(e2)*cos(e3)*cos(e4)*sin(e5) + a3*de1*m6*y6*cos(e2)*cos(e3)*cos(e6)*sin(e4) + a3*de1*m6*z6*cos(e2)*cos(e3)*cos(e4)*sin(e5) + d4*de1*m5*x5*cos(e2)*cos(e4)*cos(e5)*sin(e3) + d4*de1*m5*x5*cos(e3)*cos(e4)*cos(e5)*sin(e2) - I6xx*de1*cos(e2)*cos(e4)*cos(e5)*cos(e6)^2*sin(e3)*sin(e5) - I6xx*de1*cos(e3)*cos(e4)*cos(e5)*cos(e6)^2*sin(e2)*sin(e5) + I6yy*de1*cos(e2)*cos(e4)*cos(e5)*cos(e6)^2*sin(e3)*sin(e5) + I6yy*de1*cos(e3)*cos(e4)*cos(e5)*cos(e6)^2*sin(e2)*sin(e5) - 2*I6yz*de1*cos(e2)*cos(e3)*cos(e4)^2*cos(e5)*sin(e5)*sin(e6) + a3*de1*m5*x5*cos(e4)*cos(e5)*sin(e2)*sin(e3) + a3*de1*m6*x6*cos(e2)*cos(e3)*sin(e4)*sin(e6) - 4*I6xy*de1*cos(e4)*cos(e5)*cos(e6)^2*sin(e2)*sin(e3)*sin(e4) - 2*I6zx*de1*cos(e4)^2*cos(e5)*cos(e6)*sin(e2)*sin(e3)*sin(e5) - d4*de1*m5*y5*cos(e2)*cos(e4)*sin(e3)*sin(e5) - d4*de1*m5*y5*cos(e3)*cos(e4)*sin(e2)*sin(e5) - d4*de1*m6*y6*cos(e2)*cos(e6)*sin(e3)*sin(e4) - d4*de1*m6*y6*cos(e3)*cos(e6)*sin(e2)*sin(e4) - d4*de1*m6*z6*cos(e2)*cos(e4)*sin(e3)*sin(e5) - d4*de1*m6*z6*cos(e3)*cos(e4)*sin(e2)*sin(e5) + 2*de1*m4*x4*y4*cos(e2)*cos(e3)*cos(e4)*sin(e4) - 2*de1*m6*x6*y6*cos(e2)*cos(e3)*cos(e6)*sin(e6) - de1*m6*x6*z6*cos(e2)*cos(e4)*cos(e6)*sin(e3) - de1*m6*x6*z6*cos(e3)*cos(e4)*cos(e6)*sin(e2) - a3*de1*m5*y5*cos(e4)*sin(e2)*sin(e3)*sin(e5) - a3*de1*m6*y6*cos(e6)*sin(e2)*sin(e3)*sin(e4) - a3*de1*m6*z6*cos(e4)*sin(e2)*sin(e3)*sin(e5) - d4*de1*m6*x6*cos(e2)*sin(e3)*sin(e4)*sin(e6) - d4*de1*m6*x6*cos(e3)*sin(e2)*sin(e4)*sin(e6) + 2*I6yz*de1*cos(e4)^2*cos(e5)*sin(e2)*sin(e3)*sin(e5)*sin(e6) - 2*de2*m5*x5*y5*cos(e4)*cos(e5)*sin(e4)*sin(e5) - 2*de3*m5*x5*y5*cos(e4)*cos(e5)*sin(e4)*sin(e5) - 2*de2*m6*x6*y6*cos(e4)*cos(e6)*sin(e4)*sin(e6) - 2*de3*m6*x6*y6*cos(e4)*cos(e6)*sin(e4)*sin(e6) - 2*de6*m6*x6*y6*cos(e4)*cos(e6)*sin(e5)*sin(e6) - 2*de5*m6*x6*z6*cos(e5)*cos(e6)*sin(e4)*sin(e5) + de1*m5*y5*z5*cos(e2)*cos(e5)*sin(e3)*sin(e4) + de1*m5*y5*z5*cos(e3)*cos(e5)*sin(e2)*sin(e4) + de1*m6*y6*z6*cos(e2)*cos(e4)*sin(e3)*sin(e6) + de1*m6*y6*z6*cos(e3)*cos(e4)*sin(e2)*sin(e6) - a3*de1*m6*x6*sin(e2)*sin(e3)*sin(e4)*sin(e6) - 2*de1*m4*x4*y4*cos(e4)*sin(e2)*sin(e3)*sin(e4) + de1*m6*x6*y6*cos(e2)*sin(e3)*sin(e4)*sin(e5) + de1*m6*x6*y6*cos(e3)*sin(e2)*sin(e4)*sin(e5) + 2*de1*m6*x6*y6*cos(e6)*sin(e2)*sin(e3)*sin(e6) + de1*m5*x5*z5*cos(e2)*sin(e3)*sin(e4)*sin(e5) + de1*m5*x5*z5*cos(e3)*sin(e2)*sin(e4)*sin(e5) + 2*de5*m6*y6*z6*cos(e5)*sin(e4)*sin(e5)*sin(e6) + 2*I6xy*de1*cos(e2)*cos(e3)*cos(e4)^2*cos(e5)^2*cos(e6)*sin(e6) - 2*I6xy*de1*cos(e4)^2*cos(e5)^2*cos(e6)*sin(e2)*sin(e3)*sin(e6) + 2*de1*m5*x5*y5*cos(e2)*cos(e4)*cos(e5)^2*sin(e3) + 2*de1*m5*x5*y5*cos(e3)*cos(e4)*cos(e5)^2*sin(e2) - 2*de5*m6*x6*y6*cos(e5)^2*cos(e6)*sin(e4)*sin(e6) - 2*de6*m6*x6*y6*cos(e5)*cos(e6)^2*sin(e4)*sin(e5) - 2*I6yz*de1*cos(e2)*cos(e3)*cos(e4)*cos(e6)*sin(e4)*sin(e5) - 2*I6zx*de1*cos(e2)*cos(e3)*cos(e4)*sin(e4)*sin(e5)*sin(e6) + I6xx*de1*cos(e2)*cos(e6)*sin(e3)*sin(e4)*sin(e5)*sin(e6) + I6xx*de1*cos(e3)*cos(e6)*sin(e2)*sin(e4)*sin(e5)*sin(e6) + 2*I6yz*de1*cos(e4)*cos(e6)*sin(e2)*sin(e3)*sin(e4)*sin(e5) - I6yy*de1*cos(e2)*cos(e6)*sin(e3)*sin(e4)*sin(e5)*sin(e6) - I6yy*de1*cos(e3)*cos(e6)*sin(e2)*sin(e4)*sin(e5)*sin(e6) + a3*de1*m6*y6*cos(e2)*cos(e3)*cos(e4)*cos(e5)*sin(e6) + d4*de1*m6*x6*cos(e2)*cos(e4)*cos(e5)*cos(e6)*sin(e3) + d4*de1*m6*x6*cos(e3)*cos(e4)*cos(e5)*cos(e6)*sin(e2) + a3*de1*m6*x6*cos(e4)*cos(e5)*cos(e6)*sin(e2)*sin(e3) - d4*de1*m6*y6*cos(e2)*cos(e4)*cos(e5)*sin(e3)*sin(e6) - d4*de1*m6*y6*cos(e3)*cos(e4)*cos(e5)*sin(e2)*sin(e6) - 2*de1*m6*x6*y6*cos(e2)*cos(e3)*cos(e4)*cos(e5)*sin(e4) - 2*de1*m5*x5*z5*cos(e2)*cos(e3)*cos(e4)*cos(e5)*sin(e4) - a3*de1*m6*y6*cos(e4)*cos(e5)*sin(e2)*sin(e3)*sin(e6) - 2*de2*m6*x6*z6*cos(e4)*cos(e5)*cos(e6)*sin(e4)*sin(e5) - 2*de3*m6*x6*z6*cos(e4)*cos(e5)*cos(e6)*sin(e4)*sin(e5) + 2*de1*m5*y5*z5*cos(e2)*cos(e3)*cos(e4)*sin(e4)*sin(e5) - de1*m6*y6*z6*cos(e2)*cos(e5)*cos(e6)*sin(e3)*sin(e4) - de1*m6*y6*z6*cos(e3)*cos(e5)*cos(e6)*sin(e2)*sin(e4) + de1*m6*x6^2*cos(e2)*cos(e4)*cos(e5)*cos(e6)^2*sin(e3)*sin(e5) + de1*m6*x6^2*cos(e3)*cos(e4)*cos(e5)*cos(e6)^2*sin(e2)*sin(e5) - de1*m6*y6^2*cos(e2)*cos(e4)*cos(e5)*cos(e6)^2*sin(e3)*sin(e5) - de1*m6*y6^2*cos(e3)*cos(e4)*cos(e5)*cos(e6)^2*sin(e2)*sin(e5) + 2*de1*m6*x6*y6*cos(e4)*cos(e5)*sin(e2)*sin(e3)*sin(e4) + 2*de1*m5*x5*z5*cos(e4)*cos(e5)*sin(e2)*sin(e3)*sin(e4) - de1*m6*x6*z6*cos(e2)*cos(e5)*sin(e3)*sin(e4)*sin(e6) - de1*m6*x6*z6*cos(e3)*cos(e5)*sin(e2)*sin(e4)*sin(e6) + 2*de2*m6*y6*z6*cos(e4)*cos(e5)*sin(e4)*sin(e5)*sin(e6) + 2*de3*m6*y6*z6*cos(e4)*cos(e5)*sin(e4)*sin(e5)*sin(e6) - 2*de1*m5*y5*z5*cos(e4)*sin(e2)*sin(e3)*sin(e4)*sin(e5) + 2*de1*m5*x5*y5*cos(e2)*cos(e3)*cos(e4)^2*cos(e5)*sin(e5) + 2*de1*m6*x6*y6*cos(e2)*cos(e3)*cos(e4)^2*cos(e6)*sin(e6) + 2*de1*m6*x6*z6*cos(e2)*cos(e4)*cos(e5)^2*cos(e6)*sin(e3) + 2*de1*m6*x6*z6*cos(e3)*cos(e4)*cos(e5)^2*cos(e6)*sin(e2) - 2*de2*m6*x6*y6*cos(e4)*cos(e5)^2*cos(e6)*sin(e4)*sin(e6) - 2*de3*m6*x6*y6*cos(e4)*cos(e5)^2*cos(e6)*sin(e4)*sin(e6) - 2*de1*m6*y6*z6*cos(e2)*cos(e4)*cos(e5)^2*sin(e3)*sin(e6) - 2*de1*m6*y6*z6*cos(e3)*cos(e4)*cos(e5)^2*sin(e2)*sin(e6) - 2*de1*m5*x5*y5*cos(e4)^2*cos(e5)*sin(e2)*sin(e3)*sin(e5) - 2*de1*m6*x6*y6*cos(e2)*cos(e6)^2*sin(e3)*sin(e4)*sin(e5) - 2*de1*m6*x6*y6*cos(e3)*cos(e6)^2*sin(e2)*sin(e4)*sin(e5) - 2*de1*m6*x6*y6*cos(e4)^2*cos(e6)*sin(e2)*sin(e3)*sin(e6) - 2*I6xx*de1*cos(e2)*cos(e3)*cos(e4)*cos(e5)*cos(e6)*sin(e4)*sin(e6) + 2*I6yy*de1*cos(e2)*cos(e3)*cos(e4)*cos(e5)*cos(e6)*sin(e4)*sin(e6) - 2*I6xy*de1*cos(e2)*cos(e4)*cos(e5)*cos(e6)*sin(e3)*sin(e5)*sin(e6) - 2*I6xy*de1*cos(e3)*cos(e4)*cos(e5)*cos(e6)*sin(e2)*sin(e5)*sin(e6) + 2*I6xx*de1*cos(e4)*cos(e5)*cos(e6)*sin(e2)*sin(e3)*sin(e4)*sin(e6) - 2*I6yy*de1*cos(e4)*cos(e5)*cos(e6)*sin(e2)*sin(e3)*sin(e4)*sin(e6) - a3*de1*m6*x6*cos(e2)*cos(e3)*cos(e4)*cos(e5)*cos(e6) - de1*m6*x6^2*cos(e2)*cos(e6)*sin(e3)*sin(e4)*sin(e5)*sin(e6) - de1*m6*x6^2*cos(e3)*cos(e6)*sin(e2)*sin(e4)*sin(e5)*sin(e6) + de1*m6*y6^2*cos(e2)*cos(e6)*sin(e3)*sin(e4)*sin(e5)*sin(e6) + de1*m6*y6^2*cos(e3)*cos(e6)*sin(e2)*sin(e4)*sin(e5)*sin(e6) - 2*de1*m6*x6*z6*cos(e2)*cos(e3)*cos(e4)*sin(e4)*sin(e5)*sin(e6) + 2*de1*m6*y6*z6*cos(e4)*cos(e6)*sin(e2)*sin(e3)*sin(e4)*sin(e5) + 2*de1*m6*x6*z6*cos(e4)*sin(e2)*sin(e3)*sin(e4)*sin(e5)*sin(e6) + 4*de1*m6*x6*y6*cos(e2)*cos(e3)*cos(e4)*cos(e5)*cos(e6)^2*sin(e4) + 2*de1*m6*x6*z6*cos(e2)*cos(e3)*cos(e4)^2*cos(e5)*cos(e6)*sin(e5) - 2*de1*m6*y6*z6*cos(e2)*cos(e3)*cos(e4)^2*cos(e5)*sin(e5)*sin(e6) - 4*de1*m6*x6*y6*cos(e4)*cos(e5)*cos(e6)^2*sin(e2)*sin(e3)*sin(e4) - 2*de1*m6*x6*z6*cos(e4)^2*cos(e5)*cos(e6)*sin(e2)*sin(e3)*sin(e5) + 2*de1*m6*y6*z6*cos(e4)^2*cos(e5)*sin(e2)*sin(e3)*sin(e5)*sin(e6) + 2*de1*m6*x6^2*cos(e2)*cos(e3)*cos(e4)*cos(e5)*cos(e6)*sin(e4)*sin(e6) + 2*de1*m6*x6*y6*cos(e2)*cos(e3)*cos(e4)^2*cos(e5)^2*cos(e6)*sin(e6) - 2*de1*m6*y6^2*cos(e2)*cos(e3)*cos(e4)*cos(e5)*cos(e6)*sin(e4)*sin(e6) - 2*de1*m6*x6^2*cos(e4)*cos(e5)*cos(e6)*sin(e2)*sin(e3)*sin(e4)*sin(e6) - 2*de1*m6*x6*y6*cos(e4)^2*cos(e5)^2*cos(e6)*sin(e2)*sin(e3)*sin(e6) + 2*de1*m6*y6^2*cos(e4)*cos(e5)*cos(e6)*sin(e2)*sin(e3)*sin(e4)*sin(e6) - 2*de1*m6*y6*z6*cos(e2)*cos(e3)*cos(e4)*cos(e6)*sin(e4)*sin(e5) - 2*de1*m6*x6*y6*cos(e2)*cos(e4)*cos(e5)*cos(e6)*sin(e3)*sin(e5)*sin(e6) - 2*de1*m6*x6*y6*cos(e3)*cos(e4)*cos(e5)*cos(e6)*sin(e2)*sin(e5)*sin(e6),(de5*(2*I5xy + 2*I6zx*cos(e6) - 2*I6yz*sin(e6) - 4*I5xy*cos(e5)^2 + I5xx*sin(2*e5) - I5yy*sin(2*e5) + I6yy*sin(2*e5) - I6zz*sin(2*e5) - 4*I6zx*cos(e5)^2*cos(e6) + 4*I6yz*cos(e5)^2*sin(e6) + 2*m5*x5*y5 - m5*x5^2*sin(2*e5) + m5*y5^2*sin(2*e5) - m6*y6^2*sin(2*e5) + m6*z6^2*sin(2*e5) + 2*I6xx*cos(e5)*cos(e6)^2*sin(e5) - 2*I6yy*cos(e5)*cos(e6)^2*sin(e5) + 2*m6*x6*z6*cos(e6) - 2*m6*y6*z6*sin(e6) - 4*m5*x5*y5*cos(e5)^2 - 2*m6*x6^2*cos(e5)*cos(e6)^2*sin(e5) + 2*m6*y6^2*cos(e5)*cos(e6)^2*sin(e5) - 4*m6*x6*z6*cos(e5)^2*cos(e6) + 4*m6*y6*z6*cos(e5)^2*sin(e6) + 4*I6xy*cos(e5)*cos(e6)*sin(e5)*sin(e6) + 4*m6*x6*y6*cos(e5)*cos(e6)*sin(e5)*sin(e6)))/2 + (de6*(2*I6xy*cos(2*e6) - I6xx*sin(2*e6) + I6yy*sin(2*e6) + 2*I6xy*cos(e5)^2*sin(e6)^2 + m6*x6^2*sin(2*e6) - m6*y6^2*sin(2*e6) - 2*I6xy*cos(e5)^2*cos(e6)^2 + 2*I6yz*cos(e5)*cos(e6)*sin(e5) + 2*I6zx*cos(e5)*sin(e5)*sin(e6) + 2*I6xx*cos(e5)^2*cos(e6)*sin(e6) - 2*I6yy*cos(e5)^2*cos(e6)*sin(e6) + 2*m6*x6*y6*cos(2*e6) - 2*m6*x6*y6*cos(e5)^2*cos(e6)^2 + 2*m6*x6*y6*cos(e5)^2*sin(e6)^2 - 2*m6*x6^2*cos(e5)^2*cos(e6)*sin(e6) + 2*m6*y6^2*cos(e5)^2*cos(e6)*sin(e6) + 2*m6*y6*z6*cos(e5)*cos(e6)*sin(e5) + 2*m6*x6*z6*cos(e5)*sin(e5)*sin(e6)))/2,I5xy*de4 - 2*I5xy*de4*cos(e5)^2 + (I5xx*de4*sin(2*e5))/2 - (I5yy*de4*sin(2*e5))/2 + (I6yy*de4*sin(2*e5))/2 - (I6zz*de4*sin(2*e5))/2 - I6xy*de5*cos(e5) - I5zx*de5*cos(e5) + I6zx*de4*cos(e6) + (I5xx*de2*sin(e4))/2 + (I5xx*de3*sin(e4))/2 + (I6xx*de2*sin(e4))/2 + (I6xx*de3*sin(e4))/2 + (I6xx*de6*sin(e5))/2 - (I5yy*de2*sin(e4))/2 - (I5yy*de3*sin(e4))/2 + (I6yy*de2*sin(e4))/2 + (I6yy*de3*sin(e4))/2 + I5yz*de5*sin(e5) - (I6yy*de6*sin(e5))/2 - I6yz*de4*sin(e6) + (I5zz*de2*sin(e4))/2 + (I5zz*de3*sin(e4))/2 - (I6zz*de2*sin(e4))/2 - (I6zz*de3*sin(e4))/2 - (I6zz*de6*sin(e5))/2 - I5xx*de2*cos(e5)^2*sin(e4) - I5xx*de3*cos(e5)^2*sin(e4) - I6xx*de6*cos(e6)^2*sin(e5) + I5yy*de2*cos(e5)^2*sin(e4) + I5yy*de3*cos(e5)^2*sin(e4) - I6yy*de2*cos(e5)^2*sin(e4) - I6yy*de3*cos(e5)^2*sin(e4) + 2*I6yz*de4*cos(e5)^2*sin(e6) + I6yy*de6*cos(e6)^2*sin(e5) + I6zz*de2*cos(e5)^2*sin(e4) + I6zz*de3*cos(e5)^2*sin(e4) + de4*m5*x5*y5 - (de4*m5*x5^2*sin(2*e5))/2 + (de4*m5*y5^2*sin(2*e5))/2 - (de4*m6*y6^2*sin(2*e5))/2 + (de4*m6*z6^2*sin(2*e5))/2 - I6xy*de2*cos(e4)*cos(e5) - I6xy*de3*cos(e4)*cos(e5) - I5zx*de2*cos(e4)*cos(e5) - I5zx*de3*cos(e4)*cos(e5) - I5xy*de1*cos(e2)*sin(e3) - I5xy*de1*cos(e3)*sin(e2) + I5yz*de2*cos(e4)*sin(e5) + I5yz*de3*cos(e4)*sin(e5) - I6yz*de5*cos(e6)*sin(e5) - I6zx*de5*sin(e5)*sin(e6) - de6*m6*x6^2*sin(e5) + de2*m5*y5^2*sin(e4) + de3*m5*y5^2*sin(e4) + de2*m6*z6^2*sin(e4) + de3*m6*z6^2*sin(e4) + 2*I6xy*de5*cos(e5)*cos(e6)^2 - 2*I6zx*de4*cos(e5)^2*cos(e6) + de2*m5*x5^2*cos(e5)^2*sin(e4) + de3*m5*x5^2*cos(e5)^2*sin(e4) + de6*m6*x6^2*cos(e6)^2*sin(e5) - de2*m5*y5^2*cos(e5)^2*sin(e4) - de3*m5*y5^2*cos(e5)^2*sin(e4) + de2*m6*y6^2*cos(e5)^2*sin(e4) + de3*m6*y6^2*cos(e5)^2*sin(e4) - de6*m6*y6^2*cos(e6)^2*sin(e5) - de2*m6*z6^2*cos(e5)^2*sin(e4) - de3*m6*z6^2*cos(e5)^2*sin(e4) - I6xx*de2*cos(e5)^2*cos(e6)^2*sin(e4) - I6xx*de3*cos(e5)^2*cos(e6)^2*sin(e4) + I6yy*de2*cos(e5)^2*cos(e6)^2*sin(e4) + I6yy*de3*cos(e5)^2*cos(e6)^2*sin(e4) - 2*de4*m5*x5*y5*cos(e5)^2 - (I5xx*de1*cos(e2)*cos(e3)*cos(e4))/2 - (I6xx*de1*cos(e2)*cos(e3)*cos(e4))/2 + (I5yy*de1*cos(e2)*cos(e3)*cos(e4))/2 - (I6yy*de1*cos(e2)*cos(e3)*cos(e4))/2 - (I5zz*de1*cos(e2)*cos(e3)*cos(e4))/2 + (I6zz*de1*cos(e2)*cos(e3)*cos(e4))/2 - I6xx*de5*cos(e5)*cos(e6)*sin(e6) - I6yz*de2*cos(e4)*cos(e6)*sin(e5) - I6yz*de3*cos(e4)*cos(e6)*sin(e5) + I6yy*de5*cos(e5)*cos(e6)*sin(e6) - I6zx*de1*cos(e2)*cos(e6)*sin(e3) - I6zx*de1*cos(e3)*cos(e6)*sin(e2) + (I5xx*de1*cos(e4)*sin(e2)*sin(e3))/2 + (I6xx*de1*cos(e4)*sin(e2)*sin(e3))/2 - 2*I5xy*de2*cos(e5)*sin(e4)*sin(e5) - 2*I5xy*de3*cos(e5)*sin(e4)*sin(e5) - 2*I6xy*de6*cos(e6)*sin(e5)*sin(e6) - (I5yy*de1*cos(e4)*sin(e2)*sin(e3))/2 + (I6yy*de1*cos(e4)*sin(e2)*sin(e3))/2 + I6yz*de1*cos(e2)*sin(e3)*sin(e6) + I6yz*de1*cos(e3)*sin(e2)*sin(e6) + (I5zz*de1*cos(e4)*sin(e2)*sin(e3))/2 - (I6zz*de1*cos(e4)*sin(e2)*sin(e3))/2 - I6zx*de2*cos(e4)*sin(e5)*sin(e6) - I6zx*de3*cos(e4)*sin(e5)*sin(e6) + 2*I6xy*de2*cos(e4)*cos(e5)*cos(e6)^2 + 2*I6xy*de3*cos(e4)*cos(e5)*cos(e6)^2 + 2*I5xy*de1*cos(e2)*cos(e5)^2*sin(e3) + 2*I5xy*de1*cos(e3)*cos(e5)^2*sin(e2) + I6xx*de4*cos(e5)*cos(e6)^2*sin(e5) - I6yy*de4*cos(e5)*cos(e6)^2*sin(e5) - de5*m6*x6*y6*cos(e5) - de5*m5*x5*z5*cos(e5) + de4*m6*x6*z6*cos(e6) + de5*m5*y5*z5*sin(e5) - de4*m6*y6*z6*sin(e6) + 2*de5*m6*x6*y6*cos(e5)*cos(e6)^2 - 2*de4*m6*x6*z6*cos(e5)^2*cos(e6) + 2*de4*m6*y6*z6*cos(e5)^2*sin(e6) + de2*m6*x6^2*cos(e5)^2*cos(e6)^2*sin(e4) + de3*m6*x6^2*cos(e5)^2*cos(e6)^2*sin(e4) - de2*m6*y6^2*cos(e5)^2*cos(e6)^2*sin(e4) - de3*m6*y6^2*cos(e5)^2*cos(e6)^2*sin(e4) - I6xy*de1*cos(e2)*cos(e3)*cos(e5)*sin(e4) - I6xx*de2*cos(e4)*cos(e5)*cos(e6)*sin(e6) - I6xx*de3*cos(e4)*cos(e5)*cos(e6)*sin(e6) + I6yy*de2*cos(e4)*cos(e5)*cos(e6)*sin(e6) + I6yy*de3*cos(e4)*cos(e5)*cos(e6)*sin(e6) - I5zx*de1*cos(e2)*cos(e3)*cos(e5)*sin(e4) - I5xx*de1*cos(e2)*cos(e5)*sin(e3)*sin(e5) - I5xx*de1*cos(e3)*cos(e5)*sin(e2)*sin(e5) + 2*I6xy*de4*cos(e5)*cos(e6)*sin(e5)*sin(e6) + I5yy*de1*cos(e2)*cos(e5)*sin(e3)*sin(e5) + I5yy*de1*cos(e3)*cos(e5)*sin(e2)*sin(e5) + I5yz*de1*cos(e2)*cos(e3)*sin(e4)*sin(e5) - I6yy*de1*cos(e2)*cos(e5)*sin(e3)*sin(e5) - I6yy*de1*cos(e3)*cos(e5)*sin(e2)*sin(e5) + I6zz*de1*cos(e2)*cos(e5)*sin(e3)*sin(e5) + I6zz*de1*cos(e3)*cos(e5)*sin(e2)*sin(e5) - 2*I6zx*de2*cos(e5)*cos(e6)*sin(e4)*sin(e5) - 2*I6zx*de3*cos(e5)*cos(e6)*sin(e4)*sin(e5) + I6xy*de1*cos(e5)*sin(e2)*sin(e3)*sin(e4) + 2*I6yz*de2*cos(e5)*sin(e4)*sin(e5)*sin(e6) + 2*I6yz*de3*cos(e5)*sin(e4)*sin(e5)*sin(e6) + I5zx*de1*cos(e5)*sin(e2)*sin(e3)*sin(e4) - de1*m5*y5^2*cos(e2)*cos(e3)*cos(e4) - de1*m6*z6^2*cos(e2)*cos(e3)*cos(e4) - I5yz*de1*sin(e2)*sin(e3)*sin(e4)*sin(e5) + de5*m6*x6^2*cos(e5)*cos(e6)*sin(e6) - de5*m6*y6^2*cos(e5)*cos(e6)*sin(e6) + de1*m5*y5^2*cos(e4)*sin(e2)*sin(e3) + de1*m6*z6^2*cos(e4)*sin(e2)*sin(e3) + I5xx*de1*cos(e2)*cos(e3)*cos(e4)*cos(e5)^2 - I5yy*de1*cos(e2)*cos(e3)*cos(e4)*cos(e5)^2 + I6yy*de1*cos(e2)*cos(e3)*cos(e4)*cos(e5)^2 - I6zz*de1*cos(e2)*cos(e3)*cos(e4)*cos(e5)^2 + 2*I6zx*de1*cos(e2)*cos(e5)^2*cos(e6)*sin(e3) + 2*I6zx*de1*cos(e3)*cos(e5)^2*cos(e6)*sin(e2) - I5xx*de1*cos(e4)*cos(e5)^2*sin(e2)*sin(e3) - 2*I6xy*de2*cos(e5)^2*cos(e6)*sin(e4)*sin(e6) - 2*I6xy*de3*cos(e5)^2*cos(e6)*sin(e4)*sin(e6) + I5yy*de1*cos(e4)*cos(e5)^2*sin(e2)*sin(e3) - I6yy*de1*cos(e4)*cos(e5)^2*sin(e2)*sin(e3) - 2*I6yz*de1*cos(e2)*cos(e5)^2*sin(e3)*sin(e6) - 2*I6yz*de1*cos(e3)*cos(e5)^2*sin(e2)*sin(e6) + I6zz*de1*cos(e4)*cos(e5)^2*sin(e2)*sin(e3) - de2*m6*x6*y6*cos(e4)*cos(e5) - de3*m6*x6*y6*cos(e4)*cos(e5) - de2*m5*x5*z5*cos(e4)*cos(e5) - de3*m5*x5*z5*cos(e4)*cos(e5) - de1*m5*x5*y5*cos(e2)*sin(e3) - de1*m5*x5*y5*cos(e3)*sin(e2) + de2*m5*y5*z5*cos(e4)*sin(e5) + de3*m5*y5*z5*cos(e4)*sin(e5) - de5*m6*y6*z6*cos(e6)*sin(e5) - de4*m6*x6^2*cos(e5)*cos(e6)^2*sin(e5) + de4*m6*y6^2*cos(e5)*cos(e6)^2*sin(e5) - de5*m6*x6*z6*sin(e5)*sin(e6) + 2*I5xy*de1*cos(e2)*cos(e3)*cos(e4)*cos(e5)*sin(e5) - I6yz*de1*cos(e2)*cos(e3)*cos(e6)*sin(e4)*sin(e5) - 2*I5xy*de1*cos(e4)*cos(e5)*sin(e2)*sin(e3)*sin(e5) - I6zx*de1*cos(e2)*cos(e3)*sin(e4)*sin(e5)*sin(e6) + I6yz*de1*cos(e6)*sin(e2)*sin(e3)*sin(e4)*sin(e5) + de2*m6*x6^2*cos(e4)*cos(e5)*cos(e6)*sin(e6) + de3*m6*x6^2*cos(e4)*cos(e5)*cos(e6)*sin(e6) - de2*m6*y6^2*cos(e4)*cos(e5)*cos(e6)*sin(e6) - de3*m6*y6^2*cos(e4)*cos(e5)*cos(e6)*sin(e6) + I6zx*de1*sin(e2)*sin(e3)*sin(e4)*sin(e5)*sin(e6) + de1*m5*x5^2*cos(e2)*cos(e5)*sin(e3)*sin(e5) + de1*m5*x5^2*cos(e3)*cos(e5)*sin(e2)*sin(e5) - de1*m5*y5^2*cos(e2)*cos(e5)*sin(e3)*sin(e5) - de1*m5*y5^2*cos(e3)*cos(e5)*sin(e2)*sin(e5) + de1*m6*y6^2*cos(e2)*cos(e5)*sin(e3)*sin(e5) + de1*m6*y6^2*cos(e3)*cos(e5)*sin(e2)*sin(e5) - de1*m6*z6^2*cos(e2)*cos(e5)*sin(e3)*sin(e5) - de1*m6*z6^2*cos(e3)*cos(e5)*sin(e2)*sin(e5) + 2*I6xy*de1*cos(e2)*cos(e3)*cos(e5)*cos(e6)^2*sin(e4) - I6xx*de1*cos(e2)*cos(e5)*cos(e6)^2*sin(e3)*sin(e5) - I6xx*de1*cos(e3)*cos(e5)*cos(e6)^2*sin(e2)*sin(e5) + I6yy*de1*cos(e2)*cos(e5)*cos(e6)^2*sin(e3)*sin(e5) + I6yy*de1*cos(e3)*cos(e5)*cos(e6)^2*sin(e2)*sin(e5) - 2*I6xy*de1*cos(e5)*cos(e6)^2*sin(e2)*sin(e3)*sin(e4) - de1*m5*x5^2*cos(e2)*cos(e3)*cos(e4)*cos(e5)^2 + de1*m5*y5^2*cos(e2)*cos(e3)*cos(e4)*cos(e5)^2 - de1*m6*y6^2*cos(e2)*cos(e3)*cos(e4)*cos(e5)^2 + de1*m6*z6^2*cos(e2)*cos(e3)*cos(e4)*cos(e5)^2 - de1*m6*x6*z6*cos(e2)*cos(e6)*sin(e3) - de1*m6*x6*z6*cos(e3)*cos(e6)*sin(e2) - de2*m6*y6*z6*cos(e4)*cos(e6)*sin(e5) - de3*m6*y6*z6*cos(e4)*cos(e6)*sin(e5) - 2*de2*m5*x5*y5*cos(e5)*sin(e4)*sin(e5) - 2*de3*m5*x5*y5*cos(e5)*sin(e4)*sin(e5) - 2*de6*m6*x6*y6*cos(e6)*sin(e5)*sin(e6) - de2*m6*x6*z6*cos(e4)*sin(e5)*sin(e6) - de3*m6*x6*z6*cos(e4)*sin(e5)*sin(e6) + de1*m6*y6*z6*cos(e2)*sin(e3)*sin(e6) + de1*m6*y6*z6*cos(e3)*sin(e2)*sin(e6) + de1*m5*x5^2*cos(e4)*cos(e5)^2*sin(e2)*sin(e3) - de1*m5*y5^2*cos(e4)*cos(e5)^2*sin(e2)*sin(e3) + de1*m6*y6^2*cos(e4)*cos(e5)^2*sin(e2)*sin(e3) - de1*m6*z6^2*cos(e4)*cos(e5)^2*sin(e2)*sin(e3) + I6xx*de1*cos(e2)*cos(e3)*cos(e4)*cos(e5)^2*cos(e6)^2 - I6yy*de1*cos(e2)*cos(e3)*cos(e4)*cos(e5)^2*cos(e6)^2 - I6xx*de1*cos(e4)*cos(e5)^2*cos(e6)^2*sin(e2)*sin(e3) + I6yy*de1*cos(e4)*cos(e5)^2*cos(e6)^2*sin(e2)*sin(e3) + 2*de2*m6*x6*y6*cos(e4)*cos(e5)*cos(e6)^2 + 2*de3*m6*x6*y6*cos(e4)*cos(e5)*cos(e6)^2 + 2*de1*m5*x5*y5*cos(e2)*cos(e5)^2*sin(e3) + 2*de1*m5*x5*y5*cos(e3)*cos(e5)^2*sin(e2) + 2*I6xy*de1*cos(e2)*cos(e3)*cos(e4)*cos(e5)^2*cos(e6)*sin(e6) - 2*I6xy*de1*cos(e4)*cos(e5)^2*cos(e6)*sin(e2)*sin(e3)*sin(e6) - de1*m6*x6*y6*cos(e2)*cos(e3)*cos(e5)*sin(e4) - de1*m5*x5*z5*cos(e2)*cos(e3)*cos(e5)*sin(e4) + 2*de4*m6*x6*y6*cos(e5)*cos(e6)*sin(e5)*sin(e6) - 2*de2*m6*x6*z6*cos(e5)*cos(e6)*sin(e4)*sin(e5) - 2*de3*m6*x6*z6*cos(e5)*cos(e6)*sin(e4)*sin(e5) + de1*m5*y5*z5*cos(e2)*cos(e3)*sin(e4)*sin(e5) + de1*m6*x6^2*cos(e2)*cos(e5)*cos(e6)^2*sin(e3)*sin(e5) + de1*m6*x6^2*cos(e3)*cos(e5)*cos(e6)^2*sin(e2)*sin(e5) - de1*m6*y6^2*cos(e2)*cos(e5)*cos(e6)^2*sin(e3)*sin(e5) - de1*m6*y6^2*cos(e3)*cos(e5)*cos(e6)^2*sin(e2)*sin(e5) + de1*m6*x6*y6*cos(e5)*sin(e2)*sin(e3)*sin(e4) + de1*m5*x5*z5*cos(e5)*sin(e2)*sin(e3)*sin(e4) + 2*de2*m6*y6*z6*cos(e5)*sin(e4)*sin(e5)*sin(e6) + 2*de3*m6*y6*z6*cos(e5)*sin(e4)*sin(e5)*sin(e6) - de1*m5*y5*z5*sin(e2)*sin(e3)*sin(e4)*sin(e5) - de1*m6*x6^2*cos(e2)*cos(e3)*cos(e4)*cos(e5)^2*cos(e6)^2 + de1*m6*y6^2*cos(e2)*cos(e3)*cos(e4)*cos(e5)^2*cos(e6)^2 + 2*de1*m6*x6*z6*cos(e2)*cos(e5)^2*cos(e6)*sin(e3) + 2*de1*m6*x6*z6*cos(e3)*cos(e5)^2*cos(e6)*sin(e2) - 2*de2*m6*x6*y6*cos(e5)^2*cos(e6)*sin(e4)*sin(e6) - 2*de3*m6*x6*y6*cos(e5)^2*cos(e6)*sin(e4)*sin(e6) - 2*de1*m6*y6*z6*cos(e2)*cos(e5)^2*sin(e3)*sin(e6) - 2*de1*m6*y6*z6*cos(e3)*cos(e5)^2*sin(e2)*sin(e6) + 2*I6zx*de1*cos(e2)*cos(e3)*cos(e4)*cos(e5)*cos(e6)*sin(e5) + de1*m6*x6^2*cos(e4)*cos(e5)^2*cos(e6)^2*sin(e2)*sin(e3) - de1*m6*y6^2*cos(e4)*cos(e5)^2*cos(e6)^2*sin(e2)*sin(e3) - I6xx*de1*cos(e2)*cos(e3)*cos(e5)*cos(e6)*sin(e4)*sin(e6) + I6yy*de1*cos(e2)*cos(e3)*cos(e5)*cos(e6)*sin(e4)*sin(e6) - 2*I6yz*de1*cos(e2)*cos(e3)*cos(e4)*cos(e5)*sin(e5)*sin(e6) - 2*I6xy*de1*cos(e2)*cos(e5)*cos(e6)*sin(e3)*sin(e5)*sin(e6) - 2*I6xy*de1*cos(e3)*cos(e5)*cos(e6)*sin(e2)*sin(e5)*sin(e6) - 2*I6zx*de1*cos(e4)*cos(e5)*cos(e6)*sin(e2)*sin(e3)*sin(e5) + I6xx*de1*cos(e5)*cos(e6)*sin(e2)*sin(e3)*sin(e4)*sin(e6) - I6yy*de1*cos(e5)*cos(e6)*sin(e2)*sin(e3)*sin(e4)*sin(e6) + 2*I6yz*de1*cos(e4)*cos(e5)*sin(e2)*sin(e3)*sin(e5)*sin(e6) + 2*de1*m5*x5*y5*cos(e2)*cos(e3)*cos(e4)*cos(e5)*sin(e5) - de1*m6*y6*z6*cos(e2)*cos(e3)*cos(e6)*sin(e4)*sin(e5) - 2*de1*m5*x5*y5*cos(e4)*cos(e5)*sin(e2)*sin(e3)*sin(e5) - de1*m6*x6*z6*cos(e2)*cos(e3)*sin(e4)*sin(e5)*sin(e6) + de1*m6*y6*z6*cos(e6)*sin(e2)*sin(e3)*sin(e4)*sin(e5) + de1*m6*x6*z6*sin(e2)*sin(e3)*sin(e4)*sin(e5)*sin(e6) + 2*de1*m6*x6*y6*cos(e2)*cos(e3)*cos(e5)*cos(e6)^2*sin(e4) - 2*de1*m6*x6*y6*cos(e5)*cos(e6)^2*sin(e2)*sin(e3)*sin(e4) + de1*m6*x6^2*cos(e2)*cos(e3)*cos(e5)*cos(e6)*sin(e4)*sin(e6) - de1*m6*y6^2*cos(e2)*cos(e3)*cos(e5)*cos(e6)*sin(e4)*sin(e6) - de1*m6*x6^2*cos(e5)*cos(e6)*sin(e2)*sin(e3)*sin(e4)*sin(e6) + de1*m6*y6^2*cos(e5)*cos(e6)*sin(e2)*sin(e3)*sin(e4)*sin(e6) - 2*de1*m6*x6*y6*cos(e2)*cos(e5)*cos(e6)*sin(e3)*sin(e5)*sin(e6) - 2*de1*m6*x6*y6*cos(e3)*cos(e5)*cos(e6)*sin(e2)*sin(e5)*sin(e6) - 2*de1*m6*x6*z6*cos(e4)*cos(e5)*cos(e6)*sin(e2)*sin(e3)*sin(e5) + 2*de1*m6*y6*z6*cos(e4)*cos(e5)*sin(e2)*sin(e3)*sin(e5)*sin(e6) + 2*de1*m6*x6*y6*cos(e2)*cos(e3)*cos(e4)*cos(e5)^2*cos(e6)*sin(e6) - 2*de1*m6*x6*y6*cos(e4)*cos(e5)^2*cos(e6)*sin(e2)*sin(e3)*sin(e6) + 2*de1*m6*x6*z6*cos(e2)*cos(e3)*cos(e4)*cos(e5)*cos(e6)*sin(e5) - 2*de1*m6*y6*z6*cos(e2)*cos(e3)*cos(e4)*cos(e5)*sin(e5)*sin(e6),I6xy*de4*cos(e5)^2 - I6xy*de4 + 2*I6xy*de4*cos(e6)^2 - (I6xx*de4*sin(2*e6))/2 + (I6yy*de4*sin(2*e6))/2 + (I6xx*de5*sin(e5))/2 - (I6yy*de5*sin(e5))/2 - (I6zz*de5*sin(e5))/2 - I6xx*de5*cos(e6)^2*sin(e5) + I6yy*de5*cos(e6)^2*sin(e5) - de4*m6*x6*y6 + (de4*m6*x6^2*sin(2*e6))/2 - (de4*m6*y6^2*sin(2*e6))/2 - 2*I6xy*de4*cos(e5)^2*cos(e6)^2 + I6xy*de1*cos(e2)*sin(e3) + I6xy*de1*cos(e3)*sin(e2) + (I6xx*de2*cos(e4)*sin(e5))/2 + (I6xx*de3*cos(e4)*sin(e5))/2 - (I6yy*de2*cos(e4)*sin(e5))/2 - (I6yy*de3*cos(e4)*sin(e5))/2 + I6yz*de2*cos(e6)*sin(e4) + I6yz*de3*cos(e6)*sin(e4) + I6yz*de6*cos(e6)*sin(e5) - (I6zz*de2*cos(e4)*sin(e5))/2 - (I6zz*de3*cos(e4)*sin(e5))/2 + I6zx*de2*sin(e4)*sin(e6) + I6zx*de3*sin(e4)*sin(e6) + I6zx*de6*sin(e5)*sin(e6) - de5*m6*x6^2*sin(e5) + de5*m6*x6^2*cos(e6)^2*sin(e5) - de5*m6*y6^2*cos(e6)^2*sin(e5) + de4*m6*x6*y6*cos(e5)^2 + 2*de4*m6*x6*y6*cos(e6)^2 + I6yz*de4*cos(e5)*cos(e6)*sin(e5) + I6xy*de2*cos(e5)*sin(e4)*sin(e5) + I6xy*de3*cos(e5)*sin(e4)*sin(e5) - 2*I6xy*de5*cos(e6)*sin(e5)*sin(e6) + I6zx*de4*cos(e5)*sin(e5)*sin(e6) - de2*m6*x6^2*cos(e4)*sin(e5) - de3*m6*x6^2*cos(e4)*sin(e5) - I6xy*de1*cos(e2)*cos(e5)^2*sin(e3) - I6xy*de1*cos(e3)*cos(e5)^2*sin(e2) - 2*I6xy*de1*cos(e2)*cos(e6)^2*sin(e3) - 2*I6xy*de1*cos(e3)*cos(e6)^2*sin(e2) - I6xx*de2*cos(e4)*cos(e6)^2*sin(e5) - I6xx*de3*cos(e4)*cos(e6)^2*sin(e5) + I6xx*de4*cos(e5)^2*cos(e6)*sin(e6) + I6yy*de2*cos(e4)*cos(e6)^2*sin(e5) + I6yy*de3*cos(e4)*cos(e6)^2*sin(e5) - I6yz*de2*cos(e5)^2*cos(e6)*sin(e4) - I6yz*de3*cos(e5)^2*cos(e6)*sin(e4) - I6yy*de4*cos(e5)^2*cos(e6)*sin(e6) - I6zx*de2*cos(e5)^2*sin(e4)*sin(e6) - I6zx*de3*cos(e5)^2*sin(e4)*sin(e6) - I6yz*de1*cos(e2)*cos(e3)*cos(e4)*cos(e6) - I6zx*de1*cos(e2)*cos(e3)*cos(e4)*sin(e6) + (I6xx*de1*cos(e2)*cos(e3)*sin(e4)*sin(e5))/2 + I6xx*de1*cos(e2)*cos(e6)*sin(e3)*sin(e6) + I6xx*de1*cos(e3)*cos(e6)*sin(e2)*sin(e6) - 2*I6xy*de2*cos(e4)*cos(e6)*sin(e5)*sin(e6) - 2*I6xy*de3*cos(e4)*cos(e6)*sin(e5)*sin(e6) - (I6yy*de1*cos(e2)*cos(e3)*sin(e4)*sin(e5))/2 + I6yz*de1*cos(e4)*cos(e6)*sin(e2)*sin(e3) - I6yy*de1*cos(e2)*cos(e6)*sin(e3)*sin(e6) - I6yy*de1*cos(e3)*cos(e6)*sin(e2)*sin(e6) - (I6zz*de1*cos(e2)*cos(e3)*sin(e4)*sin(e5))/2 + I6zx*de1*cos(e4)*sin(e2)*sin(e3)*sin(e6) - (I6xx*de1*sin(e2)*sin(e3)*sin(e4)*sin(e5))/2 + (I6yy*de1*sin(e2)*sin(e3)*sin(e4)*sin(e5))/2 + (I6zz*de1*sin(e2)*sin(e3)*sin(e4)*sin(e5))/2 - 2*de4*m6*x6*y6*cos(e5)^2*cos(e6)^2 - 2*I6xy*de2*cos(e5)*cos(e6)^2*sin(e4)*sin(e5) - 2*I6xy*de3*cos(e5)*cos(e6)^2*sin(e4)*sin(e5) + de1*m6*x6*y6*cos(e2)*sin(e3) + de1*m6*x6*y6*cos(e3)*sin(e2) + de2*m6*y6*z6*cos(e6)*sin(e4) + de3*m6*y6*z6*cos(e6)*sin(e4) + de6*m6*y6*z6*cos(e6)*sin(e5) + de2*m6*x6^2*cos(e4)*cos(e6)^2*sin(e5) + de3*m6*x6^2*cos(e4)*cos(e6)^2*sin(e5) - de4*m6*x6^2*cos(e5)^2*cos(e6)*sin(e6) - de2*m6*y6^2*cos(e4)*cos(e6)^2*sin(e5) - de3*m6*y6^2*cos(e4)*cos(e6)^2*sin(e5) + de4*m6*y6^2*cos(e5)^2*cos(e6)*sin(e6) + de2*m6*x6*z6*sin(e4)*sin(e6) + de3*m6*x6*z6*sin(e4)*sin(e6) + de6*m6*x6*z6*sin(e5)*sin(e6) + 2*I6xy*de1*cos(e2)*cos(e5)^2*cos(e6)^2*sin(e3) + 2*I6xy*de1*cos(e3)*cos(e5)^2*cos(e6)^2*sin(e2) - I6xy*de1*cos(e2)*cos(e3)*cos(e4)*cos(e5)*sin(e5) - I6yz*de1*cos(e2)*cos(e5)*cos(e6)*sin(e3)*sin(e5) - I6yz*de1*cos(e3)*cos(e5)*cos(e6)*sin(e2)*sin(e5) + I6xy*de1*cos(e4)*cos(e5)*sin(e2)*sin(e3)*sin(e5) + I6xx*de2*cos(e5)*cos(e6)*sin(e4)*sin(e5)*sin(e6) + I6xx*de3*cos(e5)*cos(e6)*sin(e4)*sin(e5)*sin(e6) - I6yy*de2*cos(e5)*cos(e6)*sin(e4)*sin(e5)*sin(e6) - I6yy*de3*cos(e5)*cos(e6)*sin(e4)*sin(e5)*sin(e6) - I6zx*de1*cos(e2)*cos(e5)*sin(e3)*sin(e5)*sin(e6) - I6zx*de1*cos(e3)*cos(e5)*sin(e2)*sin(e5)*sin(e6) - de1*m6*x6^2*cos(e2)*cos(e3)*sin(e4)*sin(e5) - de1*m6*x6^2*cos(e2)*cos(e6)*sin(e3)*sin(e6) - de1*m6*x6^2*cos(e3)*cos(e6)*sin(e2)*sin(e6) + de1*m6*y6^2*cos(e2)*cos(e6)*sin(e3)*sin(e6) + de1*m6*y6^2*cos(e3)*cos(e6)*sin(e2)*sin(e6) + I6yz*de1*cos(e2)*cos(e3)*cos(e4)*cos(e5)^2*cos(e6) + I6zx*de1*cos(e2)*cos(e3)*cos(e4)*cos(e5)^2*sin(e6) + de1*m6*x6^2*sin(e2)*sin(e3)*sin(e4)*sin(e5) - I6xx*de1*cos(e2)*cos(e3)*cos(e6)^2*sin(e4)*sin(e5) - I6xx*de1*cos(e2)*cos(e5)^2*cos(e6)*sin(e3)*sin(e6) - I6xx*de1*cos(e3)*cos(e5)^2*cos(e6)*sin(e2)*sin(e6) + I6yy*de1*cos(e2)*cos(e3)*cos(e6)^2*sin(e4)*sin(e5) - I6yz*de1*cos(e4)*cos(e5)^2*cos(e6)*sin(e2)*sin(e3) + I6yy*de1*cos(e2)*cos(e5)^2*cos(e6)*sin(e3)*sin(e6) + I6yy*de1*cos(e3)*cos(e5)^2*cos(e6)*sin(e2)*sin(e6) - I6zx*de1*cos(e4)*cos(e5)^2*sin(e2)*sin(e3)*sin(e6) + de4*m6*y6*z6*cos(e5)*cos(e6)*sin(e5) + I6xx*de1*cos(e6)^2*sin(e2)*sin(e3)*sin(e4)*sin(e5) - I6yy*de1*cos(e6)^2*sin(e2)*sin(e3)*sin(e4)*sin(e5) + de2*m6*x6*y6*cos(e5)*sin(e4)*sin(e5) + de3*m6*x6*y6*cos(e5)*sin(e4)*sin(e5) - 2*de5*m6*x6*y6*cos(e6)*sin(e5)*sin(e6) + de4*m6*x6*z6*cos(e5)*sin(e5)*sin(e6) - de1*m6*x6*y6*cos(e2)*cos(e5)^2*sin(e3) - de1*m6*x6*y6*cos(e3)*cos(e5)^2*sin(e2) - 2*de1*m6*x6*y6*cos(e2)*cos(e6)^2*sin(e3) - 2*de1*m6*x6*y6*cos(e3)*cos(e6)^2*sin(e2) - de2*m6*y6*z6*cos(e5)^2*cos(e6)*sin(e4) - de3*m6*y6*z6*cos(e5)^2*cos(e6)*sin(e4) - de2*m6*x6*z6*cos(e5)^2*sin(e4)*sin(e6) - de3*m6*x6*z6*cos(e5)^2*sin(e4)*sin(e6) + 2*I6xy*de1*cos(e6)*sin(e2)*sin(e3)*sin(e4)*sin(e5)*sin(e6) + 2*de1*m6*x6*y6*cos(e2)*cos(e5)^2*cos(e6)^2*sin(e3) + 2*de1*m6*x6*y6*cos(e3)*cos(e5)^2*cos(e6)^2*sin(e2) - de2*m6*x6^2*cos(e5)*cos(e6)*sin(e4)*sin(e5)*sin(e6) - de3*m6*x6^2*cos(e5)*cos(e6)*sin(e4)*sin(e5)*sin(e6) + de2*m6*y6^2*cos(e5)*cos(e6)*sin(e4)*sin(e5)*sin(e6) + de3*m6*y6^2*cos(e5)*cos(e6)*sin(e4)*sin(e5)*sin(e6) + 2*I6xy*de1*cos(e2)*cos(e3)*cos(e4)*cos(e5)*cos(e6)^2*sin(e5) - de1*m6*y6*z6*cos(e2)*cos(e3)*cos(e4)*cos(e6) - 2*I6xy*de1*cos(e4)*cos(e5)*cos(e6)^2*sin(e2)*sin(e3)*sin(e5) - de1*m6*x6*z6*cos(e2)*cos(e3)*cos(e4)*sin(e6) - 2*de2*m6*x6*y6*cos(e4)*cos(e6)*sin(e5)*sin(e6) - 2*de3*m6*x6*y6*cos(e4)*cos(e6)*sin(e5)*sin(e6) + de1*m6*y6*z6*cos(e4)*cos(e6)*sin(e2)*sin(e3) + de1*m6*x6^2*cos(e2)*cos(e3)*cos(e6)^2*sin(e4)*sin(e5) + de1*m6*x6^2*cos(e2)*cos(e5)^2*cos(e6)*sin(e3)*sin(e6) + de1*m6*x6^2*cos(e3)*cos(e5)^2*cos(e6)*sin(e2)*sin(e6) - de1*m6*y6^2*cos(e2)*cos(e3)*cos(e6)^2*sin(e4)*sin(e5) - de1*m6*y6^2*cos(e2)*cos(e5)^2*cos(e6)*sin(e3)*sin(e6) - de1*m6*y6^2*cos(e3)*cos(e5)^2*cos(e6)*sin(e2)*sin(e6) + de1*m6*x6*z6*cos(e4)*sin(e2)*sin(e3)*sin(e6) - de1*m6*x6^2*cos(e6)^2*sin(e2)*sin(e3)*sin(e4)*sin(e5) + de1*m6*y6^2*cos(e6)^2*sin(e2)*sin(e3)*sin(e4)*sin(e5) - 2*de2*m6*x6*y6*cos(e5)*cos(e6)^2*sin(e4)*sin(e5) - 2*de3*m6*x6*y6*cos(e5)*cos(e6)^2*sin(e4)*sin(e5) - 2*I6xy*de1*cos(e2)*cos(e3)*cos(e6)*sin(e4)*sin(e5)*sin(e6) - de1*m6*x6*y6*cos(e2)*cos(e3)*cos(e4)*cos(e5)*sin(e5) - de1*m6*y6*z6*cos(e2)*cos(e5)*cos(e6)*sin(e3)*sin(e5) 